simulink library "dkc"  (R2021b)
settings: Solver=VariableStepAuto  StartTime=0.0  StopTime=10.0  RelTol=1e-3
undefined symbols (not defined in the file): ENUM_ANTITHEFT_ALARM, ENUM_ANTITHEFT_ARM, ENUM_ANTITHEFT_DISARM, ENUM_ANTITHEFT_WAIT, ENUM_APSSTASYSTEM_DISABLE, ENUM_APSSTASYSTEM_ENABLE, ENUM_APSSTASYSTEM_REMOTEACTIVE, ENUM_BTCONNSTA_CONNECTED, ENUM_BTCONNSTA_DISCONNECTED, ENUM_DKCAuthSta_DECRYPTIONFAIL, ENUM_DKCAuthSta_NORMAL, ENUM_DKCAuthSta_TIMEERROR, ENUM_DKCPCMDHANDING_FORCELIFT, ENUM_DKCPCMDHANDING_LOCK, ENUM_DKCPCMDHANDING_LOCKTGATEFAIL, ENUM_DKCPCMDHANDING_OVER, ENUM_DKCPCMDHANDING_TGATEHANDLE, ENUM_DKCPCMDHANDING_UNLOCK, ENUM_DkeyShowIVI_DEFAULT, ENUM_DkeyShowIVI_INVALID, ENUM_DkeyShowIVI_NFCGREEN, ENUM_DkeyShowIVI_NFCRED, ENUM_GEARACTUALPOSN_N, ENUM_GEARACTUALPOSN_P, ENUM_KEYMISSSTA_DEFAULT, ENUM_KEYMISSSTA_KEYMISS, ENUM_KEYMODE_DAFAULT, ENUM_KEYMODE_INVALID, ENUM_KEYMODE_NFC, ENUM_KEYMODE_UIDBLE, ENUM_KEYMODE_UIDUWB, ENUM_KEYTYPE_NFC, ENUM_KEYTYPE_NOREQ, ENUM_KEYTYPE_UID, ENUM_PARKINGMODE_DISABLE, ENUM_PARKINGMODE_REMOTEFORWARD, ENUM_PARKINGMODE_REMOTEREVERSE, ENUM_PARKINGMODE_STANDBY, ENUM_PCMD_AUTOLOCKJUDGE, ENUM_PCMD_DEFAULT, ENUM_PCMD_NFCDETECT, ENUM_PCMD_PTGJUDGE, ENUM_PCMD_RSSIJUDGELOCK, ENUM_PCMD_TRUNKHAND, ENUM_PCMD_UIDBUTTON, ENUM_PCMD_UWBDETEDT, ENUM_PCMDTOBCM_DEFAULT, ENUM_PCMDTOBCM_FORCELIFT, ENUM_PCMDTOBCM_LOCK, ENUM_PCMDTOBCM_LOCKTGATEFAIL, ENUM_PCMDTOBCM_NFCCOMMAND, ENUM_PCMDTOBCM_REMOTETGATE, ENUM_PCMDTOBCM_TGATEHANDLE, ENUM_PCMDTOBCM_UNLOCK, ENUM_PCMDTOBCM_UWBLOCK, ENUM_PCMDTOBCM_UWBUNLOCK, ENUM_PDKEYPTGAREA_GRAYSPTGZONE, ENUM_PDKEYPTGAREA_PTGZONE, ENUM_PDKEYPTGAREA_SPTGZONE, ENUM_PDKEYPTGAREA_UNAVALIABLE ... (+126)
libraries: simulink x120, hcu_lib x6
(part 2 of 4)

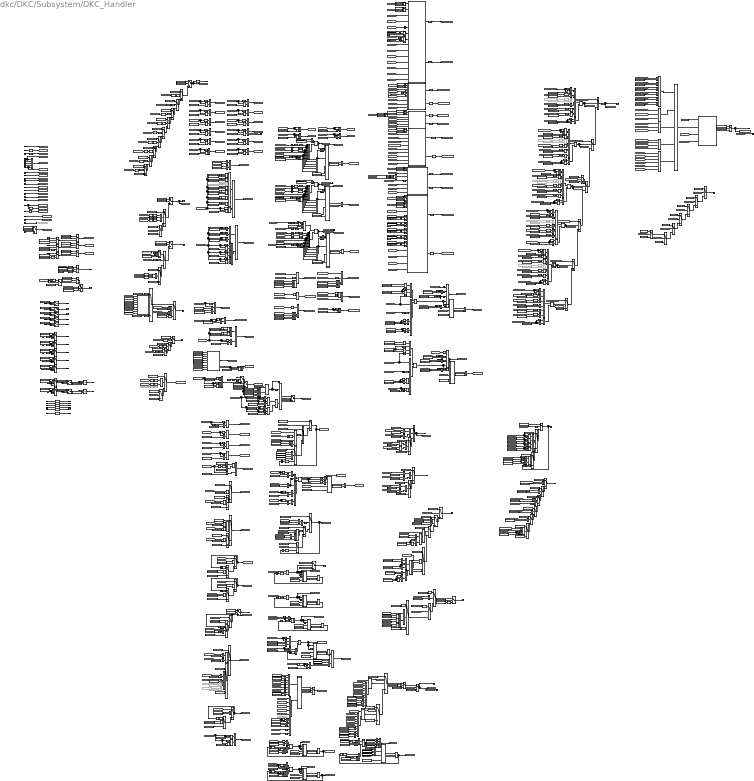
== system dkc/DKC/Subsystem/DKC_Handler ==
  note: % VINP_PDKeyAreaLockUnlock_enum(PE Zone)
      | ENUM_PDKEYRAWLULOCK_UNAVALIABLE = uint8( 0 );
      | ENUM_PDKEYRAWLULOCK_INLOCK = uint8( 1 );
      | ENUM_PDKEYRAWLULOCK_INUNLOCK = uint8( 2 );
      | ENUM_PDKEYRAWLULOCK_RESERVE = uint8( 3 );
      | ENUM_PDKEYRAWLULOCK_OTHERZONE = uint8( 255 );
  note: UWB Detect PDKey PEZone raw (沒有明確狀態一律給UNAVALIABLE)
  note: % VINP_PDKeyAreaLockUnlock_enum(PE Zone)
      | ENUM_PDKEYRAWLULOCK_UNAVALIABLE = uint8( 0 );
      | ENUM_PDKEYRAWLULOCK_INLOCK = uint8( 1 );
      | ENUM_PDKEYRAWLULOCK_INUNLOCK = uint8( 2 );
      | ENUM_PDKEYRAWLULOCK_RESERVE = uint8( 3 );
      | ENUM_PDKEYRAWLULOCK_OTHERZONE = uint8( 255 );
  note: VDKC_UWBXFPP_enum
      | DD File Define:s8
      | Valid Range:-127~127
      | Invalid value:128
  note: VINP_UWBXPower_dB
      | BSW Define:s8
      | Valid Range:-128~126
      | Invalid value:127(0x7F)
  note: VDKC_CoordinateX_enum
      | DD File Define:s16
      | Valid Range:-2550~2550
      | over range:2560(0x1FF)
      | INVALID:-2550(0x000)
  note: VDKC_UWB1Distance_enum
      | DD File Define:u16
      | Valid Range:0~2540
      | Invalid value:2550( 0xFF*10 )
  note: VINP_UWBxDistance_cm
      | BSW Define:u16
      | Valid Range:0~65534
      | Invalid value:65535(0xFFFF)
  note: KeyFobArea
      | KeyFobArea=0: unavailable
      |
      | Bit0 : PS Zone
      | Bit1 : Unlock Zone
      | Bit2 : Lock Zone
      |
      | Bit3 : SPTG Zone
      | Bit4 : PTG Zone
      | Bit5 : Welcome Zone
      | Bit6 : OutWelcome Zone
      | Bit7 : RKE Zone
      | Bit8 : GrayLockZone
      | Bit9 : GrayWelcomeZone
      | Bit10: GrayOutWelcomeZone
      | Bit11: GraySPTGZone
      |
      | 如過只舉PTG相關Flag
      | 輸出匯給出UNAVALIABLE
  note: KeyFobArea_flag change to KeyUWBDetPTGArea_enum
  note: 60s timeout
  note: Wait 60s standby judge
  note: Wait 60 s
  note: 5.5s timeout
  note: Wait 4S+1.5S USER Control Forward/Backward Req Judge
  note: Wait 4+1.5 s
  note: Wait 200ms APM-APS Req Judge
  note: Wait 200ms timeout
  note: UIDBLEButton Requireto RAPS Backward Release
  note: UIDBLEButton Requireto RAPS Forward Release
  note: UIDBLEButton Requireto RAPS Backward Press
  note: UIDBLEButton Requireto RAPS Forward Press
  note: UIDBLEButton Requireto RAPS Start Release
  note: UIDBLEButton Requireto RAPS Start Press
  note: KeyFobArea
      | KeyFobArea=0: unavailable
      | Bit0 : PS Zone
      | Bit1 : Unlock Zone
      | Bit2 : Lock Zone
      | Bit3 : SPTG Zone
      | Bit4 : PTG Zone
      | Bit5 : Welcome Zone
      | Bit6 : OutWelcome Zone
      | Bit7 : RKE Zone
      | Bit8 : GrayLockZone
      | Bit9 : GrayWelcomeZone
      | Bit10: GrayOutWelcomeZone
      | Bit11: GraySPTGZone
      |
      | 如過只舉PTG相關Flag
      | 輸出匯給出UNAVALIABLE
  note: KeyFobArea_flag change to PTGArea Debug
  note: UnavailabletoUnlock request door unlock
  note: RSSI Judge Lock trigger edge
  note: RSSI STRONG >>WEAK
  note: Key mode sta Judge
  note: Key Type Judge
  note: % VDKC_KeyModeSta_enum
      | ENUM_KEYMODE_DAFAULT = uint8( 0 );
      | ENUM_KEYMODE_UIDUWB = uint8( 1 );
      | ENUM_KEYMODE_UIDBLE = uint8( 2 );
      | ENUM_KEYMODE_PHONEUWB = uint8( 3 );
      | ENUM_KEYMODE_PHONEBLE = uint8( 4 );
      | ENUM_KEYMODE_NFC = uint8( 5 );
      | ENUM_KEYMODE_INVALID = uint8( 6 );
  note: % VDKC_FDCPCommandToBCM_enum
      | ENUM_PCMDTOBCM_DEFAULT = uint8( 0 );
      | ENUM_PCMDTOBCM_LOCK = uint8( 1 );
      | ENUM_PCMDTOBCM_UNLOCK = uint8( 2 );
      | ENUM_PCMDTOBCM_REMOTETGATE = uint8( 3 );
      | ENUM_PCMDTOBCM_CARSEARCH = uint8( 4 );
      | ENUM_PCMDTOBCM_LOCKTGATEFAIL = uint8( 5 );
      | ENUM_PCMDTOBCM_TGATEHANDLE = uint8( 6 );
      | ENUM_PCMDTOBCM_FORCELIFT = uint8( 7 );
      | ENUM_PCMDTOBCM_CARSEARCHMUTE = uint8( 8 );
      | ENUM_PCMDTOBCM_NFCCOMMAND = uint8( 9 );
      | ENUM_PCMDTOBCM_UWBLOCK = uint8( 10 );
      | ENUM_PCMDTOBCM_UWBUNLOCK = uint8( 11 );
      | ENUM_PCMDTOBCM_FRONTHOOD = uint8( 12 );
      | ENUM_PCMDTOBCM_CHARGECOVER = uint8( 13 );
      | ENUM_PCMDTOBCM_INVALID = uint8( 15 );
  note: % KDKC_BTConnectSta_enum_ovrdflg
      | % VDKC_BTConnectSta_enum
      | ENUM_BTCONNSTA_DISCONNECTED = uint8( 0 );
      | ENUM_BTCONNSTA_CONNECTED = uint8( 1 );
      | ENUM_BTCONNSTA_CONNECTING = uint8( 2 );
      | ENUM_BTCONNSTA_RESERVE = uint8( 3 );
  note: UID Battery Low Show in IVI
  note: % VDKC_UIDLowPowerSta_enum
      | ENUM_UIDLOWBATSTA_DEFAULT = uint8( 0 );
      | ENUM_UIDLOWBATSTA_LOWBATT = uint8( 1 );
  note: % KDKC_BTConnectSta_enum_ovrdflg
      | % VDKC_BTConnectSta_enum
      | ENUM_BTCONNSTA_DISCONNECTED = uint8( 0 );
      | ENUM_BTCONNSTA_CONNECTED = uint8( 1 );
      | ENUM_BTCONNSTA_CONNECTING = uint8( 2 );
      | ENUM_BTCONNSTA_RESERVE = uint8( 3 );
  note: PDKEY or NFC Card Judge Area in PS
  note: % VDKC_KeyMissSta_enum
      | ENUM_KEYMISSSTA_DEFAULT = uint8( 0 );
      | ENUM_KEYMISSSTA_KEYMISS = uint8( 1 );
  note: % VPMM_PowerSta_enum
      | ENUM_POWERSTA_OFF = uint8( 0 );
      | ENUM_POWERSTA_OFFC = uint8( 1 );
      | ENUM_POWERSTA_OFFA = uint8( 2 );
      | ENUM_POWERSTA_STANDBY = uint8( 3 );
      | ENUM_POWERSTA_ON = uint8( 4 );
      | ENUM_POWERSTA_READY = uint8( 5 );
  note: Fix the Bug of debounce in the DKC P-Command.
  note: WelcomeSta Latch
  note: KeyFobArea
      | KeyFobArea=0: unavailable
      | Bit0 : PS Zone
      | Bit1 : Unlock Zone
      | Bit2 : Lock Zone
      | Bit3 : SPTG Zone
      | Bit4 : PTG Zone
      | Bit5 : Welcome Zone
      | Bit6 : OutWelcome Zone
      | Bit7 : RKE Zone
      | Bit8 : GrayLockZone
      | Bit9 : GrayWelcomeZone
      | Bit10: GrayOutWelcomeZone
      | Bit11: GraySPTGZone
      |
      | 如過只舉PTG相關Flag
      | 輸出匯給出UNAVALIABLE
  note: % VDKC_FDCKeyAreaSPTG_enum
      | % VDKC_KeyAreaSPTGSta_enum
      | % KDKC_KeyUWBDetSPTGArea_enum_ovrdval
      | ENUM_PDKEYSPTGRAW_UNAVALIABLE = uint8( 0 );
      | ENUM_PDKEYSPTGRAW_INTOZONE = uint8( 1 );
      | ENUM_PDKEYSPTGRAW_OUTZONE = uint8( 2 );
      | ENUM_PDKEYSPTGRAW_RESERVE = uint8( 3 );
  note: KeyFobArea_flag change to KeyUWBDetSPTGArea_enum
  note: KeyFobArea
      | KeyFobArea=0: unavailable
      | Bit0 : PS Zone
      | Bit1 : Unlock Zone
      | Bit2 : Lock Zone
      | Bit3 : SPTG Zone
      | Bit4 : PTG Zone
      | Bit5 : Welcome Zone
      | Bit6 : OutWelcome Zone
      | Bit7 : RKE Zone
      | Bit8 : GrayLockZone
      | Bit9 : GrayWelcomeZone
      | Bit10: GrayOutWelcomeZone
      | Bit11: GraySPTGZone
      |
      | 如過只舉PTG相關Flag
      | 輸出匯給出UNAVALIABLE
  note: 5m
  note: KeyFobArea
      | KeyFobArea=0: unavailable
      | Bit0 : PS Zone
      | Bit1 : Unlock Zone
      | Bit2 : Lock Zone
      | Bit3 : SPTG Zone
      | Bit4 : PTG Zone
      | Bit5 : OutPTG Zone
      | Bit6 : Welcome Zone
      | Bit7 : OutWelcome Zone
      | Bit8 : RKE Zone
      | Bit9 : InitDetLockZone (GrayLockZone)
      | Bit10: InitDetWelcomeZone(GrayWelcomeZone)
      | Bit11: InitDetOutWelcomeZone(GrayOutWelcomeZone
  note: PMM change to ready if( Antif==ARM ) , PCmd==FORCELIFT
  note: If the remote app lock during the auto-lock period,the next auto-lock will fail.
  note: If the remote app lock during the auto-lock period,the next auto-lock will fail.
  note: RemoteTG command Rising Judge
  note: Priority4-TrunkHandPCmd
  note: Priority2-TrunkHandPCmd
  note: TRUNKHANSW_PRESS Judge
  note: UIDBLEButton Requireto CHARGECOVER
  note: UIDBLEButton Requireto FRONTHOOD
  note: % VDKC_FDCKeyAreaPTG_enum
      | % VINP_PDKeyAreaPTG_enum
      | % VDKC_KeyAreaPTG_enum
      | % KDKC_KeyUWBDetPTGArea_enum_ovrdval
      | ENUM_PDKEYPTGRAW_UNAVALIABLE = uint8( 0 );
      | ENUM_PDKEYPTGRAW_INTOZONE = uint8( 1 );
      | ENUM_PDKEYPTGRAW_OUTZONE = uint8( 2 );
      | ENUM_PDKEYPTGRAW_RESERVE = uint8( 3 );
  note: KeyFobArea_flag change to KeyUWBDetPTGArea_enum
  note: % KINP_UIDButtonCmd_enum_ovrdval
      | % VHAL_UIDButtonCmd_enum
      | % VINP_UIDButtonCmd_enum
      | ENUM_UIDBUTTON_UNAVALIABLE = uint8( 0 );
      | ENUM_UIDBUTTON_UNLOCK = uint8( 1 );
      | ENUM_UIDBUTTON_LOCK = uint8( 2 );
      | ENUM_UIDBUTTON_FRONTHOOD = uint8( 3 );
      | ENUM_UIDBUTTON_REMOTETAILGATE = uint8( 4 );
      | ENUM_UIDBUTTON_CHARGECOVER = uint8( 5 );
      | ENUM_UIDBUTTON_CARSEARCH = uint8( 6 );
      | ENUM_UIDBUTTON_RAPSSTARTPRESS = uint8( 7 );
      | ENUM_UIDBUTTON_RAPSFORWARDPRESS = uint8( 8 );
      | ENUM_UIDBUTTON_RAPSBACKWARDPRESS = uint8( 9 );
      | ENUM_UIDBUTTON_RAPSSTARTRELEASE = uint8( 10 );
      | ENUM_UIDBUTTON_RAPSFORWARDRELEASE = uint8( 11 );
      | ENUM_UIDBUTTON_RAPSBACKWARRELEASE = uint8( 12 );
  note: UIDBLEButton Requireto CARSEARCH
  note: UIDBLEButton Requireto REMOTETAILGATE
  note: % VDKC_KeyUWBDetArea_enum
      | % KDKC_KeyUWBDetArea_enum_ovrdval
      | ENUM_UWBDET_UNAVALIABLE = uint8( 0 );
      | ENUM_UWBDET_PSZONE = uint8( 1 );
      | ENUM_UWBDET_UNLOCKZONE = uint8( 2 );
      | ENUM_UWBDET_LOCKZONE = uint8( 3 );
      | ENUM_UWBDET_WELCOMEZONE = uint8( 4 );
      | ENUM_UWBDET_OUTWELCOMEZONE = uint8( 5 );
      | ENUM_UWBDET_RKEZONE = uint8( 6 );
      | ENUM_UWBDET_GRAYLOCKZONE = uint8( 7 );
      | ENUM_UWBDET_GRAYWELCOMEZONE = uint8( 8 );
      | ENUM_UWBDET_GRAYOUTWELCOMEZONE = uint8( 9 );
  note: % VINP_PDKeyAreaLockUnlock_enum
      | ENUM_PDKEYRAWLULOCK_UNAVALIABLE = uint8( 0 );
      | ENUM_PDKEYRAWLULOCK_INLOCK = uint8( 1 );
      | ENUM_PDKEYRAWLULOCK_INUNLOCK = uint8( 2 );
      | ENUM_PDKEYRAWLULOCK_RESERVE = uint8( 3 );
  note: % VINP_PDKeyAreaPS_enum(PS Zone)
      | ENUM_PDKEYRAWPS_UNAVALIABLE = uint8( 0 );
      | ENUM_PDKEYRAWPS_INPS = uint8( 1 );
      | ENUM_PDKEYRAWPS_OUTPS = uint8( 2 );
      | ENUM_PDKEYRAWPS_RESERVE = uint8( 3 );
  note: UIDButton change Antitheft state to DISARM
  note: UIDButton AutoLock Judge
  note: UWB Within unLock Zone(3m) Judge(需為明確的unlock zone)
  note: Priority1-UIDButton PCmd
  note: UIDBLEButton Requireto Unlock
  note: UIDBLEButton Requireto Lock
  note: Arbitration Det Area PE Zone
  note: UWB Detect PDKey PEZone raw (沒有明確狀態一律給UNAVALIABLE)
  note: NFCKeyArea change to non-PS zone
  note: Priority3-NFC Detect PCmd
  note: UWB_Detect_PDKey Require to Lock
  note: UWB_Detect_PDKey Require to unLock
  note: NFC change Antitheft state to DISARM
  note: NFCKeyArea change to PS zone
  note: KeyArea change to non-PS zone
  note: UWB Detect PDKey PSZone raw
  note: Power state change from READY or ON to Standby
  note: Power state change to OFFC
  note: Power state change to OFFA
  note: Power state "LEAVE" from READY
  note: Power state change to OFF
  note: Priority6-UWB Detect PCmd
  note: Detect PCommand set Default
  note: NFCJudge_PS_Area
  note: NFCJudgePEZoneSta
  note: % VINP_PDKeyAreaPS_enum(PS Zone)
      | ENUM_PDKEYRAWPS_UNAVALIABLE = uint8( 0 );
      | ENUM_PDKEYRAWPS_INPS = uint8( 1 );
      | ENUM_PDKEYRAWPS_OUTPS = uint8( 2 );
      | ENUM_PDKEYRAWPS_RESERVE = uint8( 3 );
  note: Arbitration Det Area PS Zone
  note: % VINP_PDKeyAreaLockUnlock_enum
      | ENUM_PDKEYRAWLULOCK_UNAVALIABLE = uint8( 0 );
      | ENUM_PDKEYRAWLULOCK_INLOCK = uint8( 1 );
      | ENUM_PDKEYRAWLULOCK_INUNLOCK = uint8( 2 );
      | ENUM_PDKEYRAWLULOCK_RESERVE = uint8( 3 );
  note: % VINP_PDKeyAreaLockUnlock_enum(PE Zone)
      | ENUM_PDKEYRAWLULOCK_UNAVALIABLE = uint8( 0 );
      | ENUM_PDKEYRAWLULOCK_INLOCK = uint8( 1 );
      | ENUM_PDKEYRAWLULOCK_INUNLOCK = uint8( 2 );
      | ENUM_PDKEYRAWLULOCK_RESERVE = uint8( 3 );
  note: Arbitration PCmdtoBCM
  note: Priority5-AutoLock Judge PCmd
  note: NFC AutoLock Judge
  note: % VDKC_KeyUWBDetArea_enum
      | % KDKC_KeyUWBDetArea_enum_ovrdval
      | ENUM_UWBDET_UNAVALIABLE = uint8( 0 );
      | ENUM_UWBDET_PSZONE = uint8( 1 );
      | ENUM_UWBDET_UNLOCKZONE = uint8( 2 );
      | ENUM_UWBDET_LOCKZONE = uint8( 3 );
      | ENUM_UWBDET_WELCOMEZONE = uint8( 4 );
      | ENUM_UWBDET_OUTWELCOMEZONE = uint8( 5 );
      | ENUM_UWBDET_RKEZONE = uint8( 6 );
      | ENUM_UWBDET_GRAYLOCKZONE = uint8( 7 );
      | ENUM_UWBDET_GRAYWELCOMEZONE = uint8( 8 );
      | ENUM_UWBDET_GRAYOUTWELCOMEZONE = uint8( 9 );
  note: % VTQD_GearActualPosn_enum
      | ENUM_GEARACTUALPOSN_P = uint8( 1 );
      | ENUM_GEARACTUALPOSN_R = uint8( 2 );
      | ENUM_GEARACTUALPOSN_N = uint8( 3 );
      | ENUM_GEARACTUALPOSN_D = uint8( 4 );
      | ENUM_GEARACTUALPOSN_INVALID = uint8( 0 );
  note: % VINP_UIDButtonCmd_enum
      | ENUM_UIDBUTTON_UNAVALIABLE = uint8( 0 );
      | ENUM_UIDBUTTON_UNLOCK = uint8( 1 );
      | ENUM_UIDBUTTON_LOCK = uint8( 2 );
      | ENUM_UIDBUTTON_FRONTHOOD = uint8( 3 );
      | ENUM_UIDBUTTON_REMOTETAILGATE = uint8( 4 );
      | ENUM_UIDBUTTON_CHARGECOVER = uint8( 5 );
      | ENUM_UIDBUTTON_CARSEARCH = uint8( 6 );
  note: KeyFobArea_flag change to KeyUWBDetArea_enum
  note: PTG InnerSW Close TimerOut Count Function
  note: TailgateSW2 FallingEdge to close and Dectect UID in PS Zone
  note: TailgateSW2 FallingEdge to close and Dectect UID out PS Zone
  note: Press InnerSW2 after TailgateSW No Close
  note: FallingEdge to close and Dectect UID in PS Zone
  note: Press InnerSW1 or DKC remtailgate Button after TailgateSW No Close
  note: KeyFobArea
      | KeyFobArea=0: unavailable
      | Bit0 : PS Zone
      | Bit1 : Unlock Zone
      | Bit2 : Lock Zone
      | Bit3 : SPTG Zone
      | Bit4 : PTG Zone
      | Bit5 : Welcome Zone
      | Bit6 : OutWelcome Zone
      | Bit7 : RKE Zone
      | Bit8 : GrayLockZone
      | Bit9 : GrayWelcomeZone
      | Bit10: GrayOutWelcomeZone
      | Bit11: GraySPTGZone
      |
      | 如過只舉PTG相關Flag
      | 輸出匯給出UNAVALIABLE
  note: % VDKC_KeyUWBDetArea_enum
      | % KDKC_KeyUWBDetArea_enum_ovrdval
      | ENUM_UWBDET_UNAVALIABLE = uint8( 0 );
      | ENUM_UWBDET_PSZONE = uint8( 1 );
      | ENUM_UWBDET_UNLOCKZONE = uint8( 2 );
      | ENUM_UWBDET_LOCKZONE = uint8( 3 );
      | ENUM_UWBDET_WELCOMEZONE = uint8( 4 );
      | ENUM_UWBDET_OUTWELCOMEZONE = uint8( 5 );
      | ENUM_UWBDET_RKEZONE = uint8( 6 );
      | ENUM_UWBDET_GRAYLOCKZONE = uint8( 7 );
      | ENUM_UWBDET_GRAYWELCOMEZONE = uint8( 8 );
      | ENUM_UWBDET_GRAYOUTWELCOMEZONE = uint8( 9 );
  note: 8m
  note: 10m
  note: 3m
  note: 3-5m
  note: % VDKC_KeyUWBDetArea_enum
      | % KDKC_KeyUWBDetArea_enum_ovrdval
      | ENUM_UWBDET_UNAVALIABLE = uint8( 0 );
      | ENUM_UWBDET_PSZONE = uint8( 1 );
      | ENUM_UWBDET_UNLOCKZONE = uint8( 2 );
      | ENUM_UWBDET_LOCKZONE = uint8( 3 );
      | ENUM_UWBDET_WELCOMEZONE = uint8( 4 );
      | ENUM_UWBDET_OUTWELCOMEZONE = uint8( 5 );
      | ENUM_UWBDET_RKEZONE = uint8( 6 );
      | ENUM_UWBDET_GRAYLOCKZONE = uint8( 7 );
      | ENUM_UWBDET_GRAYWELCOMEZONE = uint8( 8 );
      | ENUM_UWBDET_GRAYOUTWELCOMEZONE = uint8( 9 );
  note: % VDKC_KeyUWBDetArea_enum
      | % KDKC_KeyUWBDetArea_enum_ovrdval
      | ENUM_UWBDET_UNAVALIABLE = uint8( 0 );
      | ENUM_UWBDET_PSZONE = uint8( 1 );
      | ENUM_UWBDET_UNLOCKZONE = uint8( 2 );
      | ENUM_UWBDET_LOCKZONE = uint8( 3 );
      | ENUM_UWBDET_WELCOMEZONE = uint8( 4 );
      | ENUM_UWBDET_OUTWELCOMEZONE = uint8( 5 );
      | ENUM_UWBDET_RKEZONE = uint8( 6 );
      | ENUM_UWBDET_GRAYLOCKZONE = uint8( 7 );
      | ENUM_UWBDET_GRAYWELCOMEZONE = uint8( 8 );
      | ENUM_UWBDET_GRAYOUTWELCOMEZONE = uint8( 9 );
  note: NFC Unlock/lock PCMD Change to NFC-CMD
  note: % VDKC_KeyUWBDetArea_enum
      | % KDKC_KeyUWBDetArea_enum_ovrdval
      | ENUM_UWBDET_UNAVALIABLE = uint8( 0 );
      | ENUM_UWBDET_PSZONE = uint8( 1 );
      | ENUM_UWBDET_UNLOCKZONE = uint8( 2 );
      | ENUM_UWBDET_LOCKZONE = uint8( 3 );
      | ENUM_UWBDET_WELCOMEZONE = uint8( 4 );
      | ENUM_UWBDET_OUTWELCOMEZONE = uint8( 5 );
      | ENUM_UWBDET_RKEZONE = uint8( 6 );
      | ENUM_UWBDET_GRAYLOCKZONE = uint8( 7 );
      | ENUM_UWBDET_GRAYWELCOMEZONE = uint8( 8 );
      | ENUM_UWBDET_GRAYOUTWELCOMEZONE = uint8( 9 );
  note: UWB_Detect_PDKey Require to Welcome mode
  note: LIDA -Green Latch
  note: in unlockZone and unlock during not counter timeout trigger
  note: in unlockZone and unlock during not counter timeout trigger
  note: trigger==0&& reset==1 timer counter=Reset(0)
  note: trigger==0&& reset==1 timer counter=Reset(0)
  note: NFCJudge Auto Leave PS
  note: DKC Allow Sleep Judge
  note: Keep PE,PS Zone State
  note: % KDKC_BTConnectSta_enum_ovrdflg
      | ENUM_BTConnSta_DISCONNECTED = uint8( 0 );
      | ENUM_BTConnSta_CONNECTED = uint8( 1 );
      | ENUM_BTConnSta_CONNECTING = uint8( 2 );
      | ENUM_BTConnSta_RESERVE = uint8( 3 );
  note: on Ready BT Disconnect 10s(key miss Judge)
  note: NFCKeyArea change to PS zone
  note: % VDKC_KeyTypeSta_enum
      | ENUM_KEYTYPE_NOREQ = uint8( 0 );
      | ENUM_KEYTYPE_UID = uint8( 1 );
      | ENUM_KEYTYPE_NFC = uint8( 2 );
      | ENUM_KEYTYPE_PHONE = uint8( 3 );
  note: Antitheft change to ARM
  note: Antitheft change to ARM
  note: NFC change Antitheft state to DISARM
  note: IVI Show NFC Card STA Judge
  note: DrDoor Sta Judge Latch
  note: RSSI_dBm:1Byte
      | Type:s8[-128~127]
      | (0~-100dB) range
      | Initial value:-128
      | Valid Range:0~-100
      | Other Invalid:1~127,-101~-12
  note: % KDKC_BTRSSISampTime_s=init 100ms
  note: BT RSSI Judge UID Area
  note: RSSI_dBm:1Byte
      | Type:s8[-128~127]
      | (0~-100dB) range
      | Initial value:-128
      | Valid Range:0~-100
      | Other Invalid:1~127,-101~-12
      | % VDKC_RSSIJudgeArea_enum
      | ENUM_RSSIAREA_DAFAULT = uint8( 0 );
      | ENUM_RSSIAREA_WEAK = uint8( 1 );
      | ENUM_RSSIAreaSta_STRONG = uint8( 2 );
  note: Judge Unlock Zone Falling edge flg
  note: % VDKC_KeyUWBDetArea_enum
      | % KDKC_KeyUWBDetArea_enum_ovrdval
      | ENUM_UWBDET_UNAVALIABLE = uint8( 0 );
      | ENUM_UWBDET_PSZONE = uint8( 1 );
      | ENUM_UWBDET_UNLOCKZONE = uint8( 2 );
      | ENUM_UWBDET_LOCKZONE = uint8( 3 );
      | ENUM_UWBDET_WELCOMEZONE = uint8( 4 );
      | ENUM_UWBDET_OUTWELCOMEZONE = uint8( 5 );
      | ENUM_UWBDET_RKEZONE = uint8( 6 );
      | ENUM_UWBDET_GRAYLOCKZONE = uint8( 7 );
      | ENUM_UWBDET_GRAYWELCOMEZONE = uint8( 8 );
      | ENUM_UWBDET_GRAYOUTWELCOMEZONE = uint8( 9 );
  note: PCMD_Debug output
  note: % VDKC_RSSISignal_enum
      | ENUM_RSSI_MAX = uint8( 0 );
      | ENUM_RSSI_UNAVAILABLE = uint8( 255 );
  note: % VDKC_UWBDetPTGArea_enum
      | ENUM_PDKEYPTGAREA_UNAVALIABLE = uint8( 0 );
      | ENUM_PDKEYPTGAREA_SPTGZONE = uint8( 1 );
      | ENUM_PDKEYPTGAREA_PTGZONE = uint8( 2 );
      | ENUM_PDKEYPTGAREA_GraySPTGZone = uint8( 3 );
  note: RAPS Active flg
  note: ACC>1.5% =0
      | ACC<1.5% =1
  note: ACC=Active flg=1
      | ACC=OFF flg=0
  note: % VINP_APSStaSystem_enum
      | % VAPS_APSStaSystem_enum
      | ENUM_APSSTASYSTEM_DISABLE = uint8( 0 );
      | ENUM_APSSTASYSTEM_ENABLE = uint8( 1 );
      | ENUM_APSSTASYSTEM_ACTIVE = uint8( 2 );
      | ENUM_APSSTASYSTEM_FAILED = uint8( 3 );
      | ENUM_APSSTASYSTEM_REMOTEACTIVE = uint8( 4 );
  note: % VINP_APSStaSystem_enum
      | % VAPS_APSStaSystem_enum
      | ENUM_APSSTASYSTEM_DISABLE = uint8( 0 );
      | ENUM_APSSTASYSTEM_ENABLE = uint8( 1 );
      | ENUM_APSSTASYSTEM_ACTIVE = uint8( 2 );
      | ENUM_APSSTASYSTEM_FAILED = uint8( 3 );
      | ENUM_APSSTASYSTEM_REMOTEACTIVE = uint8( 4 );
  note: 200s timeout
  note: % VDKC_FDCDKCParkingMode_enum
      | ENUM_PARKINGMODE_DISABLE = uint8( 0 );
      | ENUM_PARKINGMODE_STANDBY = uint8( 1 );
      | ENUM_PARKINGMODE_REMOTEPARKING = uint8( 2 );
      | ENUM_PARKINGMODE_REMOTEFORWARD = uint8( 3 );
      | ENUM_PARKINGMODE_REMOTEREVERSE = uint8( 4 );
  note: DKC Judge Output ParkingMode
  note: % VDKC_DkeyAreaRAPSSta_enum
      | % KDKC_KeyUWBDetRAPSArea_enum_ovrdval
      | ENUM_PDKEYRAPSRAW_UNAVALIABLE = uint8( 0 );
      | ENUM_PDKEYRAPSRAW_INTOZONE = uint8( 1 );
      | ENUM_PDKEYRAPSRAW_OUTZONE = uint8( 2 );
  note: RAPS Detect zone keep judge
  note: % VINP_UWBxDistance_cm
      | ENUM_UWBXDISTANCE_ONCANINVALID = uint16( 2550 );
      | % VINP_UWB1Power_dB
      | ENUM_UWBPOWER_BSWINVALID = int16( 127 );
      | % VDKC_UWBXFPP_enum
      | ENUM_UWBPOWER_ONCANINVALID = int16( 128 );
      | % VINP_UWBpositionX_cm
      | ENUM_UWBPOSX_BSWINVALID = int16( 32767 );
      | % VDKC_CoordinateX_enum
      | ENUM_UWBPOSX_ONCANINVALID = int16( -2550 );
      | ENUM_UWBPOSX_ONCANEXRANGE = int16( 2560 );
      | % VINP_UWBpositionY_cm
      | ENUM_UWBPOSY_ONCANINVALID = int16( 0 );
      | ENUM_UWBPOSY_BSWINVALID = int16( 32767 );
      | ENUM_UWBPOSY_ONCANEXRANGE = int16( -2560 );
  note: UWBxDistance
  note: UWB1Power
  note: % VINP_UWB5RangingSta_enum
      | % VDKC_UWB5Invalid_flg
      | % KINP_UWB5RangingSta_enum_ovrdval
      | ENUM_UWBRANGINGSTA_VALID = uint8( 0 );
      | ENUM_UWBRANGINGSTA_INVALID = uint8( 1 );
      | ENUM_UWBRANGINGSTA_BROKEN = uint8( 2 );
      | ENUM_UWBRANGINGSTA_NOUSED = uint8( 3 );
  note: UWBpositionX/Y
  note: UWB OTHER
  note: Keep Detect unlock area
  note: keep unlockzone to otherzone Judge lock
  task_time_s : Inport
  VINP_NFCLidASta_flg : Inport  Port=2
  VINP_NFCDoorSta_flg : Inport  Port=3
  VINP_DrDoorSW_flg : Inport  Port=4
  VINP_PsDoorSW_flg : Inport  Port=5
  VINP_RRDoorSW_flg : Inport  Port=6
  VINP_RLDoorSW_flg : Inport  Port=7
  VINP_TailgateSW_flg : Inport  Port=8
  VINP_HoodSW_flg : Inport  Port=9
  VBCM_AntitheftSta_enum : Inport  Port=10
  VPMM_PowerSta_enum : Inport  Port=11
  VINP_KeyFobAreaU16_enum : Inport  Port=12
  VINP_UIDButtonCmd_enum : Inport  Port=13
  VINP_VehSpeed_kph : Inport  Port=14
  VTQD_GearActualPosn_enum : Inport  Port=15
  VINP_TrunkHanSW_flg : Inport  Port=16
  VINP_BPPTGInsideSW1Sta_enum : Inport  Port=17
  VINP_BPPTGInsideSW2Sta_enum : Inport  Port=18
  VINP_BrakeSWGPIO_flg : Inport  Port=19
  VTQD_LowIdleAccPedal_flg : Inport  Port=20
  VDKC_CANMsgValidZONEDRFR_flg : Inport  Port=21
  VINP_SeatSW_flg : Inport  Port=22
  VINP_BTConnectSta_enum : Inport  Port=23
  VINP_UIDBatVoltx1000_V : Inport  Port=24
  VINP_DKCBTRSSI_dB : Inport  Port=25
  VINP_FlashJugKeepUnLZone_flg : Inport  Port=26
  VINP_BPPTGExistSta_flg : Inport  Port=27
  VINP_APSStaSystem_enum : Inport  Port=28
  VINP_UWB1Distance_cm : Inport  Port=29
  VINP_UWB2Distance_cm : Inport  Port=30
  VINP_UWB3Distance_cm : Inport  Port=31
  VINP_UWB4Distance_cm : Inport  Port=32
  VINP_UWB5Distance_cm : Inport  Port=33
  VINP_UWB1Power_dB : Inport  Port=34
  VINP_UWB2Power_dB : Inport  Port=35
  VINP_UWB3Power_dB : Inport  Port=36
  VINP_UWB4Power_dB : Inport  Port=37
  VINP_UWB5Power_dB : Inport  Port=38
  VINP_UWBpositionX_cm : Inport  Port=39
  VINP_UWBpositionY_cm : Inport  Port=40
  VINP_UWB1RangingSta_enum : Inport  Port=41
  VINP_UWB2RangingSta_enum : Inport  Port=42
  VINP_UWB3RangingSta_enum : Inport  Port=43
  VINP_UWB4RangingSta_enum : Inport  Port=44
  VINP_UWB5RangingSta_enum : Inport  Port=45
  VINP_UWBRangingON_flg : Inport  Port=46
  Abs : Abs
  AllowSleep_Chart : Stateflow chart  TreatAsAtomicUnit=on
  AutoLock_PCMD_Chart : Stateflow chart  TreatAsAtomicUnit=on
  BTRSSIJudgeArea_Chart : Stateflow chart  TreatAsAtomicUnit=on
  Constant : Constant  Value=ENUM_BTCONNSTA_DISCONNECTED  OutDataTypeStr=uint8
  Constant{1,16,136,138,165,304..305,313,316,417} (10 alike) : Constant  Value=ENUM_UWBDET_UNLOCKZONE
  Constant10 : Constant  Value=ENUM_TRUNKHANSW_RELEASE
  Constant{35,100..101,140} (4 alike) : Constant  Value=KDKC_UnlockCmdDelayTime_s
  Constant102 : Constant  Value=ENUM_UIDBUTTON_LOCK
  Constant{57..59,63..68,72..78,103,108,110..113,142,146,149,196,216..220} (31 alike) : Constant  Value=ENUM_DKCPCMDHANDING_OVER
  Constant{60..61,69..70,98,104..105,144..145,147..148,151,153,178,201,261,264..265,271,274,277,279,281,283,285} (25 alike) : Constant  Value=ENUM_PCMDTOBCM_DEFAULT
  Constant{106,159,202..203,205..207,211..212} (9 alike) : Constant  Value=KDKC_ZONEVaildCmdDelayTime_s
  Constant{62,71,107,109,114} (5 alike) : Constant  Commented=on  Value=ENUM_DKCPCMDHANDING_OVER
  Constant11 : Constant  Value=ENUM_PDKEYPTGRAW_INTOZONE
  Constant{3..4,115..116} (4 alike) : Constant  Value=KDKC_AutoLockTimeout_s
  Constant117 : Constant  Value=KDKC_PSAreaTimeout_s
  Constant{44,47,81,92,99,118,128,150,154..156,191,210,241,246,268..269,272,392} (19 alike) : Constant  Value=ENUM_PDKEYRAWPS_INPS
  Constant119 : Constant  Value=KDKC_PSAreaTimeout_s
  Constant12 : Constant  Value=ENUM_PDKEYPTGRAW_UNAVALIABLE
  Constant{55,87,120,226..228,288,306,314,380..381,424} (12 alike) : Constant  Value=ENUM_UWBDET_UNAVALIABLE
  Constant{121,157,160..162} (5 alike) : Constant  Value=ENUM_PDKEYRAWPS_OUTPS
  Constant{82..84,122,129,152,244,263} (8 alike) : Constant  Value=ENUM_POWERSTA_READY
  Constant123 : Constant  Value=ENUM_ANTITHEFT_DISARM
  Constant124 : Constant  Value=ENUM_POWERSTA_OFFC
  Constant125 : Constant  Value=ENUM_POWERSTA_OFF
  Constant{6,8..9,53,56,91,126,197..198,209} (10 alike) : Constant  Value=ENUM_PCMDTOBCM_UNLOCK
  Constant{46,127,158,163..164,170,177,391,393,418} (10 alike) : Constant  Value=ENUM_PDKEYRAWPS_UNAVALIABLE
  Constant13 : Constant  Value=ENUM_UIDBUTTON_REMOTETAILGATE
  Constant130 : Constant  Value=KDKC_LatchWelcomeModeSta_s
  Constant{23,131,134,180} (4 alike) : Constant  Value=ENUM_UWBDET_WELCOMEZONE
  Constant132 : Constant  Value=ENUM_UWBDET_GRAYOUTWELCOMEZONE
  Constant133 : Constant  Commented=on  Value=ENUM_UWBDET_GRAYLOCKZONE
  Constant135 : Constant  Value=ENUM_POWERSTA_STANDBY
  Constant{2,15,97,137,175,422} (6 alike) : Constant  Value=ENUM_UWBDET_PSZONE
  Constant{22,139,166,181} (4 alike) : Constant  Value=ENUM_UWBDET_LOCKZONE
  Constant14 : Constant  Value=ENUM_UIDBUTTON_CARSEARCH
  Constant{48,54,141,199,204} (5 alike) : Constant  Value=KDKC_LockCmdDelayTime_s
  Constant143 : Constant  Value=ENUM_POWERSTA_ON
  Constant{94,167..168,171..172,419,423} (7 alike) : Constant  Value=ENUM_PDKEYRAWLULOCK_INUNLOCK
  Constant{95,169,173..174,176} (5 alike) : Constant  Value=ENUM_PDKEYRAWLULOCK_INLOCK
  Constant17 : Constant  Value=ENUM_PDKEYSPTGRAW_UNAVALIABLE
  Constant179 : Constant  Value=ENUM_UIDBUTTON_UNLOCK
  Constant18 : Constant  Value=ENUM_PDKEYSPTGRAW_INTOZONE
  Constant182 : Constant  Value=ENUM_UWBDET_GRAYWELCOMEZONE
  Constant{25,183,308,315,426} (5 alike) : Constant  Value=ENUM_UWBDET_GRAYLOCKZONE
  Constant{7,24,90,184} (4 alike) : Constant  Value=ENUM_UWBDET_OUTWELCOMEZONE
  Constant185 : Constant  Value=ENUM_PDKEYWELCOMERAW_UNAVALIABLE
  Constant186 : Constant  Value=ENUM_PDKEYWELCOMERAW_INTOZONE
  Constant187 : Constant  Value=ENUM_UWBDET_GRAYOUTWELCOMEZONE
  Constant188 : Constant  Value=KDKC_LatchWelcomeModeSta_s
  Constant189 : Constant  Value=KDKC_LatchLidADetGreenCard_s
  Constant19 : Constant  Value=ENUM_PDKEYSPTGRAW_OUTZONE
  Constant190 : Constant  Value=ENUM_DkeyShowIVI_NFCGREEN
  Constant192 : Constant  Value=KDKC_LatchLidADetGreenCard_s
  Constant193 : Constant  Value=ENUM_DkeyShowIVI_DEFAULT
  Constant194 : Constant  Value=ENUM_DkeyShowIVI_NFCRED
  Constant{79..80,195,213} (4 alike) : Constant  Value=ENUM_ANTITHEFT_ARM
  Constant20 : Constant  Value=KDKC_KeyUWBDetSPTGArea_enum_ovrdflg
  Constant200 : Constant  Value=ENUM_PCMDTOBCM_NFCCOMMAND
  Constant208 : Constant  Value=ENUM_ANTITHEFT_DISARM
  Constant21 : Constant  Value=KDKC_KeyUWBDetSPTGArea_enum_ovrdval
  Constant214 : Constant  Value=ENUM_DkeyShowIVI_INVALID
  Constant215 : Constant  Value=ENUM_DkeyShowIVI_DEFAULT
  Constant221 : Constant  Value=KDKC_FDCKeyAllowSleep_flg_ovrdflg
  Constant222 : Constant  Value=KDKC_FDCKeyAllowSleep_flg_ovrdval
  Constant{51,223,251,262,335,349,382,425} (8 alike) : Constant  Value=ENUM_BTCONNSTA_CONNECTED
  Constant{40,50,52,224} (4 alike) : Constant  Value=ENUM_PCMDTOBCM_REMOTETGATE
  Constant225 : Constant  Value=KDKC_DKCAllowSleepDelayTime_s
  Constant229 : Constant  Value=KDKC_BTConnectSta_enum_ovrdflg
  Constant230 : Constant  Value=KDKC_BTConnectSta_enum_ovrdval
  Constant{231,318..319,337,353,383..386} (9 alike) : Constant  Value=FALSE
  Constant233 : Constant  Value=ENUM_KEYMISSSTA_KEYMISS
  Constant235 : Constant  Value=ENUM_POWERSTA_ON
  Constant236 : Constant  Value=ENUM_POWERSTA_STANDBY
  Constant237 : Constant  Value=ENUM_POWERSTA_OFFC
  Constant238 : Constant  Value=ENUM_KEYMISSSTA_DEFAULT
  Constant239 : Constant  Value=KDKC_BTDisconJudgeDeb_s
  Constant240 : Constant  Value=KDKC_BTDisconJudgeDeb_s
  Constant242 : Constant  Value=ENUM_KEYMISSSTA_DEFAULT
  Constant{243,347,360,362} (4 alike) : Constant  Value=ENUM_BTCONNSTA_DISCONNECTED
  Constant245 : Constant  Value=ENUM_KEYMISSSTA_KEYMISS
  Constant247 : Constant  Value=KDKC_UIDBTStaBSWInpSW_ovrdflg
  Constant248 : Constant  Value=KDKC_UIDBatVoltx1000_V_ovrdflg
  Constant249 : Constant  Value=KDKC_UIDBatVoltx1000_V_ovrdval
  Constant250 : Constant  Value=ENUM_POWERSTA_OFF
  Constant252 : Constant  Value=ENUM_UIDLOWBATSTA_DEFAULT
  Constant253 : Constant  Value=ENUM_UIDLOWBATSTA_DEFAULT
  Constant254 : Constant  Value=ENUM_UIDLOWBATSTA_LOWBATT
  Constant255 : Constant  Value=KDKC_UIDBatLowVolDeb_cnt
  Constant256 : Constant  Value=KDKC_UIDBatOKVolDeb_cnt
  Constant257 : Constant  Value=KDKC_UIDBatSampInterval_s
  Constant258 : Constant  Value=KDKC_UIDBatSampTotal_cnt
  Constant259 : Constant  Value=KDKC_UIDBatLowVolx1000Thres_V
  Constant26 : Constant  Value=ENUM_PDKEYPTGRAW_INTOZONE
  Constant260 : Constant  Value=KDKC_UIDBatOKVolx1000Thres_V
  Constant266 : Constant  Value=ENUM_KEYTYPE_NOREQ
  Constant267 : Constant  Value=ENUM_KEYTYPE_UID
  Constant27 : Constant  Value=ENUM_PDKEYPTGRAW_OUTZONE
  Constant270 : Constant  Value=ENUM_KEYTYPE_NFC
  Constant273 : Constant  Value=ENUM_KEYMODE_UIDBLE
  Constant275 : Constant  Value=KDKC_DrDoorOpenStaKeep_s
  Constant276 : Constant  Value=ENUM_KEYMODE_DAFAULT
  Constant278 : Constant  Value=ENUM_KEYMODE_NFC
  Constant{28,36,41,43,45,49} (6 alike) : Constant  Value=KDKC_PTGSWCloseTimeout_s
  Constant280 : Constant  Value=ENUM_KEYMODE_DAFAULT
  Constant282 : Constant  Value=ENUM_KEYMODE_DAFAULT
  Constant284 : Constant  Value=ENUM_KEYMODE_UIDUWB
  Constant286 : Constant  Value=ENUM_KEYMODE_INVALID
  Constant287 : Constant  Value=KDKC_DrDoorOpenStaKeep_s
  Constant289 : Constant  Value=KDKC_DKCBTRSSI_dB_ovrdflg
  Constant29 : Constant  Value=ENUM_UIDBUTTON_FRONTHOOD
  Constant290 : Constant  Value=KDKC_DKCBTRSSI_dB_ovrdval
  Constant291 : Constant  Value=ENUM_RSSIAREA_WEAK
  Constant292 : Constant  Value=KDKC_UIDVolBSWtInpSW_ovrdflg
  Constant293 : Constant  Value=3000  OutDataTypeStr=uint16
  Constant294 : Constant  Value=KDKC_UIDRSSIBSWtInpSW_ovrdflg
  Constant295 : Constant  Value=0  OutDataTypeStr=uint16
  Constant296 : Constant  Value=KDKC_JudBTRSSIWeakDeb_cnt
  Constant297 : Constant  Value=KDKC_JudBTRSSIStrongDeb_cnt
  Constant298 : Constant  Value=KDKC_BTRSSISampTime_s
  Constant299 : Constant  Value=TRUE  OutDataTypeStr=uint16
  Constant30 : Constant  Value=ENUM_UIDBUTTON_CHARGECOVER
  Constant300 : Constant  Value=KDKC_JudBTRSSIWeakThres_dB
  Constant301 : Constant  Value=KDKC_JudBTRSSIStrongThres_dB
  Constant302 : Constant  Value=KDKC_StoreUnlockAreaSW_ovrdflg
  Constant303 : Constant  Value=KDKC_StoreUnlockAreaSW_ovrdval
  Constant307 : Constant  Value=KDKC_KeyMissStaSW_ovrdflg
  Constant309 : Constant  Value=KDKC_UnavToUnlReqSW_ovrdflg
  Constant31 : Constant  Value=KDKC_KeyUWBDetArea_enum_ovrdflg
  Constant310 : Constant  Value=KDKC_UnavToUnlReqSW_ovrdval
  Constant311 : Constant  Value=KDKC_KeyMissStaSW_ovrdval  OutDataTypeStr=uint16
  Constant312 : Constant  Value=ENUM_PCMDTOBCM_LOCK
  Constant317 : Constant  Value=ENUM_PCMDTOBCM_LOCK
  Constant32 : Constant  Value=KDKC_KeyUWBDetArea_enum_ovrdval
  Constant320 : Constant  Value=ENUM_PDKEYSPTGRAW_OUTZONE
  Constant321 : Constant  Value=ENUM_PCMD_DEFAULT
  Constant322 : Constant  Value=ENUM_PCMD_RSSIJUDGELOCK
  Constant323 : Constant  Value=ENUM_PCMD_UWBDETEDT
  Constant324 : Constant  Value=ENUM_PCMD_AUTOLOCKJUDGE
  Constant325 : Constant  Value=ENUM_PCMD_PTGJUDGE
  Constant326 : Constant  Value=ENUM_PCMD_NFCDETECT
  Constant327 : Constant  Value=ENUM_PCMD_TRUNKHAND
  Constant328 : Constant  Value=ENUM_PCMD_UIDBUTTON
  Constant329 : Constant  Value=ENUM_UIDBUTTON_RAPSSTARTPRESS
  Constant33 : Constant  Value=KDKC_KeyUWBDetPTGArea_enum_ovrdflg
  Constant330 : Constant  Value=ENUM_PDKEYPTGAREA_UNAVALIABLE
  Constant331 : Constant  Value=ENUM_RSSI_UNAVAILABLE
  Constant332 : Constant  Value=ENUM_PDKEYPTGAREA_PTGZONE
  Constant333 : Constant  Value=ENUM_PDKEYPTGAREA_GRAYSPTGZONE
  Constant334 : Constant  Value=ENUM_PDKEYPTGAREA_SPTGZONE
  Constant336 : Constant  Value=ENUM_RSSI_UNAVAILABLE
  Constant338 : Constant  Value=TRUE
  Constant339 : Constant  Value=TRUE
  Constant34 : Constant  Value=KDKC_KeyUWBDetPTGArea_enum_ovrdval
  Constant340 : Constant  Value=ENUM_RSSI_UNAVAILABLE
  Constant341 : Constant  Value=ENUM_UIDBUTTON_RAPSSTARTRELEASE
  Constant342 : Constant  Value=ENUM_UIDBUTTON_RAPSFORWARDPRESS
  Constant343 : Constant  Value=ENUM_UIDBUTTON_RAPSBACKWARDPRESS
  Constant344 : Constant  Value=ENUM_UIDBUTTON_RAPSFORWARDRELEASE
  Constant345 : Constant  Value=ENUM_UIDBUTTON_RAPSBACKWARRELEASE
  Constant{346,352,364,378} (4 alike) : Constant  Value=ENUM_APSSTASYSTEM_DISABLE
  Constant348 : Constant  Value=ENUM_APSSTASYSTEM_ENABLE
  Constant350 : Constant  Value=KDKC_WaitAPMAPSReqTime_s
  Constant351 : Constant  Value=KDKC_WaitAPMAPSReqTime_s
  Constant354 : Constant  Value=ENUM_PARKINGMODE_DISABLE
  Constant355 : Constant  Value=ENUM_APSSTASYSTEM_REMOTEACTIVE
  Constant356 : Constant  Value=KDKC_WaitAPMJudgUserReqTime_s
  Constant357 : Constant  Value=KDKC_WaitAPMJudgUserReqTime_s
  Constant358 : Constant  Value=ENUM_APSSTASYSTEM_ENABLE
  Constant359 : Constant  Value=ENUM_PARKINGMODE_REMOTEFORWARD
  Constant361 : Constant  Value=ENUM_PARKINGMODE_REMOTEREVERSE
  Constant363 : Constant  Value=ENUM_PARKINGMODE_STANDBY
  Constant365 : Constant  Value=KDKC_DKCStandbyWait60sTime_s
  Constant366 : Constant  Value=KDKC_DKCStandbyWait60sTime_s
  Constant367 : Constant  Value=ENUM_APSSTASYSTEM_ENABLE
  Constant368 : Constant  Value=ENUM_PDKEYRAPSRAW_UNAVALIABLE
  Constant{369,373..376} (5 alike) : Constant  Value=ENUM_PDKEYRAPSRAW_INTOZONE
  Constant37 : Constant  Value=ENUM_PTGINNERSWSTA_PRESS
  Constant370 : Constant  Value=ENUM_PDKEYRAPSRAW_OUTZONE
  Constant371 : Constant  Value=KDKC_KeyUWBDetRAPSArea_enum_ovrdflg
  Constant372 : Constant  Value=KDKC_KeyUWBDetRAPSArea_enum_ovrdval
  Constant377 : Constant  Value=ENUM_PARKINGMODE_STANDBY
  Constant379 : Constant  Value=TRUE
  Constant38 : Constant  Value=ENUM_PTGINNERSWSTA_RELEASE
  Constant387 : Constant  Value=KDKC_APSStaSystem_enum_ovrdflg
  Constant388 : Constant  Value=KDKC_APSStaSystem_enum_ovrdval
  Constant389 : Constant  Value=KDKC_UserReqRAPSLatch_flg_ovrdflg
  Constant39 : Constant  Value=ENUM_PTGINNERSWSTA_PRESS
  Constant390 : Constant  Value=KDKC_UserReqRAPSLatch_flg_ovrdval
  Constant{394..398} (5 alike) : Constant  Value=ENUM_UWBXDISTANCE_ONCANINVALID
  Constant{399,401,403,405,407} (5 alike) : Constant  Value=ENUM_UWBPOWER_BSWINVALID
  Constant{400,402,404,406,408} (5 alike) : Constant  Value=ENUM_UWBPOWER_ONCANINVALID
  Constant409 : Constant  Value=ENUM_UWBPOSX_BSWINVALID
  Constant410 : Constant  Value=ENUM_UWBPOSX_ONCANINVALID
  Constant411 : Constant  Value=ENUM_UWBPOSX_ONCANEXRANGE
  Constant412 : Constant  Value=ENUM_UWBPOSX_ONCANEXRANGE
  Constant413 : Constant  Value=ENUM_UWBPOSY_BSWINVALID
  Constant414 : Constant  Value=ENUM_UWBPOSY_ONCANINVALID
  Constant415 : Constant  Value=ENUM_UWBPOSY_ONCANEXRANGE
  Constant416 : Constant  Value=ENUM_UWBPOSY_ONCANEXRANGE
  Constant42 : Constant  Value=ENUM_PTGINNERSWSTA_RELEASE
  Constant420 : Constant  Value=ENUM_PDKEYRAWLULOCK_OTHERZONE
  Constant421 : Constant  Value=ENUM_PDKEYRAWLULOCK_UNAVALIABLE
  Constant427 : Constant  Commented=on  Value=ENUM_UWBDET_GRAYWELCOMEZONE
  Constant428 : Constant  Commented=on  Value=ENUM_UWBDET_GRAYOUTWELCOMEZONE
  Constant429 : Constant  Value=ENUM_PDKEYRAWLULOCK_OTHERZONE
  Constant430 : Constant  Value=ENUM_PDKEYRAWLULOCK_UNAVALIABLE
  Constant5 : Constant  Value=ENUM_ANTITHEFT_DISARM
  Constant85 : Constant  Value=ENUM_UWBDET_RKEZONE
  Constant86 : Constant  Value=ENUM_UWBDET_GRAYOUTWELCOMEZONE
  Constant88 : Constant  Value=ENUM_UWBDET_GRAYWELCOMEZONE
  Constant89 : Constant  Value=ENUM_UWBDET_RKEZONE
  Constant93 : Constant  Value=ENUM_PCMDTOBCM_LOCK
  Constant96 : Constant  Value=ENUM_POWERSTA_OFFA
  Data Type Conversion{1,8..16,18..40,42,44,46..48,50..52,54..55,57..61,63..72,78..83,85,88..89,97..98,101,121,123,128,136,142..146,148..149} (81 alike) : DataTypeConversion  OutDataTypeStr=uint8
  Data Type Conversion{2..7,45,73..77,84,86..87,90..96,99..100,102..117,119..120,124..126,129,131..132,134..135,147} (51 alike) : DataTypeConversion  OutDataTypeStr=boolean
  Data Type Conversion118 : DataTypeConversion  OutDataTypeStr=uint16
  Data Type Conversion122 : DataTypeConversion
  Data Type Conversion127 : DataTypeConversion  OutDataTypeStr=uint16
  Data Type Conversion130 : DataTypeConversion  OutDataTypeStr=uint16
  Data Type Conversion133 : DataTypeConversion  Commented=on  OutDataTypeStr=boolean
  Data Type Conversion{137..141} (5 alike) : DataTypeConversion  OutDataTypeStr=int16
  Data Type Conversion{17,41,43,49,53,56} (6 alike) : DataTypeConversion  Commented=on  OutDataTypeStr=uint8
  Data Type Conversion62 : DataTypeConversion  OutDataTypeStr=int8
  Detect Change{1..56} (56 alike) : simulink/Logic and Bit Operations/Detect Change  vinit=0  OutDataTypeStr=boolean
  Detect Decrease{,1..20} (21 alike) : simulink/Logic and Bit Operations/Detect Decrease  vinit=0.0  OutDataTypeStr=boolean
  Detect Increase{,1..20,22} (22 alike) : simulink/Logic and Bit Operations/Detect Increase  vinit=0.0  OutDataTypeStr=boolean
  Equal{1..22,24,26,28..37,39..40,42..46,48..49,51..67,69..73,75..78,81..83,85..89,91..103,105..107,109..112,114..129,131,137..138,141..147,149,151..152,156,158,164..165,167,169,171..195,198..199,201..203,205..214,216..217,220..221} (176 alike) : RelationalOperator  Operator===  OutDataTypeStr=boolean  RndMeth=Simplest
  Equal{23,25,27,38,47,79,84,90,104,108,130,132..136,139,148,150,153..155,157,159..163,166,168,170,196..197,200,204,215} (36 alike) : RelationalOperator  Operator=~=  OutDataTypeStr=boolean  RndMeth=Simplest
  Equal{41,50,68,74,80,113,218..219} (8 alike) : RelationalOperator  Commented=on  Operator===  OutDataTypeStr=boolean  RndMeth=Simplest
  Extract Bits : simulink/Logic and Bit Operations/Extract Bits  bitsToExtract=Range of bits  numBits=0  bitIdxRange=[0 0]  outScalingMode=Treat bit field as an integer
  Extract Bits1 : simulink/Logic and Bit Operations/Extract Bits  bitsToExtract=Range of bits  numBits=0  bitIdxRange=[1 1]  outScalingMode=Treat bit field as an integer
  Extract Bits10 : simulink/Logic and Bit Operations/Extract Bits  bitsToExtract=Range of bits  numBits=0  bitIdxRange=[4 4]  outScalingMode=Treat bit field as an integer
  Extract Bits11 : simulink/Logic and Bit Operations/Extract Bits  bitsToExtract=Range of bits  numBits=0  bitIdxRange=[11 11]  outScalingMode=Treat bit field as an integer
  Extract Bits12 : simulink/Logic and Bit Operations/Extract Bits  bitsToExtract=Range of bits  numBits=0  bitIdxRange=[11 11]  outScalingMode=Treat bit field as an integer
  Extract Bits13 : simulink/Logic and Bit Operations/Extract Bits  bitsToExtract=Range of bits  numBits=0  bitIdxRange=[3 3]  outScalingMode=Treat bit field as an integer
  Extract Bits14 : simulink/Logic and Bit Operations/Extract Bits  bitsToExtract=Range of bits  numBits=0  bitIdxRange=[11 11]  outScalingMode=Treat bit field as an integer
  Extract Bits15 : simulink/Logic and Bit Operations/Extract Bits  bitsToExtract=Range of bits  numBits=0  bitIdxRange=[4 4]  outScalingMode=Treat bit field as an integer
  Extract Bits16 : simulink/Logic and Bit Operations/Extract Bits  bitsToExtract=Range of bits  numBits=0  bitIdxRange=[3 3]  outScalingMode=Treat bit field as an integer
  Extract Bits17 : simulink/Logic and Bit Operations/Extract Bits  bitsToExtract=Range of bits  numBits=0  bitIdxRange=[4 4]  outScalingMode=Treat bit field as an integer
  Extract Bits18 : simulink/Logic and Bit Operations/Extract Bits  bitsToExtract=Range of bits  numBits=0  bitIdxRange=[1 1]  outScalingMode=Treat bit field as an integer
  Extract Bits19 : simulink/Logic and Bit Operations/Extract Bits  Commented=on  bitsToExtract=Range of bits  numBits=0  bitIdxRange=[2 2]  outScalingMode=Treat bit field as an integer
  Extract Bits2 : simulink/Logic and Bit Operations/Extract Bits  bitsToExtract=Range of bits  numBits=0  bitIdxRange=[2 2]  outScalingMode=Treat bit field as an integer
  Extract Bits20 : simulink/Logic and Bit Operations/Extract Bits  bitsToExtract=Range of bits  numBits=0  bitIdxRange=[0 0]  outScalingMode=Treat bit field as an integer
  Extract Bits3 : simulink/Logic and Bit Operations/Extract Bits  bitsToExtract=Range of bits  numBits=0  bitIdxRange=[5 5]  outScalingMode=Treat bit field as an integer
  Extract Bits4 : simulink/Logic and Bit Operations/Extract Bits  bitsToExtract=Range of bits  numBits=0  bitIdxRange=[6 6]  outScalingMode=Treat bit field as an integer
  Extract Bits5 : simulink/Logic and Bit Operations/Extract Bits  bitsToExtract=Range of bits  numBits=0  bitIdxRange=[3 3]  outScalingMode=Treat bit field as an integer
  Extract Bits6 : simulink/Logic and Bit Operations/Extract Bits  bitsToExtract=Range of bits  numBits=0  bitIdxRange=[7 7]  outScalingMode=Treat bit field as an integer
  Extract Bits7 : simulink/Logic and Bit Operations/Extract Bits  bitsToExtract=Range of bits  numBits=0  bitIdxRange=[8 8]  outScalingMode=Treat bit field as an integer
  Extract Bits8 : simulink/Logic and Bit Operations/Extract Bits  bitsToExtract=Range of bits  numBits=0  bitIdxRange=[9 9]  outScalingMode=Treat bit field as an integer
  Extract Bits9 : simulink/Logic and Bit Operations/Extract Bits  bitsToExtract=Range of bits  numBits=0  bitIdxRange=[10 10]  outScalingMode=Treat bit field as an integer
  From : From  Commented=on  GotoTag=VINP_BPPTGExistSta_flg
  From{73,83,101,153,185} (5 alike) : From  Commented=on  GotoTag=VDKC_UWBDetPCmdHandSta_enum
  From14 : From  Commented=on  GotoTag=VINP_BPPTGExistSta_flg
  From371 : From  Commented=on  GotoTag=VDKC_UIDButtonUnlock_flg
  From415 : From  Commented=on  GotoTag=VINP_KeyFobAreaU16_enum
  From428 : From  Commented=on  GotoTag=VINP_BPPTGExistSta_flg
  From454 : From  Commented=on  GotoTag=VDKC_KeyUWBDetArea_enum
  From455 : From  Commented=on  GotoTag=VDKC_KeyUWBDetArea_enum
  Goto71 : Goto  Commented=on  GotoTag=VINP_BPPTGExistSta_flg
  Logical Operator{1,38,73,127} (4 alike) : Logic  Inputs=4  AllPortsSameDT=off  OutDataTypeStr=boolean
  Logical Operator{2,5,10,53,55,59,67,74,94..95,97..99,109,114..115,121,138..139,146,150..151,163,165,184,188,206,220..221,223..224} (31 alike) : Logic  Operator=OR  AllPortsSameDT=off  OutDataTypeStr=boolean
  Logical Operator{11..14,16,18,20..21,23,26..27,29..30,32,36,42,44..46,49,51..52,54,56,58,60,63..65,68..71,75,78..80,82..84,86..87,89..90,92..93,100,102..104,106,108,110..111,113,116..117,122..123,132,134,136,140..141,143..145,147..149,153,155..157,159..160,166..173,183,186..187,190..192,199,201,210,212,214,222,225..226} (98 alike) : Logic  AllPortsSameDT=off  OutDataTypeStr=boolean
  Logical Operator{28,31,88,101,105,203} (6 alike) : Logic  Inputs=5  AllPortsSameDT=off  OutDataTypeStr=boolean
  Logical Operator{9,76,96,107,129,137,142} (7 alike) : Logic  Operator=OR  Inputs=4  AllPortsSameDT=off  OutDataTypeStr=boolean
  Logical Operator{37,81,85,112,126,128,131,197} (8 alike) : Logic  Operator=OR  Inputs=3  AllPortsSameDT=off  OutDataTypeStr=boolean
  Logical Operator{3..4,6..7,22,35,39..40,43,47,57,61..62,66,72,118..119,125,133,152,154,158,175..181,185,189,195..196,198,200,204..205,207..209,211,213,216..219,227} (47 alike) : Logic  Operator=NOT  AllPortsSameDT=off  OutDataTypeStr=boolean
  Logical Operator{15,24..25,50,120,135,161..162,164} (9 alike) : Logic  Inputs=3  AllPortsSameDT=off  OutDataTypeStr=boolean
  Logical Operator{17,19,33..34,41,48,77,124,215} (9 alike) : Logic  Operator=OR  Inputs=6  AllPortsSameDT=off  OutDataTypeStr=boolean
  Logical Operator130 : Logic  Operator=OR  Inputs=5  AllPortsSameDT=off  OutDataTypeStr=boolean
  Logical Operator174 : Logic  Inputs=9  AllPortsSameDT=off  OutDataTypeStr=boolean
  Logical Operator182 : Logic  Operator=OR  Inputs=10  AllPortsSameDT=off  OutDataTypeStr=boolean
  Logical Operator193 : Logic  Operator=OR  Inputs=10  AllPortsSameDT=off  OutDataTypeStr=boolean
  Logical Operator194 : Logic  Operator=OR  Inputs=10  AllPortsSameDT=off  OutDataTypeStr=boolean
  Logical Operator202 : Logic  Operator=OR  Inputs=5  AllPortsSameDT=off  OutDataTypeStr=boolean
  Logical Operator8 : Logic  Operator=OR  Inputs=5  AllPortsSameDT=off  OutDataTypeStr=boolean
  Logical Operator91 : Logic  Inputs=6  AllPortsSameDT=off  OutDataTypeStr=boolean
  NFC_PCMD_Chart : Stateflow chart  TreatAsAtomicUnit=on
  PDkeyJudgeBatLowVolt_Chart : Stateflow chart  TreatAsAtomicUnit=on
  PTG_PCMD_Chart : Stateflow chart  TreatAsAtomicUnit=on
  Relational Operator{1..13} (13 alike) : RelationalOperator  OutDataTypeStr=boolean  RndMeth=Simplest
  SR_Latch1 : Subsystem  mask(SR_Latch){}
      mask help: SR latch function.
  SR_Latch10 : Subsystem  mask(SR_Latch){}
      mask help: SR latch function.
  SR_Latch11 : Subsystem  mask(SR_Latch){}
      mask help: SR latch function.
  SR_Latch12 : Subsystem  mask(SR_Latch){}
      mask help: SR latch function.
  SR_Latch13 : Subsystem  mask(SR_Latch){}
      mask help: SR latch function.
  SR_Latch14 : Subsystem  mask(SR_Latch){}
      mask help: SR latch function.
  SR_Latch15 : Subsystem  mask(SR_Latch){}
      mask help: SR latch function.
  SR_Latch16 : Subsystem  mask(SR_Latch){}
      mask help: SR latch function.
  SR_Latch17 : Subsystem  mask(SR_Latch){}
      mask help: SR latch function.
  SR_Latch18 : Subsystem  mask(SR_Latch){}
      mask help: SR latch function.
  SR_Latch19 : Subsystem  mask(SR_Latch){}
      mask help: SR latch function.
  SR_Latch2 : Subsystem  mask(SR_Latch){}
      mask help: SR latch function.
  SR_Latch20 : Subsystem  mask(SR_Latch){}
      mask help: SR latch function.
  SR_Latch21 : Subsystem  mask(SR_Latch){}
      mask help: SR latch function.
  SR_Latch22 : Subsystem  mask(SR_Latch){}
      mask help: SR latch function.
  SR_Latch23 : Subsystem  mask(SR_Latch){}
      mask help: SR latch function.
  SR_Latch24 : Subsystem  mask(SR_Latch){}
      mask help: SR latch function.
  SR_Latch25 : Subsystem  mask(SR_Latch){}
      mask help: SR latch function.
  SR_Latch26 : Subsystem  mask(SR_Latch){}
      mask help: SR latch function.
  SR_Latch3 : hcu_lib/Basic_Blocks/SR_Latch
  SR_Latch4 : Subsystem  mask(SR_Latch){}
      mask help: SR latch function.
  SR_Latch5 : Subsystem  mask(SR_Latch){}
      mask help: SR latch function.
  SR_Latch6 : Subsystem  mask(SR_Latch){}
      mask help: SR latch function.
  SR_Latch7 : hcu_lib/Basic_Blocks/SR_Latch
  SR_Latch8 : Subsystem  mask(SR_Latch){}
      mask help: SR latch function.
  SR_Latch9 : Subsystem  mask(SR_Latch){}
      mask help: SR latch function.
  Switch{,1,10,51,54,63,75..82,99,103,114..115} (18 alike) : Switch  Criteria=u2 > Threshold
  Switch{2..9,11..50,52..53,55..57,60..62,64..74,83..92,94..98,100..102,104..113,132..135} (99 alike) : Switch  Criteria=u2 ~= 0
  Switch{116..120} (5 alike) : Switch  Threshold=2550
  Switch{121..126,129} (7 alike) : Switch  Criteria=u2 ~= 0  Threshold=127
  Switch127 : Switch  Criteria=u2 > Threshold  Threshold=2550
  Switch128 : Switch  Threshold=-2550
  Switch130 : Switch  Criteria=u2 > Threshold  Threshold=2550
  Switch131 : Switch  Threshold=-2550
  Switch93 : Switch  Threshold=-100
  Terminator{,1..5} (6 alike) : Terminator
  Timer1 : Subsystem  mask(Timer){}
      mask help: Timer funcion.
  Timer10 : Subsystem  mask(Timer){}
      mask help: Timer funcion.
  Timer11 : Subsystem  mask(Timer){}
      mask help: Timer funcion.
  Timer12 : Subsystem  mask(Timer){}
      mask help: Timer funcion.
  Timer13 : Subsystem  mask(Timer){}
      mask help: Timer funcion.
  Timer2 : Subsystem  mask(Timer){}
      mask help: Timer funcion.
  Timer3 : hcu_lib/Basic_Blocks/Timer
  Timer4 : hcu_lib/Basic_Blocks/Timer
  Timer5 : Subsystem  mask(Timer){}
      mask help: Timer funcion.
  Timer6 : Subsystem  mask(Timer){}
      mask help: Timer funcion.
  Timer7 : Subsystem  mask(Timer){}
      mask help: Timer funcion.
  Timer8 : Subsystem  mask(Timer){}
      mask help: Timer funcion.
  Timer9 : Subsystem  mask(Timer){}
      mask help: Timer funcion.
  TrunkHanSW_PCMD_Chart : Stateflow chart  TreatAsAtomicUnit=on
  UIDButton_PCMD_Chart : Stateflow chart  TreatAsAtomicUnit=on
  UWB_PCMD_Chart : Stateflow chart  TreatAsAtomicUnit=on
  Unit Delay{,1..17,19..46,49..63,67} (62 alike) : UnitDelay  SampleTime=-1  HasFrameUpgradeWarning=on
  Unit Delay18 : UnitDelay  Commented=on  SampleTime=-1  HasFrameUpgradeWarning=on
  VDKC_FDCPCommandToBCM_enum : Outport
  VDKC_FDCKeyAreaLockUnlock_enum : Outport  Port=2
  VDKC_FDCKeyAreaPS_enum : Outport  Port=3
  VDKC_FDCKeyAreaPTG_enum : Outport  Port=4
  VDKC_FDCKeyAreaSPTG_enum : Outport  Port=5
  VDKC_FDCKeyWelcomeSta_enum : Outport  Port=6
  VDKC_FDCKeyAllowSleep_flg : Outport  Port=7
  VDKC_KeyMissSta_flg : Outport  Port=8
  VDKC_UIDLowPowerSta_flg : Outport  Port=9
  VDKC_KeyModeSta_enum : Outport  Port=10
  VDKC_KeyTypeSta_enum : Outport  Port=11
  VDKC_DkeyShowIVISta_enum : Outport  Port=12
  VDKC_JudgeKeepUnlockZone_flg : Outport  Port=13
  VDKC_OutputPCMDModule_enum : Outport  Port=14
  VDKC_UWBDetArea_enum : Outport  Port=15
  VDKC_BLERSSI_enum : Outport  Port=16
  VDKC_UWBDetPTGArea_enum : Outport  Port=17
  VDKC_UIDBatVolt_enum : Outport  Port=18
  VDKC_DkeyAreaRAPSSta_enum : Outport  Port=19
  VDKC_ParkingModeCmd_enum : Outport  Port=20
  VDKC_UWB1Distance_enum : Outport  Port=21
  VDKC_UWB2Distance_enum : Outport  Port=22
  VDKC_UWB3Distance_enum : Outport  Port=23
  VDKC_UWB4Distance_enum : Outport  Port=24
  VDKC_UWB0Distance_enum : Outport  Port=25
  VDKC_UWB1FPP_enum : Outport  Port=26
  VDKC_UWB2FPP_enum : Outport  Port=27
  VDKC_UWB3FPP_enum : Outport  Port=28
  VDKC_UWB4FPP_enum : Outport  Port=29
  VDKC_UWB0FPP_enum : Outport  Port=30
  VDKC_CoordinateX_enum : Outport  Port=31
  VDKC_CoordinateY_enum : Outport  Port=32
  VDKC_UWB1Invalid_flg : Outport  Port=33
  VDKC_UWB2Invalid_flg : Outport  Port=34
  VDKC_UWB3Invalid_flg : Outport  Port=35
  VDKC_UWB4Invalid_flg : Outport  Port=36
  VDKC_UWB0Invalid_flg : Outport  Port=37
  VDKC_UWBOnOff_flg : Outport  Port=38
  wires:
  Unit Delay46/1 -> UIDButton_PCMD_Chart/5(VDKC_UserReqRAPSLatch_flg)
  [VDKC_UserReqRAPSLatch_flg] -> Unit Delay46/1
  Switch57/1 -> UWB_PCMD_Chart/7(VDKC_UWBDetKeepUnltoOther_flg)
  [VDKC_UWBDetKeepUnltoOther_flg] -> Switch57/1
  [VDKC_UserReqRAPSLatch_flg] -> Logical Operator227/1
  Logical Operator227/1 -> Switch57/2
  Constant231/1 -> Switch57/3
  Logical Operator225/1 -> [VDKC_UWBDetKeepUnltoOther_flg]  "VDKC_UWBDetKeepUnltoOther_flg"
  Equal221/1 -> Logical Operator225/1
  Data Type Conversion149/1 -> Equal221/1
  Unit Delay63/1 -> Data Type Conversion149/1
  Constant423/1 -> Equal221/2
  Logical Operator226/1 -> Logical Operator225/2
  Equal220/1 -> Logical Operator226/2
  Detect Change56/1 -> Logical Operator226/1
  Constant429/1 -> Equal220/2
  [VDKC_UWBDetUnlockKeepSta_enum] -> Unit Delay63/1, Detect Change56/1, Equal220/1
  Equal217/1 -> Logical Operator224/2
  Equal212/1 -> Logical Operator224/1
  Logical Operator224/1 -> Switch132/2
  Constant428/1 -> Equal219/2
  From455/1 -> Equal219/1
  From454/1 -> Equal218/1
  Constant427/1 -> Equal218/2
  Constant426/1 -> Equal217/2
  [VDKC_KeyUWBDetArea_enum] -> Equal217/1
  [VDKC_UWBDetUnLockSta_enum] -> Switch134/1
  Data Type Conversion148/1 -> Switch135/1
  Unit Delay62/1 -> Data Type Conversion148/1
  Constant430/1 -> Switch135/3
  Equal216/1 -> Switch135/2
  Constant425/1 -> Equal216/2
  [VDKC_BTConnectSta_enum] -> Equal216/1
  Switch135/1 -> Switch134/3
  Equal215/1 -> Switch134/2
  [VDKC_KeyUWBDetArea_enum] -> Equal215/1
  Constant424/1 -> Equal215/2
  Switch134/1 -> [VDKC_UWBDetUnlockKeepSta_enum], Unit Delay62/1  "VDKC_UWBDetUnlockKeepSta_enum"
  Constant420/1 -> Switch132/3
  Constant421/1 -> Switch132/1
  [VDKC_KeyUWBDetArea_enum] -> Equal212/1
  Switch132/1 -> Switch133/3
  Switch133/1 -> [VDKC_UWBDetUnLockSta_enum]  "VDKC_UWBDetUnLockSta_enum"
  Constant422/1 -> Equal213/2
  [VDKC_KeyUWBDetArea_enum] -> Equal213/1
  Constant419/1 -> Switch133/1
  Logical Operator223/1 -> Switch133/2
  Equal213/1 -> Logical Operator223/1
  [VDKC_KeyUWBDetArea_enum] -> Equal214/1
  Constant417/1 -> Equal214/2
  Equal214/1 -> Logical Operator223/2
  Constant418/1 -> Equal212/2
  Data Type Conversion147/1 -> VDKC_UWBOnOff_flg/1  "VDKC_UWBOnOff_flg"
  VINP_UWBRangingON_flg/1 -> Data Type Conversion147/1
  Data Type Conversion146/1 -> VDKC_UWB0Invalid_flg/1  "VDKC_UWB0Invalid_flg"
  VINP_UWB5RangingSta_enum/1 -> Data Type Conversion146/1
  Data Type Conversion145/1 -> VDKC_UWB4Invalid_flg/1  "VDKC_UWB4Invalid_flg"
  VINP_UWB4RangingSta_enum/1 -> Data Type Conversion145/1
  Data Type Conversion144/1 -> VDKC_UWB3Invalid_flg/1  "VDKC_UWB3Invalid_flg"
  VINP_UWB3RangingSta_enum/1 -> Data Type Conversion144/1
  Data Type Conversion143/1 -> VDKC_UWB2Invalid_flg/1  "VDKC_UWB2Invalid_flg"
  VINP_UWB2RangingSta_enum/1 -> Data Type Conversion143/1
  Data Type Conversion142/1 -> VDKC_UWB1Invalid_flg/1  "VDKC_UWB1Invalid_flg"
  VINP_UWB1RangingSta_enum/1 -> Data Type Conversion142/1
  Data Type Conversion141/1 -> Equal209/2, Switch125/3
  Data Type Conversion140/1 -> Switch124/3, Equal208/2
  Data Type Conversion139/1 -> Equal207/2, Switch123/3
  Data Type Conversion138/1 -> Switch122/3, Equal206/2
  VINP_UWB1Power_dB/1 -> Data Type Conversion137/1
  Data Type Conversion137/1 -> Equal205/2, Switch121/3
  VINP_UWBpositionY_cm/1 -> Switch129/3, Equal211/2
  Equal211/1 -> Switch129/2
  Constant413/1 -> Equal211/1
  Constant414/1 -> Switch129/1
  Switch129/1 -> Switch130/3, Switch130/2
  Constant415/1 -> Switch130/1
  Switch130/1 -> Switch131/1, Switch131/2
  Constant416/1 -> Switch131/3
  Switch131/1 -> VDKC_CoordinateY_enum/1  "VDKC_CoordinateY_enum"
  Switch128/1 -> VDKC_CoordinateX_enum/1  "VDKC_CoordinateX_enum"
  Constant412/1 -> Switch128/3
  Switch127/1 -> Switch128/2, Switch128/1
  Constant411/1 -> Switch127/1
  Switch126/1 -> Switch127/2, Switch127/3
  Constant410/1 -> Switch126/1
  Constant409/1 -> Equal210/1
  Equal210/1 -> Switch126/2
  VINP_UWBpositionX_cm/1 -> Equal210/2, Switch126/3
  Switch125/1 -> VDKC_UWB0FPP_enum/1  "VDKC_UWB0FPP_enum"
  Switch124/1 -> VDKC_UWB4FPP_enum/1  "VDKC_UWB4FPP_enum"
  Switch123/1 -> VDKC_UWB3FPP_enum/1  "VDKC_UWB3FPP_enum"
  Switch122/1 -> VDKC_UWB2FPP_enum/1  "VDKC_UWB2FPP_enum"
  VINP_UWB5Power_dB/1 -> Data Type Conversion141/1
  Constant408/1 -> Switch125/1
  Equal209/1 -> Switch125/2
  Constant407/1 -> Equal209/1
  Constant405/1 -> Equal208/1
  VINP_UWB4Power_dB/1 -> Data Type Conversion140/1
  Equal208/1 -> Switch124/2
  Constant406/1 -> Switch124/1
  Constant404/1 -> Switch123/1
  Equal207/1 -> Switch123/2
  VINP_UWB3Power_dB/1 -> Data Type Conversion139/1
  Constant403/1 -> Equal207/1
  Constant401/1 -> Equal206/1
  VINP_UWB2Power_dB/1 -> Data Type Conversion138/1
  Equal206/1 -> Switch122/2
  Constant402/1 -> Switch122/1
  Switch121/1 -> VDKC_UWB1FPP_enum/1  "VDKC_UWB1FPP_enum"
  Constant400/1 -> Switch121/1
  Equal205/1 -> Switch121/2
  Constant399/1 -> Equal205/1
  Switch120/1 -> VDKC_UWB0Distance_enum/1  "VDKC_UWB0Distance_enum"
  Switch119/1 -> VDKC_UWB4Distance_enum/1  "VDKC_UWB4Distance_enum"
  Switch118/1 -> VDKC_UWB3Distance_enum/1  "VDKC_UWB3Distance_enum"
  Switch117/1 -> VDKC_UWB2Distance_enum/1  "VDKC_UWB2Distance_enum"
  Constant398/1 -> Switch120/1
  VINP_UWB5Distance_cm/1 -> Switch120/2, Switch120/3
  VINP_UWB4Distance_cm/1 -> Switch119/2, Switch119/3
  Constant397/1 -> Switch119/1
  Constant396/1 -> Switch118/1
  VINP_UWB3Distance_cm/1 -> Switch118/2, Switch118/3
  VINP_UWB2Distance_cm/1 -> Switch117/2, Switch117/3
  Constant395/1 -> Switch117/1
  Switch116/1 -> VDKC_UWB1Distance_enum/1  "VDKC_UWB1Distance_enum"
  Constant394/1 -> Switch116/1
  VINP_UWB1Distance_cm/1 -> Switch116/2, Switch116/3
  Constant393/1 -> Equal204/2
  [VDKC_UWBDetPSZoneKeepSta_enum] -> Equal204/1
  Equal204/1 -> Logical Operator222/2
  Equal25/1 -> Logical Operator222/1
  Logical Operator222/1 -> Logical Operator25/3
  Equal24/1 -> Logical Operator221/2
  Constant392/1 -> Equal203/2
  [VDKC_UWBDetPSZoneKeepSta_enum] -> Equal203/1
  [VDKC_UWBDetPSZoneKeepSta_enum] -> Equal24/1
  Logical Operator221/1 -> Logical Operator24/3
  Constant46/1 -> Equal24/2
  Equal203/1 -> Logical Operator221/1
  Logical Operator220/1 -> Logical Operator45/2
  Equal202/1 -> Logical Operator220/2
  Constant391/1 -> Equal202/2
  [VDKC_UWBDetPSZoneKeepSta_enum] -> Equal202/1
  SR_Latch21/1(latched) -> Switch115/3
  Switch115/1 -> [VDKC_UserReqRAPSLatch_flg]
  Constant389/1 -> Switch115/2
  Constant390/1 -> Switch115/1
  Constant388/1 -> Switch114/1
  VINP_APSStaSystem_enum/1 -> Switch114/3
  Constant387/1 -> Switch114/2
  Switch114/1 -> [VDKC_APSStaSystem_enum]  "VDKC_APSStaSystem_enum"
  Unit Delay59/1 -> Logical Operator182/10
  Unit Delay57/1 -> Logical Operator182/9
  Unit Delay55/1 -> Logical Operator182/8
  Equal185/1 -> Logical Operator182/7
  Logical Operator183/1 -> Logical Operator182/6
  Switch113/1 -> UWB_PCMD_Chart/8(VDKC_UnavToUnlReqUnlock_flg)
  Constant386/1 -> Switch113/3
  Logical Operator219/1 -> Switch113/2
  [VDKC_UserReqRAPSLatch_flg] -> Logical Operator219/1
  [VDKC_UnavToUnlReqUnlock_flg] -> Switch113/1
  Switch112/1 -> UWB_PCMD_Chart/6(VDKC_UIDDetRSSIChgToLock_flg)
  [VDKC_UIDDetRSSIChgToLock_flg] -> Switch112/1
  [VDKC_UserReqRAPSLatch_flg] -> Logical Operator218/1
  Logical Operator218/1 -> Switch112/2
  Constant385/1 -> Switch112/3
  Switch111/1 -> UWB_PCMD_Chart/5(VDKC_UWBDetReqtoUnlock_flg)
  Constant384/1 -> Switch111/3
  Logical Operator217/1 -> Switch111/2
  [VDKC_UserReqRAPSLatch_flg] -> Logical Operator217/1
  [VDKC_UWBDetAreaChaToUnlock_flg] -> Switch111/1
  Switch110/1 -> UWB_PCMD_Chart/4(VDKC_UWBDetReqtoLock_flg)
  [VDKC_UWBDetAreaChangeToLock_flg] -> Switch110/1
  [VDKC_UserReqRAPSLatch_flg] -> Logical Operator216/1
  Logical Operator216/1 -> Switch110/2
  Constant383/1 -> Switch110/3
  [VDKC_RPAStandbyTcTrig_flg] -> Logical Operator215/6
  [VDKC_WaitUserReqTrgT_flg] -> Logical Operator215/5
  [VDKC_WaitAPMReqEnTrgT_flg] -> Logical Operator215/4
  [VDKC_UIDForWPressLacth_flg] -> Logical Operator215/3
  [VDKC_UIDBackWPressLacth_flg] -> Logical Operator215/2
  [VDKC_UserReqRAPSLatch_flg] -> Logical Operator215/1
  Switch102/1 -> Switch101/3
  Logical Operator215/1 -> Logical Operator130/5  "VDKC_DKCRAPSTimerActive_flg"
  [VDKC_UserReqRAPSLatch_flg] -> Unit Delay61/1
  Unit Delay61/1 -> Logical Operator214/2
  Logical Operator214/1 -> Switch109/2
  Equal201/1 -> Logical Operator214/1
  [VDKC_DkeyRAPSAreaRaw_enum] -> Switch108/1
  Switch104/1 -> [VDKC_DkeyRAPSAreaRaw_enum]  "VDKC_DkeyRAPSAreaRaw_enum"
  Data Type Conversion136/1 -> Switch109/1
  Unit Delay60/1 -> Data Type Conversion136/1
  Constant380/1 -> Switch109/3
  Constant382/1 -> Equal201/2
  [VDKC_BTConnectSta_enum] -> Equal201/1
  Switch109/1 -> Switch108/3
  Equal200/1 -> Switch108/2
  [VDKC_KeyUWBDetArea_enum] -> Equal200/1
  Constant381/1 -> Equal200/2
  Switch108/1 -> Unit Delay60/1, Switch103/3  "VDKC_UWBDetRAPSZoneKeep_enum"
  Constant337/1 -> Switch107/3
  [VDKC_UIDButtonFrontHood_flg] -> Switch107/1
  Logical Operator213/1 -> Switch107/2
  [VDKC_UserReqRAPSLatch_flg] -> Logical Operator213/1
  Switch107/1 -> UIDButton_PCMD_Chart/6(VDKC_UIDButtonFrontHood_flg)
  Logical Operator212/1 -> Switch84/2
  Logical Operator211/1 -> Logical Operator212/2
  Constant379/1 -> Logical Operator212/1
  [VDKC_UserReqRAPSLatch_flg] -> Logical Operator211/1
  Logical Operator209/1 -> Logical Operator210/2
  Logical Operator210/1 -> Switch85/2
  Constant339/1 -> Logical Operator210/1
  [VDKC_UserReqRAPSLatch_flg] -> Logical Operator209/1
  [VDKC_UIDButtonBackWRelease_flg] -> Logical Operator208/1
  [VDKC_UIDButtonForWRelease_flg] -> Logical Operator207/1
  Logical Operator208/1 -> Logical Operator203/5
  Logical Operator207/1 -> Logical Operator203/4
  [VDKC_UIDButtonBackWRelease_flg] -> Logical Operator202/5
  [VDKC_UIDButtonForWRelease_flg] -> Logical Operator202/4
  Logical Operator181/1 -> Logical Operator174/8
  Logical Operator180/1 -> Logical Operator174/7
  Logical Operator179/1 -> Logical Operator174/6
  Logical Operator178/1 -> Logical Operator174/5
  Logical Operator177/1 -> Logical Operator174/4
  Logical Operator176/1 -> Logical Operator174/3
  Equal199/1 -> Logical Operator174/2
  Equal195/1 -> Logical Operator174/9
  [VDKC_APSStaSystem_enum] -> Equal199/1
  Constant378/1 -> Equal199/2
  [VDKC_ParkingModeCmd_enum] -> Terminator5/1
  [VDKC_UIDButtonStartRelease_flg] -> Terminator4/1
  Constant377/1 -> Switch106/3
  Switch101/1 -> Switch106/1
  Equal198/1 -> Switch106/2
  Constant376/1 -> Equal198/2
  [VDKC_DkeyAreaRAPSSta_enum] -> Equal198/1
  Switch106/1 -> Switch94/1
  Constant375/1 -> Equal197/2
  [VDKC_DkeyAreaRAPSSta_enum] -> Equal197/1
  Equal197/1 -> Logical Operator194/10
  Equal196/1 -> Logical Operator193/10
  [VDKC_DkeyAreaRAPSSta_enum] -> Equal196/1
  Constant374/1 -> Equal196/2
  Constant373/1 -> Equal195/2
  [VDKC_DkeyAreaRAPSSta_enum] -> Equal195/1
  Data Type Conversion135/1 -> Logical Operator206/2
  [VINP_KeyFobAreaU16_enum] -> Extract Bits18/1
  Extract Bits18/1 -> Data Type Conversion135/1
  Data Type Conversion134/1 -> Logical Operator206/1
  Logical Operator206/1 -> Switch104/2
  Switch103/1 -> [VDKC_DkeyAreaRAPSSta_enum], VDKC_DkeyAreaRAPSSta_enum/1  "VDKC_DkeyAreaRAPSSta_enum"
  Constant370/1 -> Switch105/1
  Constant368/1 -> Switch105/3
  [VINP_KeyFobAreaU16_enum] -> Switch105/2
  Switch105/1 -> Switch104/3
  Constant369/1 -> Switch104/1
  Extract Bits20/1 -> Data Type Conversion134/1
  [VINP_KeyFobAreaU16_enum] -> Extract Bits20/1
  Constant372/1 -> Switch103/1
  Constant371/1 -> Switch103/2
  Extract Bits19/1 -> Data Type Conversion133/1
  From415/1 -> Extract Bits19/1
  [VDKC_UIDButtonBackWPress_flg] -> Logical Operator205/1
  Logical Operator205/1 -> Logical Operator203/2
  Logical Operator204/1 -> Logical Operator203/1
  [VDKC_UIDButtonForWPress_flg] -> Logical Operator204/1
  Logical Operator203/1 -> Timer13/1(trigger), [VDKC_RPAStandbyTcTrig_flg]  "VDKC_RPAStandbyTcTrig_flg"
  Logical Operator202/1 -> Timer13/2(reset)
  [VDKC_UIDButtonForWPress_flg] -> Logical Operator202/2
  [VDKC_UIDButtonBackWPress_flg] -> Logical Operator202/3
  Logical Operator198/1 -> Logical Operator202/1
  [VDKC_RPAWait60sReqTout_flg] -> Unit Delay59/1
  Equal194/1 -> Logical Operator197/3
  [VDKC_APSStaSystem_enum] -> Equal194/1
  Constant364/1 -> Equal194/2
  [VDKC_UserReqRAPSLatch_flg] -> Logical Operator200/1
  Logical Operator200/1 -> Logical Operator197/2
  Data Type Conversion132/1 -> Logical Operator197/1
  Logical Operator197/1 -> SR_Latch26/2(reset)
  [task_time_s] -> Timer13/3(Ts)
  Constant365/1 -> Timer13/4(max_time)
  SR_Latch26/1(latched) -> Logical Operator198/1, Logical Operator203/3
  Constant366/1 -> Relational Operator13/2
  Timer13/1(time) -> Relational Operator13/1
  Unit Delay58/1 -> Data Type Conversion132/1
  Relational Operator13/1 -> [VDKC_RPAWait60sReqTout_flg], Unit Delay58/1  "VDKC_RPAWait60sReqTout_flg"
  Logical Operator199/1 -> SR_Latch26/1(set)
  [VDKC_UserReqRAPSLatch_flg] -> Logical Operator199/1
  Equal193/1 -> Logical Operator201/2
  Detect Increase22/1 -> Logical Operator201/1
  Constant367/1 -> Equal193/2
  [VDKC_APSStaSystem_enum] -> Equal193/1, Detect Increase22/1
  Logical Operator201/1 -> Logical Operator199/2
  Constant363/1 -> Switch102/3
  Logical Operator196/1 -> Logical Operator194/9
  [VDKC_UserReqRAPSLatch_flg] -> Logical Operator196/1
  [VDKC_AnyDoorSta_flg] -> Logical Operator194/8
  [VDKC_AnyDoorSta_flg] -> Logical Operator193/8
  [VDKC_UserReqRAPSLatch_flg] -> Logical Operator195/1
  Logical Operator195/1 -> Logical Operator193/9
  Logical Operator194/1 -> SR_Latch25/2(reset)  "VDKC_UIDBackWReset_flg"
  [VDKC_UIDButtonBackWRelease_flg] -> Logical Operator194/1
  [VDKC_UIDButtonUnlock_flg] -> Logical Operator194/2
  [VDKC_UIDButtonLock_flg] -> Logical Operator194/3
  [VDKC_UIDButtonForWPress_flg] -> Logical Operator194/4
  [VDKC_UIDButtonStartPress_flg] -> Logical Operator194/5
  [VDKC_BTConnectSta_enum] -> Equal192/1
  Constant362/1 -> Equal192/2
  Equal192/1 -> Logical Operator194/7
  [VDKC_UIDButtonCarSearch_flg] -> Logical Operator194/6
  [VDKC_UIDButtonBackWPress_flg] -> SR_Latch25/1(set)
  Constant361/1 -> Switch102/1
  SR_Latch25/1(latched) -> Switch102/2, [VDKC_UIDBackWPressLacth_flg]  "VDKC_UIDBackWPressLacth_flg"
  [VDKC_UIDButtonCarSearch_flg] -> Logical Operator193/6
  Equal191/1 -> Logical Operator193/7
  Constant360/1 -> Equal191/2
  [VDKC_BTConnectSta_enum] -> Equal191/1
  [VDKC_UIDButtonStartPress_flg] -> Logical Operator193/5
  [VDKC_UIDButtonBackWPress_flg] -> Logical Operator193/4
  [VDKC_UIDButtonLock_flg] -> Logical Operator193/3
  [VDKC_UIDButtonUnlock_flg] -> Logical Operator193/2
  [VDKC_UIDButtonForWRelease_flg] -> Logical Operator193/1
  Logical Operator193/1 -> SR_Latch24/2(reset)  "VDKC_UIDForWReset_flg"
  SR_Latch24/1(latched) -> [VDKC_UIDForWPressLacth_flg], Switch101/2  "VDKC_UIDForWPressLacth_flg"
  [VDKC_UIDButtonForWPress_flg] -> SR_Latch24/1(set)
  Constant359/1 -> Switch101/1
  [VDKC_WaitAPMJuUserReqTout_flg] -> Unit Delay57/1
  Logical Operator192/1 -> Logical Operator190/2
  [VDKC_APSStaSystem_enum] -> Detect Increase20/1, Equal189/1
  Constant358/1 -> Equal189/2
  Detect Increase20/1 -> Logical Operator192/1
  Equal189/1 -> Logical Operator192/2
  [VDKC_UserReqRAPSLatch_flg] -> Logical Operator190/1
  Logical Operator190/1 -> SR_Latch22/1(set)
  Relational Operator11/1 -> [VDKC_WaitAPMJuUserReqTout_flg], Unit Delay56/1  "VDKC_WaitAPMJuUserReqTout_flg"
  Unit Delay56/1 -> Data Type Conversion131/1
  Timer11/1(time) -> Relational Operator11/1
  Constant357/1 -> Relational Operator11/2
  Logical Operator189/1 -> Timer11/2(reset)
  SR_Latch22/1(latched) -> Logical Operator189/1, Timer11/1(trigger), [VDKC_WaitUserReqTrgT_flg]  "VDKC_WaitUserReqTrgT_flg"
  Constant356/1 -> Timer11/4(max_time)
  [task_time_s] -> Timer11/3(Ts)
  Logical Operator188/1 -> SR_Latch22/2(reset)
  Data Type Conversion131/1 -> Logical Operator188/1
  [VDKC_APSStaSystem_enum] -> Detect Increase19/1, Equal190/1
  Constant355/1 -> Equal190/2
  Detect Increase19/1 -> Logical Operator191/1
  Equal190/1 -> Logical Operator191/2
  Logical Operator191/1 -> Logical Operator188/2
  Constant354/1 -> Switch94/3
  Switch94/1 -> VDKC_ParkingModeCmd_enum/1, [VDKC_ParkingModeCmd_enum]  "VDKC_ParkingModeCmd_enum"
  Constant353/1 -> Data Type Conversion130/1
  Data Type Conversion130/1 -> Switch100/3
  Data Type Conversion127/1 -> Switch100/1
  Switch100/1 -> VDKC_UIDBatVolt_enum/1  "VDKC_UIDBatVolt_enum"
  Equal188/1 -> Switch100/2
  Constant349/1 -> Equal188/2
  [VDKC_BTConnectSta_enum] -> Equal188/1
  [VDKC_UserReqRAPSLatch_flg] -> Switch94/2
  [VDKC_WaitAPMReqTimeout_flg] -> Unit Delay55/1
  Logical Operator187/1 -> Logical Operator184/2
  Equal187/1 -> Logical Operator187/2
  Detect Increase17/1 -> Logical Operator187/1
  Constant348/1 -> Equal187/2
  [VDKC_APSStaSystem_enum] -> Equal187/1, Detect Increase17/1
  Data Type Conversion129/1 -> Logical Operator184/1
  Logical Operator184/1 -> SR_Latch23/2(reset)
  Equal186/1 -> Logical Operator186/2
  Constant352/1 -> Equal186/2
  [VDKC_APSStaSystem_enum] -> Equal186/1
  [task_time_s] -> Timer12/3(Ts)
  Constant350/1 -> Timer12/4(max_time)
  SR_Latch23/1(latched) -> Timer12/1(trigger), [VDKC_WaitAPMReqEnTrgT_flg], Logical Operator185/1  "VDKC_WaitAPMReqEnTrgT_flg"
  Logical Operator185/1 -> Timer12/2(reset)
  Constant351/1 -> Relational Operator12/2
  Timer12/1(time) -> Relational Operator12/1
  Unit Delay54/1 -> Data Type Conversion129/1
  Relational Operator12/1 -> Unit Delay54/1, [VDKC_WaitAPMReqTimeout_flg]  "VDKC_WaitAPMReqTimeout_flg"
  [VDKC_UserReqRAPSLatch_flg] -> Detect Increase18/1
  Detect Increase18/1 -> Logical Operator186/1
  Logical Operator186/1 -> SR_Latch23/1(set)
  [VDKC_BTConnectSta_enum] -> Equal185/1
  Constant347/1 -> Equal185/2
  Constant346/1 -> Equal183/2
  Equal183/1 -> Logical Operator183/2
  Detect Decrease19/1 -> Logical Operator183/1
  [VDKC_APSStaSystem_enum] -> Detect Decrease19/1, Equal183/1
  [VDKC_UIDButtonLock_flg] -> Logical Operator182/5
  [VINP_HoodSW_flg] -> Logical Operator182/2
  [VINP_TailgateSW_flg] -> Logical Operator182/1
  [VINP_BrakeSWSta_flg] -> Logical Operator182/4
  [VDKC_ACCSWSta_flg] -> Logical Operator182/3
  Logical Operator182/1 -> SR_Latch21/2(reset)  "VDKC_RAPStopTrigger_flg"
  Logical Operator174/1 -> SR_Latch21/1(set)  "VDKC_UserReqRAPTrigger_flg"
  [VDKC_UIDButtonStartPress_flg] -> Logical Operator174/1
  [VINP_SeatSW_flg] -> Logical Operator181/1
  [VDKC_ACCSWSta_flg] -> Logical Operator180/1
  [VINP_BrakeSWSta_flg] -> Logical Operator179/1
  [VINP_HoodSW_flg] -> Logical Operator178/1
  [VINP_TailgateSW_flg] -> Logical Operator177/1
  [VDKC_AnyDoorSta_flg] -> Logical Operator176/1
  Logical Operator175/1 -> [VDKC_ACCSWSta_flg]  "VDKC_ACCSWSta_flg"
  VTQD_LowIdleAccPedal_flg/1 -> Logical Operator175/1
  VINP_HoodSW_flg/1 -> [VINP_HoodSW_flg]
  Logical Operator173/1 -> [VDKC_UIDButtonBackWRelease_flg]  "VDKC_UIDButtonBackWRelease_flg"
  Equal181/1 -> Logical Operator173/2
  Detect Change55/1 -> Logical Operator173/1
  Constant345/1 -> Equal181/2
  [VDKC_UIDBLEBatton_Cmd] -> Detect Change55/1, Equal181/1
  [VDKC_UIDBLEBatton_Cmd] -> Equal180/1, Detect Change54/1
  Constant344/1 -> Equal180/2
  Detect Change54/1 -> Logical Operator172/1
  Equal180/1 -> Logical Operator172/2
  Logical Operator172/1 -> [VDKC_UIDButtonForWRelease_flg]  "VDKC_UIDButtonForWRelease_flg"
  [VDKC_UIDBLEBatton_Cmd] -> Equal179/1, Detect Change53/1
  Constant343/1 -> Equal179/2
  Detect Change53/1 -> Logical Operator171/1
  Equal179/1 -> Logical Operator171/2
  Logical Operator171/1 -> [VDKC_UIDButtonBackWPress_flg]  "VDKC_UIDButtonBackWPress_flg"
  Logical Operator170/1 -> [VDKC_UIDButtonForWPress_flg]  "VDKC_UIDButtonForWPress_flg"
  Equal178/1 -> Logical Operator170/2
  Detect Change52/1 -> Logical Operator170/1
  Constant342/1 -> Equal178/2
  [VDKC_UIDBLEBatton_Cmd] -> Detect Change52/1, Equal178/1
  Logical Operator169/1 -> [VDKC_UIDButtonStartRelease_flg]  "VDKC_UIDButtonStartRelease_flg"
  Equal177/1 -> Logical Operator169/2
  Detect Change51/1 -> Logical Operator169/1
  Constant341/1 -> Equal177/2
  [VDKC_UIDBLEBatton_Cmd] -> Detect Change51/1, Equal177/1
  [VDKC_UIDBLEBatton_Cmd] -> Equal176/1, Detect Change50/1
  Constant329/1 -> Equal176/2
  Detect Change50/1 -> Logical Operator168/1
  Equal176/1 -> Logical Operator168/2
  Logical Operator168/1 -> [VDKC_UIDButtonStartPress_flg]  "VDKC_UIDButtonStartPress_flg"
  Switch93/1 -> Switch99/3
  Constant331/1 -> Switch93/3
  Data Type Conversion123/1 -> Switch93/1
  Abs/1 -> Data Type Conversion123/1
  [VDKC_DKCBTRSSI_dB] -> Abs/1, Switch93/2
  [VDKC_DKCBTRSSI_dB] -> Switch99/2
  Constant340/1 -> Switch99/1
  [VDKC_UIDBatVoltx1000_V] -> Data Type Conversion127/1
  Constant338/1 -> Switch83/2
  Constant336/1 -> Switch95/3
  Switch99/1 -> Switch95/1
  Switch95/1 -> VDKC_BLERSSI_enum/1  "VDKC_BLERSSI_enum"
  Equal175/1 -> Switch95/2
  [VDKC_BTConnectSta_enum] -> Equal175/1
  Constant335/1 -> Equal175/2
  Constant334/1 -> Switch96/1
  Constant332/1 -> Switch97/1
  Constant333/1 -> Switch98/1
  Switch96/1 -> VDKC_UWBDetPTGArea_enum/1  "VDKC_UWBDetPTGArea_enum"
  Switch98/1 -> Switch97/3
  Switch97/1 -> Switch96/3
  [VINP_KeyFobAreaU16_enum] -> Extract Bits16/1
  Extract Bits16/1 -> Data Type Conversion124/1
  Constant330/1 -> Switch98/3
  Data Type Conversion124/1 -> Switch96/2
  [VINP_KeyFobAreaU16_enum] -> Extract Bits17/1
  Extract Bits17/1 -> Data Type Conversion125/1
  Data Type Conversion125/1 -> Switch97/2
  Extract Bits14/1 -> Data Type Conversion126/1
  [VINP_KeyFobAreaU16_enum] -> Extract Bits14/1
  Data Type Conversion126/1 -> Switch98/2
  Data Type Conversion122/1 -> VDKC_UWBDetArea_enum/1  "VDKC_UWBDetArea_enum"
  Switch86/1 -> VDKC_OutputPCMDModule_enum/1  "VDKC_OutputPCMDModule_enum"
  Constant328/1 -> Switch86/1
  Constant327/1 -> Switch87/1
  Constant326/1 -> Switch88/1
  Constant325/1 -> Switch89/1
  Constant324/1 -> Switch90/1
  Constant323/1 -> Switch92/3
  Constant322/1 -> Switch92/1
  Constant321/1 -> Switch91/3
  [VDKC_UIDDetRSSIChgToLock_flg] -> Switch92/2
  Switch92/1 -> Switch91/1
  Switch91/1 -> Switch90/3
  Switch90/1 -> Switch89/3
  Switch89/1 -> Switch88/3
  Switch88/1 -> Switch87/3
  Switch87/1 -> Switch86/3
  [VDKC_UWBDetCmdLatch_flg] -> Switch91/2
  [VDKC_AutoLockCmdLatch_flg] -> Switch90/2
  [VDKC_PTGPCmdLatch_flg] -> Switch89/2
  [VDKC_NFCDetPCmdLatch_flg] -> Switch88/2
  [VDKC_TrunkHanPCmdLatch_flg] -> Switch87/2
  [VDKC_UIDButPCmdLatch_flg] -> Switch86/2
  VINP_DKCBTRSSI_dB/1 -> Switch78/1
  VINP_UIDBatVoltx1000_V/1 -> Switch76/1
  VINP_BTConnectSta_enum/1 -> Switch77/1
  PDkeyJudgeBatLowVolt_Chart/1(VDKC_UIDBatLowVolt_flg) -> Switch65/2  "VDKC_UIDBatLowVolt_flg"
  Logical Operator138/1 -> SR_Latch17/2(reset)
  Logical Operator140/1 -> Logical Operator138/1
  [VDKC_BTConnectSta_enum] -> Equal151/1, Detect Change42/1
  Constant262/1 -> Equal151/2
  Detect Change42/1 -> Logical Operator140/1
  Equal151/1 -> Logical Operator140/2
  Logical Operator133/1 -> Timer9/2(reset)
  [VDKC_FDCKeyAllowSleep_flg] -> Terminator2/1
  Switch51/1 -> [VDKC_FDCKeyAllowSleep_flg], VDKC_FDCKeyAllowSleep_flg/1  "VDKC_FDCKeyAllowSleep_flg"
  AllowSleep_Chart/1(VDKC_FDCKeyAllowSleep_flg) -> Switch51/3
  Constant221/1 -> Switch51/2
  Constant222/1 -> Switch51/1
  Logical Operator130/1 -> AllowSleep_Chart/2(VDKC_FDCDKCTimerActive_flg)  "VDKC_FDCDKCTimerActive_flg"
  Constant225/1 -> AllowSleep_Chart/1(KDKC_DKCAllowSleepDelayTime_s)
  [VPMM_PowerSta_enum] -> AllowSleep_Chart/4(VPMM_PowerSta_enum)
  [task_time_s] -> AllowSleep_Chart/3(task_time_s)
  Logical Operator129/1 -> Logical Operator130/4  "VDKC_DKCOtherTimerActive_flg"
  Logical Operator128/1 -> Logical Operator130/3  "VDKC_DKCAutoJudgTimerActive_flg"
  Logical Operator126/1 -> Logical Operator130/2  "VDKC_DKCTGTimerActive_flg"
  Logical Operator124/1 -> Logical Operator130/1  "VDKC_DKCCmdHandTimerActive_flg"
  [VDKC_LidADetGreenCardLatch4s_flg] -> Logical Operator129/2
  [VDKC_UWBDetChgWelcomeLatch_flg] -> Logical Operator129/1
  [VDKC_AutoLeavePSTimerLatch_flg] -> Logical Operator128/3
  [VDKC_UIDAutoLockTimerLatch_flg] -> Logical Operator128/2
  [VDKC_NFCAutoLockTimerLatch_flg] -> Logical Operator128/1
  [VDKC_RemTGCmdTimerLatch_flg] -> Logical Operator126/3
  [VDKC_InnerSW1TimerLatch_flg] -> Logical Operator126/2
  [VDKC_InnerSW2TimerLatch_flg] -> Logical Operator126/1
  Equal133/1 -> Logical Operator124/3
  Equal134/1 -> Logical Operator124/4
  Equal135/1 -> Logical Operator124/5
  Equal136/1 -> Logical Operator124/6
  Constant220/1 -> Equal136/2
  [VDKC_AutoLockPCmdHandSta_enum] -> Equal136/1
  Constant219/1 -> Equal135/2
  [VDKC_UWBDetPCmdHandSta_enum] -> Equal135/1
  Constant218/1 -> Equal134/2
  [VDKC_PTGPCmdHandSta_enum] -> Equal134/1
  Constant217/1 -> Equal133/2
  [VDKC_NFCDetPCmdHandSta_enum] -> Equal133/1
  Constant216/1 -> Equal132/2
  [VDKC_TrunkHanPCmdHandSta_enum] -> Equal132/1
  Equal132/1 -> Logical Operator124/2
  [VDKC_UIDButtonPCmdHandSta_enum] -> Equal130/1
  Constant196/1 -> Equal130/2
  Equal130/1 -> Logical Operator124/1
  Logical Operator60/1 -> [VDKC_PMMChgToReady_flg]  "VDKC_PMMChgToReady_flg"
  Unit Delay42/1 -> Data Type Conversion113/1
  [VDKC_UIDButtJudgeAutoLock_flg] -> Unit Delay42/1
  Unit Delay41/1 -> Data Type Conversion112/1
  [VDKC_NFCDetJudgeAutoLock_flg] -> Unit Delay41/1
  Logical Operator56/1 -> Logical Operator76/3
  Logical Operator110/1 -> Logical Operator76/4
  Switch47/1 -> AutoLock_PCMD_Chart/1(KDKC_LockCmdDelayTime_s)
  [VDKC_CANMsgValidZONEDRFR_flg] -> Switch47/2
  Constant48/1 -> Switch47/3
  Constant207/1 -> Switch47/1
  Switch49/1 -> UWB_PCMD_Chart/1(KDKC_LockCmdDelayTime_s)
  Switch50/1 -> UWB_PCMD_Chart/2(KDKC_UnlockCmdDelayTime_s)
  [VDKC_CANMsgValidZONEDRFR_flg] -> Switch50/2
  Constant140/1 -> Switch50/3
  Constant212/1 -> Switch50/1
  Constant211/1 -> Switch49/1
  Constant141/1 -> Switch49/3
  [VDKC_CANMsgValidZONEDRFR_flg] -> Switch49/2
  Switch46/1 -> PTG_PCMD_Chart/1(KDKC_LockCmdDelayTime_s)
  Constant159/1 -> Switch46/1
  Constant54/1 -> Switch46/3
  [VDKC_CANMsgValidZONEDRFR_flg] -> Switch46/2
  Switch45/1 -> NFC_PCMD_Chart/2(KDKC_UnlockCmdDelayTime_s)
  Constant106/1 -> Switch45/1
  Constant35/1 -> Switch45/3
  [VDKC_CANMsgValidZONEDRFR_flg] -> Switch45/2
  Switch44/1 -> TrunkHanSW_PCMD_Chart/1(KDKC_UnlockCmdDelayTime_s)
  [VDKC_CANMsgValidZONEDRFR_flg] -> Switch43/2
  Constant204/1 -> Switch43/3
  Constant205/1 -> Switch43/1
  Switch43/1 -> NFC_PCMD_Chart/1(KDKC_LockCmdDelayTime_s)
  Constant206/1 -> Switch44/1
  Constant101/1 -> Switch44/3
  [VDKC_CANMsgValidZONEDRFR_flg] -> Switch44/2
  [VDKC_CANMsgValidZONEDRFR_flg] -> Switch42/2
  Constant100/1 -> Switch42/3
  Constant203/1 -> Switch42/1
  Switch42/1 -> UIDButton_PCMD_Chart/2(KDKC_UnlockCmdDelayTime_s)
  Switch41/1 -> UIDButton_PCMD_Chart/1(KDKC_LockCmdDelayTime_s)
  Constant202/1 -> Switch41/1
  Constant199/1 -> Switch41/3
  [VDKC_CANMsgValidZONEDRFR_flg] -> Switch41/2
  VDKC_CANMsgValidZONEDRFR_flg/1 -> [VDKC_CANMsgValidZONEDRFR_flg]
  Equal55/1 -> Logical Operator101/5
  Equal54/1 -> Logical Operator101/4
  Equal49/1 -> Logical Operator31/5
  Equal48/1 -> Logical Operator31/4
  Equal51/1 -> Logical Operator31/3
  Equal44/1 -> Logical Operator88/5
  Equal43/1 -> Logical Operator88/4
  Equal81/1 -> Logical Operator88/3
  Equal40/1 -> Logical Operator28/5
  Equal39/1 -> Logical Operator28/4
  Equal42/1 -> Logical Operator28/3
  Equal35/1 -> Logical Operator105/5
  Equal34/1 -> Logical Operator105/4
  Equal75/1 -> Logical Operator105/3
  Switch26/1 -> Switch27/3
  Constant178/1 -> Switch26/3
  Switch27/1 -> Switch12/3
  Logical Operator35/1 -> Logical Operator127/3
  Constant198/1 -> Equal63/2
  Equal63/1 -> Logical Operator35/1
  [VDKC_UIDButtonPCmdToBCMRAW_enum] -> Unit Delay40/1
  Unit Delay40/1 -> Data Type Conversion85/1
  Data Type Conversion85/1 -> Equal63/1
  Logical Operator7/1 -> Logical Operator73/3
  Equal33/1 -> Logical Operator7/1
  [VDKC_UIDButtonPCmdToBCMRAW_enum] -> Unit Delay32/1
  Unit Delay32/1 -> Data Type Conversion72/1
  Constant197/1 -> Equal33/2
  Data Type Conversion72/1 -> Equal33/1
  Logical Operator57/1 -> Logical Operator73/1
  SR_Latch3/1 -> Logical Operator43/1, Logical Operator73/4
  Data Type Conversion71/1 -> Equal4/1
  Constant6/1 -> Equal4/2
  Equal4/1 -> Logical Operator6/1
  [VDKC_FDCPCommandToBCM_enum] -> Unit Delay10/1
  Unit Delay10/1 -> Data Type Conversion71/1
  Unit Delay9/1 -> Data Type Conversion69/1
  [VDKC_FDCPCommandToBCM_enum] -> Unit Delay9/1
  Equal10/1 -> Logical Operator72/1
  Constant126/1 -> Equal10/2
  Data Type Conversion69/1 -> Equal10/1
  Constant201/1 -> Switch19/3
  Constant200/1 -> Switch19/1
  [VDKC_NFCDetPCmdToBCMRAW_enum] -> Switch19/2
  Switch19/1 -> Switch25/1
  Logical Operator111/1 -> Logical Operator9/4
  Logical Operator127/1 -> Timer1/1(trigger), [VDKC_UIDAutoLockTimerLatch_flg]  "VDKC_UIDAutoLockTimerLatch_flg"
  Logical Operator125/1 -> Logical Operator127/1
  [VDKC_UWBDetWithinUnlockZone_flg] -> Logical Operator125/1
  Logical Operator72/1 -> Logical Operator73/2
  Data Type Conversion87/1 -> Logical Operator114/2
  [VINP_KeyFobAreaU16_enum] -> Extract Bits12/1
  Extract Bits12/1 -> Data Type Conversion87/1
  Data Type Conversion86/1 -> Logical Operator114/1
  Logical Operator114/1 -> Switch18/2
  Extract Bits15/1 -> Data Type Conversion86/1
  [VINP_KeyFobAreaU16_enum] -> Extract Bits15/1
  Data Type Conversion84/1 -> Switch2/2
  Switch1/1 -> VDKC_FDCKeyAreaSPTG_enum/1  "VDKC_FDCKeyAreaSPTG_enum"
  Constant19/1 -> Switch18/1
  Constant17/1 -> Switch18/3
  Switch2/1 -> Switch1/3
  Switch18/1 -> Switch2/3
  Constant21/1 -> Switch1/1
  Constant20/1 -> Switch1/2
  Extract Bits13/1 -> Data Type Conversion84/1
  [VINP_KeyFobAreaU16_enum] -> Extract Bits13/1
  Data Type Conversion45/1 -> Logical Operator112/3
  [VINP_KeyFobAreaU16_enum] -> Extract Bits11/1
  Extract Bits11/1 -> Data Type Conversion45/1
  VINP_BPPTGInsideSW1Sta_enum/1 -> [VINP_BPPTGInsideSW1Sta_enum]
  VINP_BPPTGInsideSW2Sta_enum/1 -> [VINP_BPPTGInsideSW2Sta_enum]
  [VTQD_GearActualPosn_enum] -> TrunkHanSW_PCMD_Chart/7(VDKC_GearActualPosn_enum)
  Equal59/1 -> Logical Operator77/1
  Equal122/1 -> Logical Operator77/2
  [VPMM_PowerSta_enum] -> Detect Change34/1, Equal117/1
  Constant84/1 -> Equal117/2
  Equal117/1 -> Logical Operator111/2
  Detect Change34/1 -> Logical Operator111/1
  Detect Change18/1 -> Logical Operator110/1
  [VPMM_PowerSta_enum] -> Equal60/1, Detect Change18/1
  Equal60/1 -> Logical Operator110/2
  Constant83/1 -> Equal60/2
  Detect Increase9/1 -> AutoLock_PCMD_Chart/4(VDKC_PMMChgToReady_flg)
  [VDKC_PMMChgToReady_flg] -> Detect Increase9/1
  Constant82/1 -> Equal58/2
  Equal58/1 -> Logical Operator60/2
  [VPMM_PowerSta_enum] -> Detect Change17/1, Equal58/1
  Detect Change17/1 -> Logical Operator60/1
  Data Type Conversion70/1 -> Equal30/1
  Data Type Conversion68/1 -> Equal5/1
  Data Type Conversion66/1 -> Detect Change7/1, Equal20/1
  Unit Delay12/1 -> Data Type Conversion66/1
  Data Type Conversion64/1 -> Detect Change8/1, Equal19/1
  Unit Delay3/1 -> Data Type Conversion64/1
  Data Type Conversion63/1 -> Detect Change9/1, Equal26/1
  Unit Delay7/1 -> Data Type Conversion63/1
  Constant80/1 -> Equal56/2
  [VBCM_AntitheftSta_enum] -> Detect Change16/1, Equal56/1
  Detect Change16/1 -> Logical Operator58/1
  Equal56/1 -> Logical Operator58/2
  Equal31/1 -> Logical Operator56/2
  Detect Change12/1 -> Logical Operator56/1
  [VBCM_AntitheftSta_enum] -> Equal31/1, Detect Change12/1
  Constant79/1 -> Equal31/2
  Logical Operator55/1 -> Timer3/2
  Logical Operator43/1 -> Logical Operator55/1
  Constant56/1 -> Equal30/2
  Equal30/1 -> Logical Operator55/2
  [VDKC_UIDButtonPCmdToBCMRAW_enum] -> Unit Delay1/1
  Unit Delay1/1 -> Data Type Conversion70/1
  [VDKC_UWBDetWithinUnlockZone_flg] -> Logical Operator57/1
  Unit Delay11/1 -> Data Type Conversion68/1
  [VDKC_UIDButtJudgeAutoLock_flg] -> Detect Increase2/1
  [VDKC_NFCDetJudgeAutoLock_flg] -> Detect Increase7/1
  [VDKC_PTGPCmdHandSta_enum] -> Data Type Conversion61/1
  Constant78/1 -> Equal55/2
  Data Type Conversion61/1 -> Equal55/1
  Data Type Conversion60/1 -> Equal54/1
  Constant77/1 -> Equal54/2
  [VDKC_TrunkHanPCmdHandSta_enum] -> Data Type Conversion60/1
  [VDKC_TrunkHanPCmdHandSta_enum] -> Data Type Conversion58/1
  Constant75/1 -> Equal52/2
  Data Type Conversion58/1 -> Equal52/1
  Data Type Conversion59/1 -> Equal53/1
  Constant76/1 -> Equal53/2
  [VDKC_PTGPCmdHandSta_enum] -> Data Type Conversion59/1
  Equal52/1 -> Logical Operator91/5
  Equal53/1 -> Logical Operator91/6
  Switch12/1 -> Switch25/3
  [VDKC_TrunkHanPCmdHandSta_enum] -> Data Type Conversion23/1
  Constant74/1 -> Equal49/2
  Data Type Conversion23/1 -> Equal49/1
  Data Type Conversion21/1 -> Equal48/1
  Constant73/1 -> Equal48/2
  [VDKC_UIDButtonPCmdHandSta_enum] -> Data Type Conversion21/1
  [VDKC_AutoLockPCmdHandSta_enum] -> Data Type Conversion57/1
  From83/1 -> Data Type Conversion56/1
  [VDKC_NFCDetPCmdHandSta_enum] -> Data Type Conversion24/1
  Constant68/1 -> Equal45/2
  Data Type Conversion24/1 -> Equal45/1
  Detect Decrease2/1 -> Logical Operator30/1
  Equal46/1 -> Logical Operator30/2
  Constant69/1 -> Equal46/2
  [VDKC_PTGPCmdToBCMRAW_enum] -> Detect Decrease2/1, Equal46/1
  Logical Operator30/1 -> SR_Latch10/2(reset)
  Equal45/1 -> Logical Operator31/2
  Logical Operator31/1 -> SR_Latch10/1(set)
  Logical Operator32/1 -> Logical Operator31/1
  Equal47/1 -> Logical Operator32/2
  Detect Change14/1 -> Logical Operator32/1
  Constant70/1 -> Equal47/2
  [VDKC_PTGPCmdToBCMRAW_enum] -> Equal47/1, Detect Change14/1
  SR_Latch10/1(latched) -> [VDKC_PTGPCmdLatch_flg], Switch12/2
  [VDKC_PTGPCmdToBCMRAW_enum] -> Switch12/1
  Data Type Conversion56/1 -> Equal50/1
  Constant71/1 -> Equal50/2
  Constant72/1 -> Equal51/2
  Data Type Conversion57/1 -> Equal51/1
  Switch25/1 -> Switch11/3
  [VDKC_TrunkHanPCmdHandSta_enum] -> Data Type Conversion19/1
  Constant66/1 -> Equal43/2
  Data Type Conversion19/1 -> Equal43/1
  Data Type Conversion20/1 -> Equal44/1
  Constant67/1 -> Equal44/2
  [VDKC_PTGPCmdHandSta_enum] -> Data Type Conversion20/1
  Data Type Conversion18/1 -> Equal42/1
  Constant63/1 -> Equal42/2
  Constant62/1 -> Equal41/2
  Data Type Conversion17/1 -> Equal41/1
  [VDKC_TrunkHanPCmdToBCMRAW_enum] -> Switch11/1
  SR_Latch9/1(latched) -> Switch11/2, [VDKC_TrunkHanPCmdLatch_flg]
  [VDKC_TrunkHanPCmdToBCMRAW_enum] -> Detect Change13/1, Equal38/1
  Constant61/1 -> Equal38/2
  Detect Change13/1 -> Logical Operator29/1
  Equal38/1 -> Logical Operator29/2
  Logical Operator29/1 -> Logical Operator28/1
  Logical Operator28/1 -> SR_Latch9/1(set)
  Equal36/1 -> Logical Operator28/2
  Logical Operator27/1 -> SR_Latch9/2(reset)
  [VDKC_TrunkHanPCmdToBCMRAW_enum] -> Equal37/1, Detect Decrease1/1
  Constant60/1 -> Equal37/2
  Equal37/1 -> Logical Operator27/2
  Detect Decrease1/1 -> Logical Operator27/1
  Data Type Conversion16/1 -> Equal36/1
  Constant59/1 -> Equal36/2
  Switch11/1 -> Switch30/3
  [VDKC_NFCDetPCmdHandSta_enum] -> Data Type Conversion16/1
  From73/1 -> Data Type Conversion17/1
  [VDKC_AutoLockPCmdHandSta_enum] -> Data Type Conversion18/1
  [VDKC_UIDButtonPCmdHandSta_enum] -> Data Type Conversion14/1
  Constant64/1 -> Equal39/2
  Data Type Conversion14/1 -> Equal39/1
  Data Type Conversion15/1 -> Equal40/1
  Constant65/1 -> Equal40/2
  [VDKC_PTGPCmdHandSta_enum] -> Data Type Conversion15/1
  [VDKC_PTGPCmdHandSta_enum] -> Data Type Conversion13/1
  Constant58/1 -> Equal35/2
  Data Type Conversion13/1 -> Equal35/1
  Data Type Conversion12/1 -> Equal34/1
  Constant57/1 -> Equal34/2
  [VDKC_TrunkHanPCmdHandSta_enum] -> Data Type Conversion12/1
  Equal15/1 -> Logical Operator15/3
  [VDKC_FDCKeyAreaPTG_enum] -> Equal15/1
  Constant11/1 -> Equal15/2
  Data Type Conversion9/1 -> [VDKC_TrunkHanPCmdHandSta_enum]  "VDKC_TrunkHanPCmdHandSta_enum"
  TrunkHanSW_PCMD_Chart/2(VDKC_TrunkHanUnlockPCmdHandingSta_enum) -> Data Type Conversion9/1
  TrunkHanSW_PCMD_Chart/1(VDKC_TrunkHanPCmdToBCMRAW_enum) -> Data Type Conversion8/1
  Data Type Conversion8/1 -> [VDKC_TrunkHanPCmdToBCMRAW_enum]  "VDKC_TrunkHanPCmdToBCMRAW_enum"
  [VINP_VehSpeed_kph] -> TrunkHanSW_PCMD_Chart/6(VDKC_VehSpeed_kph)
  [VBCM_AntitheftSta_enum] -> TrunkHanSW_PCMD_Chart/2(VBCM_AntitheftSta_enum)
  [task_time_s] -> TrunkHanSW_PCMD_Chart/4(task_time_s)
  [VDKC_DKCPCmdFallingEdge_flg] -> TrunkHanSW_PCMD_Chart/5(VDKC_PCmdFallingEdge_flg)
  Logical Operator15/1 -> [VDKC_TrunkHandleSW_flg]  "VDKC_TrunkHandleSW_flg"
  Equal14/1 -> Logical Operator15/2
  Detect Decrease17/1 -> Logical Operator15/1
  Constant10/1 -> Equal14/2
  [VINP_TrunkHanSW_flg] -> Detect Decrease17/1, Equal14/1
  VINP_TrunkHanSW_flg/1 -> [VINP_TrunkHanSW_flg]
  Constant33/1 -> Switch10/2
  Constant34/1 -> Switch10/1
  Constant32/1 -> Switch/1
  Constant31/1 -> Switch/2
  Switch/1 -> [VDKC_KeyUWBDetArea_enum], Data Type Conversion122/1  "VDKC_KeyUWBDetArea_enum"
  [VDKC_UIDButtonChargeCover_flg] -> UIDButton_PCMD_Chart/8(VDKC_UIDButtonChargeCover_flg)
  [VDKC_UIDBLEBatton_Cmd] -> Equal13/1, Detect Change5/1
  Constant30/1 -> Equal13/2
  Detect Change5/1 -> Logical Operator14/1
  Equal13/1 -> Logical Operator14/2
  Logical Operator14/1 -> [VDKC_UIDButtonChargeCover_flg]  "VDKC_UIDButtonChargeCover_flg"
  Logical Operator13/1 -> [VDKC_UIDButtonFrontHood_flg]  "VDKC_UIDButtonFrontHood_flg"
  Equal12/1 -> Logical Operator13/2
  Detect Change4/1 -> Logical Operator13/1
  Constant29/1 -> Equal12/2
  [VDKC_UIDBLEBatton_Cmd] -> Detect Change4/1, Equal12/1
  [VINP_KeyFobAreaU16_enum] -> Extract Bits5/1
  Extract Bits5/1 -> Data Type Conversion7/1
  Constant26/1 -> Switch8/1
  Switch9/1 -> Switch8/3
  [VINP_KeyFobAreaU16_enum] -> Switch9/2
  Switch8/1 -> Switch10/3
  Switch3/1 -> Switch/3
  Switch13/1 -> Switch7/3
  Switch7/1 -> Switch6/3
  Constant24/1 -> Switch7/1
  Data Type Conversion6/1 -> Switch7/2
  Extract Bits4/1 -> Data Type Conversion6/1
  [VINP_KeyFobAreaU16_enum] -> Extract Bits4/1
  [VINP_KeyFobAreaU16_enum] -> Extract Bits3/1
  [VINP_KeyFobAreaU16_enum] -> Extract Bits2/1
  [VINP_KeyFobAreaU16_enum] -> Extract Bits1/1
  Extract Bits1/1 -> Data Type Conversion3/1
  Switch6/1 -> Switch5/3
  Extract Bits3/1 -> Data Type Conversion5/1
  Data Type Conversion5/1 -> Switch6/2
  Constant23/1 -> Switch6/1
  Switch5/1 -> Switch4/3
  Constant22/1 -> Switch5/1
  Data Type Conversion4/1 -> Switch5/2
  Extract Bits2/1 -> Data Type Conversion4/1
  Switch4/1 -> Switch3/3
  Data Type Conversion3/1 -> Switch4/2
  Constant16/1 -> Switch4/1
  Constant15/1 -> Switch3/1
  Data Type Conversion2/1 -> Switch3/2
  Extract Bits/1 -> Data Type Conversion2/1
  [VINP_KeyFobAreaU16_enum] -> Extract Bits/1
  VTQD_GearActualPosn_enum/1 -> [VTQD_GearActualPosn_enum]
  [VTQD_GearActualPosn_enum] -> UIDButton_PCMD_Chart/13(VDKC_GearActualPosn_enum)
  [VINP_VehSpeed_kph] -> UIDButton_PCMD_Chart/12(VDKC_VehSpeed_kph)
  [VDKC_UIDButtonCarSearch_flg] -> UIDButton_PCMD_Chart/9(VDKC_UIDButtonCarSearch_flg)
  Switch84/1 -> UIDButton_PCMD_Chart/7(VDKC_UIDButtonRemTailGate_flg)
  VINP_VehSpeed_kph/1 -> [VINP_VehSpeed_kph]
  Logical Operator12/1 -> [VDKC_UIDButtonCarSearch_flg]  "VDKC_UIDButtonCarSearch_flg"
  Equal9/1 -> Logical Operator12/2
  Detect Change3/1 -> Logical Operator12/1
  Constant14/1 -> Equal9/2
  [VDKC_UIDBLEBatton_Cmd] -> Detect Change3/1, Equal9/1
  [VDKC_UIDBLEBatton_Cmd] -> Equal8/1, Detect Change2/1
  Constant13/1 -> Equal8/2
  Detect Change2/1 -> Logical Operator11/1
  Equal8/1 -> Logical Operator11/2
  Logical Operator11/1 -> [VDKC_UIDButtonRemTailGate_flg]  "VDKC_UIDButtonRemTailGate_flg"
  VINP_KeyFobAreaU16_enum/1 -> [VINP_KeyFobAreaU16_enum]
  VINP_UIDButtonCmd_enum/1 -> [VDKC_UIDBLEBatton_Cmd]
  [VDKC_NFCDetPCmdHandSta_enum] -> Data Type Conversion48/1
  [VDKC_UIDButtonPCmdHandSta_enum] -> Data Type Conversion35/1
  From101/1 -> Data Type Conversion49/1
  [VDKC_AutoLockPCmdHandSta_enum] -> Data Type Conversion47/1
  [VDKC_NFCDetPCmdHandSta_enum] -> Data Type Conversion46/1
  [VDKC_UIDButtonPCmdHandSta_enum] -> Data Type Conversion29/1
  [VDKC_AutoLockPCmdHandSta_enum] -> Data Type Conversion44/1
  From185/1 -> Data Type Conversion43/1
  [VDKC_UIDButtonPCmdHandSta_enum] -> Data Type Conversion51/1
  [VDKC_AutoLockPCmdHandSta_enum] -> Data Type Conversion42/1
  From153/1 -> Data Type Conversion41/1
  [VDKC_NFCDetPCmdHandSta_enum] -> Data Type Conversion37/1
  Constant157/1 -> Switch29/3
  Constant158/1 -> Switch29/1
  Data Type Conversion1/1 -> Logical Operator10/2
  Detect Increase2/1 -> Data Type Conversion1/1
  Data Type Conversion33/1 -> Logical Operator10/1
  Logical Operator10/1 -> AutoLock_PCMD_Chart/3(VDKC_AutoLockReqtoLock_flg)  "VDKC_AutoLockReqtoLock_flg"
  [VDKC_UIDButtonPCmdToBCMRAW_enum] -> Unit Delay11/1
  Detect Change1/1 -> Logical Operator1/2
  Timer1/1(time) -> Relational Operator1/1
  Logical Operator9/1 -> SR_Latch6/2(reset)
  Relational Operator1/1 -> [VDKC_UIDButtJudgeAutoLock_flg]  "VDKC_UIDButtJudgeAutoLock_flg"
  Logical Operator5/1 -> Timer1/2(reset)
  Logical Operator1/1 -> SR_Latch6/1(set)
  Equal6/1 -> Logical Operator1/3
  [task_time_s] -> Timer1/3(Ts)
  Equal5/1 -> Logical Operator5/2
  [VDKC_AnyDoorSta_flg] -> Logical Operator3/1, Logical Operator9/1
  [VBCM_AntitheftSta_enum] -> Equal6/1, Detect Change1/1
  SR_Latch6/1(latched) -> Logical Operator127/4, Logical Operator4/1
  Constant5/1 -> Equal6/2
  Logical Operator4/1 -> Logical Operator5/1
  Constant9/1 -> Equal5/2
  Logical Operator3/1 -> Logical Operator1/4
  Equal3/1 -> Logical Operator1/1
  [VDKC_UIDButtonPCmdToBCMRAW_enum] -> Equal3/1
  Constant8/1 -> Equal3/2
  Constant4/1 -> Relational Operator1/2
  Constant3/1 -> Timer1/4(max_time)
  Logical Operator2/1 -> [VDKC_UWBDetWithinUnlockZone_flg]  "VDKC_UWBDetWithinUnlockZone_flg"
  Constant2/1 -> Equal1/2
  [VDKC_KeyUWBDetArea_enum] -> Equal1/1
  Equal1/1 -> Logical Operator2/1
  [VDKC_KeyUWBDetArea_enum] -> Equal2/1
  Constant1/1 -> Equal2/2
  Equal2/1 -> Logical Operator2/2
  Constant115/1 -> Timer3/4
  Constant116/1 -> Relational Operator2/2
  SR_Latch2/1(latched) -> Switch25/2, [VDKC_NFCDetPCmdLatch_flg]
  UIDButton_PCMD_Chart/1(VDKC_UIDButtonPCmdToBCMRAW_enum) -> Data Type Conversion36/1
  UIDButton_PCMD_Chart/2(VDKC_UIDButtonPCmdHandingSta_enum) -> Data Type Conversion34/1
  Switch30/1 -> Data Type Conversion54/1
  Constant103/1 -> Equal105/2
  Data Type Conversion37/1 -> Equal105/1
  Detect Decrease9/1 -> Logical Operator102/1
  Equal106/1 -> Logical Operator102/2
  Constant104/1 -> Equal106/2
  [VDKC_UIDButtonPCmdToBCMRAW_enum] -> Detect Decrease9/1, Equal106/1
  Logical Operator102/1 -> SR_Latch1/2(reset)
  Equal105/1 -> Logical Operator105/2
  Logical Operator105/1 -> SR_Latch1/1(set)
  Logical Operator106/1 -> Logical Operator105/1
  Equal108/1 -> Logical Operator106/2
  Detect Change25/1 -> Logical Operator106/1
  Constant105/1 -> Equal108/2
  [VDKC_UIDButtonPCmdToBCMRAW_enum] -> Equal108/1, Detect Change25/1
  SR_Latch1/1(latched) -> Switch30/2, [VDKC_UIDButPCmdLatch_flg]
  [VDKC_UIDButtonPCmdToBCMRAW_enum] -> Switch30/1
  [VPMM_PowerSta_enum] -> UIDButton_PCMD_Chart/11(VPMM_PowerSta_enum)
  [task_time_s] -> UIDButton_PCMD_Chart/10(task_time_s)
  [VDKC_UIDButtonLock_flg] -> UIDButton_PCMD_Chart/4(VDKC_UIDButtonLock_flg)
  [VDKC_UIDButtonUnlock_flg] -> UIDButton_PCMD_Chart/3(VDKC_UIDButtonUnlock_flg)
  Data Type Conversion36/1 -> [VDKC_UIDButtonPCmdToBCMRAW_enum]  "VDKC_UIDButtonPCmdToBCMRAW_enum"
  Data Type Conversion34/1 -> [VDKC_UIDButtonPCmdHandSta_enum]  "VDKC_UIDButtonPCmdHandSta_enum"
  [VDKC_DKCPCmdFallingEdge_flg] -> UIDButton_PCMD_Chart/14(VDKC_PCmdFallingEdge_flg)
  Logical Operator100/1 -> [VDKC_UIDButtonUnlock_flg]  "VDKC_UIDButtonUnlock_flg"
  Equal103/1 -> Logical Operator100/2
  Detect Change24/1 -> Logical Operator100/1
  Constant179/1 -> Equal103/2
  [VDKC_UIDBLEBatton_Cmd] -> Detect Change24/1, Equal103/1
  [VDKC_UIDBLEBatton_Cmd] -> Equal107/1, Detect Change23/1
  Constant102/1 -> Equal107/2
  Detect Change23/1 -> Logical Operator104/1
  Equal107/1 -> Logical Operator104/2
  Logical Operator104/1 -> [VDKC_UIDButtonLock_flg]  "VDKC_UIDButtonLock_flg"
  Constant53/1 -> Equal102/2
  [VDKC_NFCDetPCmdToBCMRAW_enum] -> Equal102/1
  Equal102/1 -> Logical Operator38/1
  SR_Latch5/1(latched) -> Switch27/2, [VDKC_AutoLockCmdLatch_flg]
  Constant153/1 -> Equal104/2
  Detect Change21/1 -> Logical Operator103/1
  Equal104/1 -> Logical Operator103/2
  Logical Operator103/1 -> Logical Operator101/1
  Logical Operator101/1 -> SR_Latch5/1(set)
  Equal85/1 -> Logical Operator101/2
  Logical Operator93/1 -> SR_Latch5/2(reset)
  [VDKC_AutoLockPCmdToBCMRAW_enum] -> Equal87/1, Detect Decrease7/1
  Equal87/1 -> Logical Operator93/2
  Detect Decrease7/1 -> Logical Operator93/1
  Data Type Conversion35/1 -> Equal85/1
  Constant149/1 -> Equal85/2
  Constant151/1 -> Equal87/2
  [VDKC_AutoLockPCmdToBCMRAW_enum] -> Equal104/1, Detect Change21/1
  Detect Increase7/1 -> Data Type Conversion33/1
  AutoLock_PCMD_Chart/1(VDKC_AutoLockPCmdToBCMRAW_enum) -> Data Type Conversion32/1
  AutoLock_PCMD_Chart/2(VDKC_AutoLockPCmdHandingSta_enum) -> Data Type Conversion30/1
  [VPMM_PowerSta_enum] -> AutoLock_PCMD_Chart/6(VPMM_PowerSta_enum)
  [VDKC_DKCPCmdFallingEdge_flg] -> AutoLock_PCMD_Chart/7(VDKC_PCmdFallingEdge_flg)
  [task_time_s] -> AutoLock_PCMD_Chart/5(task_time_s)
  [VBCM_AntitheftSta_enum] -> AutoLock_PCMD_Chart/2(VBCM_AntitheftSta_enum)
  Data Type Conversion30/1 -> [VDKC_AutoLockPCmdHandSta_enum]  "VDKC_AutoLockPCmdHandSta_enum"
  Data Type Conversion32/1 -> [VDKC_AutoLockPCmdToBCMRAW_enum]  "VDKC_AutoLockPCmdToBCMRAW_enum"
  [VDKC_AutoLockPCmdToBCMRAW_enum] -> Switch27/1
  Data Type Conversion54/1 -> [VDKC_FDCPCommandToBCM_enum], VDKC_FDCPCommandToBCM_enum/1  "VDKC_FDCPCommandToBCM_enum"
  Constant177/1 -> Switch28/3
  Constant176/1 -> Switch28/1
  Constant174/1 -> Equal101/2
  Constant173/1 -> Equal100/2
  [VDKC_UWBDetPEZoneKeepSta_enum] -> Equal101/1
  [VDKC_NFCJudgePEZoneSta_enum] -> Equal100/1
  Constant172/1 -> Switch21/1
  [VDKC_NFCJudgePEZoneSta_enum] -> Equal97/1
  [VDKC_UWBDetPEZoneKeepSta_enum] -> Equal98/1
  Constant167/1 -> Equal97/2
  Constant171/1 -> Equal98/2
  Switch21/1 -> VDKC_FDCKeyAreaLockUnlock_enum/1  "VDKC_FDCKeyAreaLockUnlock_enum"
  Logical Operator98/1 -> Switch21/2
  Equal97/1 -> Logical Operator98/1
  Equal98/1 -> Logical Operator98/2
  Switch28/1 -> Switch21/3
  Equal101/1 -> Logical Operator99/2
  Equal100/1 -> Logical Operator99/1
  Logical Operator99/1 -> Switch28/2
  Constant166/1 -> Equal115/2
  Constant170/1 -> Switch20/3
  Constant169/1 -> Switch20/1
  Equal96/1 -> Logical Operator97/2
  Constant165/1 -> Equal96/2
  [VDKC_KeyUWBDetArea_enum] -> Equal96/1
  Equal95/1 -> Logical Operator97/1
  Logical Operator97/1 -> Switch35/2
  Constant168/1 -> Switch35/1
  [VDKC_KeyUWBDetArea_enum] -> Equal95/1
  Constant175/1 -> Equal95/2
  Switch35/1 -> [VDKC_UWBDetPEZoneSta_enum]  "VDKC_UWBDetPEZoneSta_enum"
  Switch20/1 -> Switch35/3
  [VDKC_KeyUWBDetArea_enum] -> Equal115/1
  Equal115/1 -> Switch20/2
  Switch33/1 -> VDKC_FDCKeyAreaPS_enum/1, [VDKC_FDCKeyAreaPS_enum]  "VDKC_FDCKeyAreaPS_enum"
  Constant163/1 -> Switch34/3
  Constant162/1 -> Switch34/1
  Logical Operator95/1 -> Switch34/2
  Constant160/1 -> Equal93/2
  [VDKC_NFCJudgePSZoneSta_enum] -> Equal93/1
  Equal93/1 -> Logical Operator95/1
  Constant161/1 -> Equal94/2
  [VDKC_UWBDetPSZoneKeepSta_enum] -> Equal94/1
  Equal94/1 -> Logical Operator95/2
  Switch34/1 -> Switch33/3
  Constant154/1 -> Switch33/1
  Equal92/1 -> Logical Operator94/2
  [VDKC_UWBDetPSZoneKeepSta_enum] -> Equal92/1
  Constant150/1 -> Equal92/2
  Equal91/1 -> Logical Operator94/1
  [VDKC_NFCJudgePSZoneSta_enum] -> Equal91/1
  Constant118/1 -> Equal91/2
  Logical Operator94/1 -> Switch33/2
  Constant156/1 -> Switch15/1
  Logical Operator70/1 -> Logical Operator37/3
  Constant155/1 -> Equal90/2
  Equal90/1 -> Logical Operator70/2
  [VDKC_NFCJudgePSZoneSta_enum] -> Detect Change22/1, Equal90/1
  Detect Change22/1 -> Logical Operator70/1
  Equal86/1 -> Switch29/2
  Constant120/1 -> Equal86/2
  [VDKC_KeyUWBDetArea_enum] -> Equal86/1
  Switch29/1 -> Switch15/3
  Switch15/1 -> [VDKC_UWBDetPSZoneSta_enum]  "VDKC_UWBDetPSZoneSta_enum"
  [VDKC_DKCPCmdFallingEdge_flg] -> UWB_PCMD_Chart/12(VDKC_PCmdFallingEdge_flg)
  [VDKC_DKCPCmdFallingEdge_flg] -> NFC_PCMD_Chart/7(VDKC_PCmdFallingEdge_flg)
  Unit Delay17/1 -> Data Type Conversion31/1
  [VDKC_FDCPCommandToBCM_enum] -> Unit Delay17/1
  Data Type Conversion31/1 -> Equal89/1, Detect Decrease8/1
  Logical Operator86/1 -> [VDKC_DKCPCmdFallingEdge_flg]  "VDKC_DKCPCmdFallingEdge_flg"
  Constant98/1 -> Equal89/2
  Detect Decrease8/1 -> Logical Operator86/1
  Equal89/1 -> Logical Operator86/2
  [VDKC_UWBDetPCmdToBCMRAW_enum] -> Detect Change20/1, Equal84/1
  Constant147/1 -> Equal83/2
  [VDKC_UWBDetPCmdToBCMRAW_enum] -> Switch26/1
  Constant146/1 -> Equal82/2
  Data Type Conversion29/1 -> Equal82/1
  Detect Decrease6/1 -> Logical Operator90/1
  Equal83/1 -> Logical Operator90/2
  [VDKC_UWBDetPCmdToBCMRAW_enum] -> Detect Decrease6/1, Equal83/1
  Logical Operator90/1 -> SR_Latch4/2(reset)
  Equal82/1 -> Logical Operator91/2
  Logical Operator91/1 -> SR_Latch4/1(set)
  Logical Operator92/1 -> Logical Operator91/1
  Equal84/1 -> Logical Operator92/2
  Detect Change20/1 -> Logical Operator92/1
  Constant148/1 -> Equal84/2
  SR_Latch4/1(latched) -> Switch26/2, [VDKC_UWBDetCmdLatch_flg]
  [VDKC_NFCDetPCmdToBCMRAW_enum] -> Detect Change19/1, Equal79/1
  Constant145/1 -> Equal79/2
  Detect Change19/1 -> Logical Operator89/1
  Equal79/1 -> Logical Operator89/2
  Logical Operator89/1 -> Logical Operator88/1
  Logical Operator88/1 -> SR_Latch2/1(set)
  Equal76/1 -> Logical Operator88/2
  Logical Operator87/1 -> SR_Latch2/2(reset)
  [VDKC_NFCDetPCmdToBCMRAW_enum] -> Equal78/1, Detect Decrease5/1
  Constant144/1 -> Equal78/2
  Equal78/1 -> Logical Operator87/2
  Detect Decrease5/1 -> Logical Operator87/1
  Data Type Conversion51/1 -> Equal76/1
  Constant142/1 -> Equal76/2
  NFC_PCMD_Chart/2(VDKC_NFCPCmdHandingSta_enum) -> Data Type Conversion27/1
  NFC_PCMD_Chart/1(VDKC_NFCPCmdToBCMRAW_enum) -> Data Type Conversion28/1
  Data Type Conversion28/1 -> [VDKC_NFCDetPCmdToBCMRAW_enum]  "VDKC_NFCDetPCmdToBCMRAW_enum"
  Data Type Conversion27/1 -> [VDKC_NFCDetPCmdHandSta_enum]  "VDKC_NFCDetPCmdHandSta_enum"
  Data Type Conversion26/1 -> [VDKC_UWBDetPCmdHandSta_enum]  "VDKC_UWBDetPCmdHandSta_enum"
  UWB_PCMD_Chart/2(VDKC_UWBPCmdHandingSta_enum) -> Data Type Conversion26/1
  Data Type Conversion40/1 -> [VDKC_UWBDetPCmdToBCMRAW_enum]  "VDKC_UWBDetPCmdToBCMRAW_enum"
  UWB_PCMD_Chart/1(VDKC_UWBPCmdToBCMRAW_enum) -> Data Type Conversion40/1
  [task_time_s] -> UWB_PCMD_Chart/9(task_time_s)
  [VPMM_PowerSta_enum] -> UWB_PCMD_Chart/10(VPMM_PowerSta_enum)
  [VBCM_AntitheftSta_enum] -> UWB_PCMD_Chart/3(VBCM_AntitheftSta_enum)
  Logical Operator85/1 -> Logical Operator82/2
  Logical Operator84/1 -> Logical Operator85/2
  Logical Operator83/1 -> Logical Operator85/1
  Equal69/1 -> Logical Operator84/2
  Detect Change11/1 -> Logical Operator84/1
  Constant134/1 -> Equal69/2
  Constant137/1 -> Equal71/2
  Constant138/1 -> Equal72/2
  Equal71/1 -> Logical Operator81/1
  Equal72/1 -> Logical Operator81/2
  Logical Operator81/1 -> Logical Operator82/1
  Unit Delay21/1 -> Data Type Conversion55/1
  Data Type Conversion55/1 -> Equal71/1
  Data Type Conversion38/1 -> Equal72/1
  Unit Delay19/1 -> Data Type Conversion38/1
  Constant139/1 -> Equal73/2
  Detect Change33/1 -> Logical Operator83/1
  Equal73/1 -> Logical Operator83/2
  Logical Operator82/1 -> [VDKC_UWBDetAreaChangeToLock_flg]  "VDKC_UWBDetAreaChangeToLock_flg"
  Logical Operator79/1 -> [VDKC_UWBDetAreaChaToUnlock_flg]  "VDKC_UWBDetAreaChaToUnlock_flg"
  Logical Operator80/1 -> Logical Operator79/2
  Equal70/1 -> Logical Operator80/2
  Detect Change32/1 -> Logical Operator80/1
  Constant136/1 -> Equal70/2
  Unit Delay18/1 -> Data Type Conversion53/1
  Data Type Conversion53/1 -> Equal68/1
  Data Type Conversion52/1 -> Equal59/1
  Unit Delay39/1 -> Data Type Conversion52/1
  Logical Operator77/1 -> Logical Operator79/1
  Constant133/1 -> Equal68/2
  Constant132/1 -> Equal59/2
  Equal67/1 -> Logical Operator37/1, Logical Operator61/1
  Logical Operator39/1 -> Logical Operator38/4
  [VDKC_NFCLidARisingEdge_flg] -> Logical Operator109/2
  Constant123/1 -> Equal61/2
  Data Type Conversion50/1 -> Switch24/3
  Logical Operator75/1 -> SR_Latch7/1
  Switch32/1 -> Switch31/3
  [VBCM_AntitheftSta_enum] -> Detect Change27/1, Equal61/1
  Constant91/1 -> Equal28/2
  [VDKC_AnyDoorSta_flg] -> Logical Operator39/1, Logical Operator76/1
  Detect Change28/1 -> Logical Operator63/1
  Logical Operator62/1 -> Logical Operator109/1
  Unit Delay37/1 -> Data Type Conversion50/1
  Logical Operator61/1 -> Logical Operator75/2
  Constant128/1 -> Equal65/2
  SR_Latch7/1 -> Logical Operator65/2, Logical Operator62/1
  [task_time_s] -> Timer3/3
  Equal65/1 -> Logical Operator63/2
  Equal61/1 -> Logical Operator38/3
  Logical Operator38/1 -> SR_Latch3/1
  Constant99/1 -> Switch36/1
  [VPMM_PowerSta_enum] -> Equal67/1
  [VDKC_NFCLidARisingEdge_flg] -> Switch36/2
  Constant95/1 -> Switch32/1
  Constant121/1 -> Switch23/1
  Timer4/1 -> Relational Operator3/1
  Data Type Conversion25/1 -> Switch22/3
  [VDKC_NFCDetPCmdToBCMRAW_enum] -> Equal28/1
  Constant127/1 -> Switch24/1
  Relational Operator2/1 -> [VDKC_NFCDetJudgeAutoLock_flg]  "VDKC_NFCDetJudgeAutoLock_flg"
  [VDKC_PMMEnterOFF_flg] -> Switch24/2
  Logical Operator76/1 -> SR_Latch3/2
  [VDKC_NFCDetPCmdToBCMRAW_enum] -> Equal32/1
  Constant119/1 -> Relational Operator3/2
  Constant129/1 -> Equal67/2
  Constant93/1 -> Equal32/2
  Switch31/1 -> Unit Delay37/1, [VDKC_NFCJudgePEZoneSta_enum]  "VDKC_NFCJudgePEZoneSta_enum"
  Constant94/1 -> Switch31/1
  Detect Increase6/1 -> Switch32/2
  Relational Operator3/1 -> [VDKC_NFCJudgeAutoLeavePS_flg]  "VDKC_NFCJudgeAutoLeavePS_flg"
  Switch36/1 -> Unit Delay36/1, [VDKC_NFCJudgePSZoneSta_enum]  "VDKC_NFCJudgePSZoneSta_enum"
  Logical Operator67/1 -> Detect Increase1/1
  Switch23/1 -> Switch36/3
  Equal28/1 -> Logical Operator67/1
  [task_time_s] -> Timer4/3
  [VDKC_NFCLidARisingEdge_flg] -> Logical Operator67/2
  Logical Operator107/1 -> Detect Increase16/1
  Constant117/1 -> Timer4/4
  [VDKC_NFCJudgeAutoLeavePS_flg] -> Unit Delay34/1
  [VDKC_PMMLeaveREADY_flg] -> Logical Operator107/1
  Unit Delay36/1 -> Data Type Conversion25/1
  Constant164/1 -> Switch22/1
  Timer3/1 -> Relational Operator2/1
  Switch24/1 -> Switch32/3
  Switch22/1 -> Switch23/3
  Detect Change27/1 -> Logical Operator38/2
  Detect Increase1/1 -> Switch31/2
  Logical Operator109/1 -> Timer4/2
  Logical Operator37/1 -> SR_Latch7/2
  Logical Operator63/1 -> Logical Operator75/1
  Detect Change29/1 -> Logical Operator64/1
  [VDKC_FDCKeyAreaPS_enum] -> Equal27/1, Detect Change29/1
  Equal27/1 -> Logical Operator64/2
  Constant92/1 -> Equal27/2
  Logical Operator64/1 -> Logical Operator37/2
  [VDKC_NFCJudgePSZoneSta_enum] -> Detect Change28/1, Equal65/1
  [VDKC_NFCLidARisingEdge_flg] -> Logical Operator66/1
  Logical Operator65/1 -> Timer4/1, [VDKC_AutoLeavePSTimerLatch_flg]  "VDKC_AutoLeavePSTimerLatch_flg"
  Logical Operator66/1 -> Logical Operator65/1
  Logical Operator96/1 -> Switch22/2
  [VDKC_PMMEnterOFFC_flg] -> Logical Operator96/3
  [VDKC_PMMCrash_flg] -> Logical Operator96/4
  [VDKC_PMMEnterOFF_flg] -> Logical Operator96/1
  [VDKC_PMMEnterOFFA_flg] -> Logical Operator96/2
  Logical Operator73/1 -> Timer3/1, [VDKC_NFCAutoLockTimerLatch_flg]  "VDKC_NFCAutoLockTimerLatch_flg"
  Equal116/1 -> Switch15/2
  Constant97/1 -> Equal116/2
  [VDKC_KeyUWBDetArea_enum] -> Equal116/1
  Logical Operator74/1 -> Logical Operator71/1
  Equal99/1 -> Logical Operator74/1
  Equal110/1 -> Logical Operator74/2
  Data Type Conversion22/1 -> Equal99/2, Equal110/1
  Constant143/1 -> Equal110/2
  Constant152/1 -> Equal99/1
  Unit Delay16/1 -> Data Type Conversion22/1
  Constant135/1 -> Equal88/2
  Logical Operator71/1 -> [VDKC_PMMCrash_flg]  "VDKC_PMMCrash_flg"
  Equal88/1 -> Logical Operator71/2
  [VPMM_PowerSta_enum] -> Unit Delay16/1, Equal88/1
  [VPMM_PowerSta_enum] -> Equal77/1, Detect Change31/1
  Equal77/1 -> Logical Operator69/2
  Logical Operator69/1 -> [VDKC_PMMEnterOFFC_flg]  "VDKC_PMMEnterOFFC_flg"
  Detect Change31/1 -> Logical Operator69/1
  Constant124/1 -> Equal77/2
  Constant96/1 -> Equal66/2
  Equal66/1 -> Logical Operator68/2
  Logical Operator68/1 -> [VDKC_PMMEnterOFFA_flg]  "VDKC_PMMEnterOFFA_flg"
  [VPMM_PowerSta_enum] -> Equal66/1, Detect Change30/1
  Detect Change30/1 -> Logical Operator68/1
  Detect Change26/1 -> Logical Operator78/1
  Detect Change10/1 -> Logical Operator108/1
  Constant122/1 -> Equal62/2
  [VPMM_PowerSta_enum] -> Detect Change10/1, Equal64/1
  Data Type Conversion39/1 -> Equal62/1
  Logical Operator78/1 -> [VDKC_PMMLeaveREADY_flg]  "VDKC_PMMLeaveREADY_flg"
  Logical Operator108/1 -> [VDKC_PMMEnterOFF_flg]  "VDKC_PMMEnterOFF_flg"
  [VDKC_NFCDoorRisingEdge_flg] -> NFC_PCMD_Chart/4(VDKC_DetectNFCRisingEdge_flg)
  Equal64/1 -> Logical Operator108/2
  [VBCM_AntitheftSta_enum] -> NFC_PCMD_Chart/3(VBCM_AntitheftSta_enum)
  Constant125/1 -> Equal64/2
  [VPMM_PowerSta_enum] -> NFC_PCMD_Chart/6(VPMM_PowerSta_enum)
  Unit Delay35/1 -> Data Type Conversion39/1
  Equal62/1 -> Logical Operator78/2
  [task_time_s] -> NFC_PCMD_Chart/5(task_time_s)
  [VPMM_PowerSta_enum] -> Detect Change26/1, Unit Delay35/1
  Data Type Conversion41/1 -> Equal74/1
  Constant107/1 -> Equal74/2
  Constant108/1 -> Equal75/2
  Data Type Conversion42/1 -> Equal75/1
  Constant109/1 -> Equal80/2
  Data Type Conversion43/1 -> Equal80/1
  Data Type Conversion44/1 -> Equal81/1
  Constant110/1 -> Equal81/2
  Data Type Conversion46/1 -> Equal109/1
  Constant111/1 -> Equal109/2
  Constant112/1 -> Equal111/2
  Data Type Conversion47/1 -> Equal111/1
  Equal109/1 -> Logical Operator91/3
  Equal111/1 -> Logical Operator91/4
  Constant113/1 -> Equal112/2
  Data Type Conversion48/1 -> Equal112/1
  Equal112/1 -> Logical Operator101/3
  Data Type Conversion49/1 -> Equal113/1
  Constant114/1 -> Equal113/2
  task_time_s/1 -> [task_time_s]
  VPMM_PowerSta_enum/1 -> [VPMM_PowerSta_enum]
  VBCM_AntitheftSta_enum/1 -> [VBCM_AntitheftSta_enum]
  VINP_DrDoorSW_flg/1 -> [VINP_DrDoorSW_flg], Logical Operator8/1
  VINP_RRDoorSW_flg/1 -> Logical Operator8/3
  VINP_NFCLidASta_flg/1 -> Detect Increase4/1
  VINP_NFCDoorSta_flg/1 -> Detect Increase/1
  VINP_RLDoorSW_flg/1 -> Logical Operator8/4
  VINP_PsDoorSW_flg/1 -> Logical Operator8/2
  VINP_TailgateSW_flg/1 -> Logical Operator8/5, [VINP_TailgateSW_flg]
  Detect Increase/1 -> [VDKC_NFCDoorRisingEdge_flg]  "VDKC_NFCDoorRisingEdge_flg"
  Logical Operator8/1 -> [VDKC_AnyDoorSta_flg]  "VDKC_AnyDoorSta_flg"
  Detect Increase4/1 -> [VDKC_NFCLidARisingEdge_flg]  "VDKC_NFCLidARisingEdge_flg"
  Constant12/1 -> Switch9/3
  Constant27/1 -> Switch9/1
  Switch10/1 -> [VDKC_FDCKeyAreaPTG_enum], VDKC_FDCKeyAreaPTG_enum/1  "VDKC_FDCKeyAreaPTG_enum"
  Constant44/1 -> Equal22/2
  [VDKC_UWBDetPSZoneKeepSta_enum] -> Equal22/1
  Logical Operator45/1 -> [VDKC_TGFalEdgeInPS_flg]  "VDKC_TGFalEdgeInPS_flg"
  [VINP_TailgateSW_flg] -> Detect Decrease12/1
  Detect Increase8/1 -> Logical Operator26/1
  Constant45/1 -> Relational Operator5/2
  SR_Latch8/1(latched) -> Logical Operator36/1, [VDKC_PressSW1Latch_flg]  "VDKC_PressSW1Latch_flg"
  Logical Operator36/1 -> Timer5/1(trigger), [VDKC_InnerSW1TimerLatch_flg]  "VDKC_InnerSW1TimerLatch_flg"
  Logical Operator40/1 -> Logical Operator36/2
  Logical Operator17/1 -> Timer5/2(reset), Logical Operator40/1
  Timer5/1(time) -> Relational Operator5/1
  Relational Operator5/1 -> [VDKC_InnerSW1CloseTimeOut_flg]  "VDKC_InnerSW1CloseTimeOut_flg"
  [task_time_s] -> Timer5/3(Ts)
  Constant36/1 -> Timer5/4(max_time)
  [VINP_BPPTGInsideSW1Sta_enum] -> Equal21/1, Detect Decrease14/1
  Constant42/1 -> Equal21/2
  Equal21/1 -> Logical Operator42/2
  Logical Operator42/1 -> [VDKC_PressSW1FallingEdge_flg]  "VDKC_PressSW1FallingEdge_flg"
  Detect Decrease14/1 -> Logical Operator42/1
  Constant43/1 -> Timer2/4(max_time)
  Relational Operator4/1 -> [VDKC_InnerSW2CloseTimeOut_flg]  "VDKC_InnerSW2CloseTimeOut_flg"
  Timer2/1(time) -> Relational Operator4/1
  [VINP_BPPTGInsideSW2Sta_enum] -> Equal16/1, Detect Increase5/1
  Constant37/1 -> Equal16/2
  Equal16/1 -> Logical Operator16/2
  Logical Operator16/1 -> [VDKC_PressSW2RisingEdge_flg]  "VDKC_PressSW2RisingEdge_flg"
  Detect Decrease/1 -> Logical Operator20/1
  Equal17/1 -> Logical Operator20/2
  Constant38/1 -> Equal17/2
  [VINP_BPPTGInsideSW2Sta_enum] -> Detect Decrease/1, Equal17/1
  Logical Operator20/1 -> [VDKC_PressSW2FallingEdge_flg]  "VDKC_PressSW2FallingEdge_flg"
  Detect Increase5/1 -> Logical Operator16/1
  Logical Operator33/1 -> Logical Operator22/1, Timer2/2(reset)
  Detect Increase3/1 -> Logical Operator18/1
  Logical Operator18/1 -> [VDKC_PressSW1RisingEdge_flg]  "VDKC_PressSW1RisingEdge_flg"
  Equal18/1 -> Logical Operator18/2
  Constant39/1 -> Equal18/2
  [VINP_BPPTGInsideSW1Sta_enum] -> Detect Increase3/1, Equal18/1
  Logical Operator22/1 -> Logical Operator21/2
  [VINP_TailgateSW_flg] -> Detect Decrease4/1
  Logical Operator24/1 -> [VDKC_PrsSW2TGFalEdgeInPS_flg]  "VDKC_PrsSW2TGFalEdgeInPS_flg"
  Constant47/1 -> Equal25/2
  [VDKC_UWBDetPSZoneKeepSta_enum] -> Equal25/1
  Logical Operator25/1 -> [VDKC_PrsSW2TGFalEdgeOutPS_flg]  "VDKC_PrsSW2TGFalEdgeOutPS_flg"
  [VINP_TailgateSW_flg] -> Detect Decrease3/1
  Logical Operator26/1 -> [VDKC_PrsSW2TGNoEdgeTimeOut_flg]  "VDKC_PrsSW2TGNoEdgeTimeOut_flg"
  Logical Operator21/1 -> Timer2/1(trigger), [VDKC_InnerSW2TimerLatch_flg]  "VDKC_InnerSW2TimerLatch_flg"
  [VDKC_PressSW2Latch_flg] -> Logical Operator25/1
  SR_Latch11/1(latched) -> Logical Operator21/1, [VDKC_PressSW2Latch_flg]  "VDKC_PressSW2Latch_flg"
  Constant41/1 -> Relational Operator4/2
  Detect Decrease4/1 -> Logical Operator24/2
  Detect Decrease3/1 -> Logical Operator25/2
  [VDKC_InnerSW2CloseTimeOut_flg] -> Detect Increase8/1
  [VINP_TailgateSW_flg] -> Logical Operator26/2
  [VDKC_TGFalEdgeInPS_flg] -> PTG_PCMD_Chart/5(VDKC_TGFalEdgeInPS_flg)
  [VDKC_DKCPCmdFallingEdge_flg] -> PTG_PCMD_Chart/10(VDKC_PCmdFallingEdge_flg)
  [VDKC_PrsSW2TGFalEdgeInPS_flg] -> PTG_PCMD_Chart/4(VDKC_PrsSW2TGFalEdgeInPS_flg)
  [task_time_s] -> PTG_PCMD_Chart/8(task_time_s)
  [VBCM_AntitheftSta_enum] -> PTG_PCMD_Chart/2(VBCM_AntitheftSta_enum)
  [VDKC_PrsSW2TGNoEdgeTimeOut_flg] -> PTG_PCMD_Chart/6(VDKC_PrsSW2TGNoEdgeTimeOut_flg)
  PTG_PCMD_Chart/2(VDKC_PTGPCmdHandingSta_enum) -> Data Type Conversion11/1
  PTG_PCMD_Chart/1(VDKC_PTGPCmdToBCMRAW_enum) -> Data Type Conversion10/1
  [VPMM_PowerSta_enum] -> PTG_PCMD_Chart/9(VPMM_PowerSta_enum)
  Data Type Conversion11/1 -> [VDKC_PTGPCmdHandSta_enum]  "VDKC_PTGPCmdHandSta_enum"
  Data Type Conversion10/1 -> [VDKC_PTGPCmdToBCMRAW_enum]  "VDKC_PTGPCmdToBCMRAW_enum"
  [VDKC_PressSW2Latch_flg] -> Logical Operator24/1
  [VDKC_PrsSW2TGFalEdgeOutPS_flg] -> PTG_PCMD_Chart/3(VDKC_PrsSW2TGFalEdgeOutPS_flg)
  [task_time_s] -> Timer2/3(Ts)
  [VDKC_FDCPCommandToBCM_enum] -> Unit Delay12/1
  Detect Change7/1 -> Logical Operator49/1
  Equal20/1 -> Logical Operator49/2
  Constant50/1 -> Equal20/2
  Constant28/1 -> Timer6/4(max_time)
  [task_time_s] -> Timer6/3(Ts)
  Relational Operator6/1 -> [VDKC_RemTGCmdCloseTimeOut_flg]  "VDKC_RemTGCmdCloseTimeOut_flg"
  Timer6/1(time) -> Relational Operator6/1
  Logical Operator34/1 -> Logical Operator47/1, Timer6/2(reset)
  Logical Operator47/1 -> Logical Operator46/2
  Logical Operator48/1 -> SR_Latch12/2(reset)
  Logical Operator46/1 -> Timer6/1(trigger), [VDKC_RemTGCmdTimerLatch_flg]  "VDKC_RemTGCmdTimerLatch_flg"
  SR_Latch12/1(latched) -> [VDKC_RemTGCmdFaillEdgeLatch_flg], Logical Operator46/1  "VDKC_RemTGCmdFaillEdgeLatch_flg"
  [VDKC_PrsSW2TGNoEdgeTimeOut_flg] -> Unit Delay13/1
  Constant49/1 -> Relational Operator6/2
  [VINP_TailgateSW_flg] -> Unit Delay14/1
  Logical Operator50/1 -> SR_Latch12/1(set)
  [VINP_TailgateSW_flg] -> Logical Operator52/2
  [VDKC_InnerSW1CloseTimeOut_flg] -> Detect Increase10/1
  Logical Operator52/1 -> [VDKC_PrsSW1orDKCNoEdgTimOut_flg]  "VDKC_PrsSW1orDKCNoEdgTimOut_flg"
  [VDKC_RemTGCmdCloseTimeOut_flg] -> Detect Increase11/1
  Detect Increase10/1 -> Logical Operator53/1
  Detect Increase11/1 -> Logical Operator53/2
  Logical Operator53/1 -> Logical Operator52/1
  Detect Decrease13/1 -> Logical Operator34/1, Logical Operator48/1
  Unit Delay13/1 -> Data Type Conversion103/1
  [VDKC_PrsSW1orDKCNoEdgTimOut_flg] -> Unit Delay23/1
  Unit Delay23/1 -> Data Type Conversion102/1
  [VDKC_PressSW2RisingEdge_flg] -> Logical Operator34/4, Logical Operator48/4
  [VDKC_PressSW1RisingEdge_flg] -> Logical Operator34/5, Logical Operator48/5
  Logical Operator49/1 -> Logical Operator34/6, Logical Operator48/6
  Logical Operator23/1 -> Logical Operator19/6, Logical Operator17/6
  [VDKC_PressSW1RisingEdge_flg] -> Logical Operator19/5, Logical Operator17/5
  [VDKC_PressSW2RisingEdge_flg] -> Logical Operator19/4, Logical Operator17/4
  Unit Delay6/1 -> Data Type Conversion105/1
  [VDKC_PrsSW1orDKCNoEdgTimOut_flg] -> Unit Delay6/1
  Unit Delay4/1 -> Data Type Conversion106/1
  Detect Decrease10/1 -> Logical Operator19/1, Logical Operator17/1
  [VINP_TailgateSW_flg] -> Unit Delay5/1
  [VDKC_PrsSW2TGNoEdgeTimeOut_flg] -> Unit Delay4/1
  Logical Operator19/1 -> SR_Latch8/2(reset)
  Constant40/1 -> Equal19/2
  Equal19/1 -> Logical Operator23/2
  Detect Change8/1 -> Logical Operator23/1
  [VDKC_FDCPCommandToBCM_enum] -> Unit Delay3/1
  [VDKC_FDCPCommandToBCM_enum] -> Unit Delay7/1
  Detect Change9/1 -> Logical Operator44/1
  Equal26/1 -> Logical Operator44/2
  Constant52/1 -> Equal26/2
  Logical Operator41/1 -> SR_Latch11/2(reset)
  [VDKC_PrsSW2TGNoEdgeTimeOut_flg] -> Unit Delay20/1
  [VINP_TailgateSW_flg] -> Unit Delay24/1
  Unit Delay24/1 -> Data Type Conversion109/1
  Detect Decrease11/1 -> Logical Operator33/1, Logical Operator41/1
  Unit Delay20/1 -> Data Type Conversion107/1
  [VDKC_PrsSW1orDKCNoEdgTimOut_flg] -> Unit Delay25/1
  Unit Delay25/1 -> Data Type Conversion108/1
  [VDKC_PressSW2RisingEdge_flg] -> Logical Operator33/4, Logical Operator41/4
  [VDKC_PressSW1RisingEdge_flg] -> Logical Operator33/5, Logical Operator41/5
  Logical Operator44/1 -> Logical Operator33/6, Logical Operator41/6
  [VDKC_PrsSW1orDKCNoEdgTimOut_flg] -> PTG_PCMD_Chart/7(VDKC_PrsSW1orDKCNoEdgTimOut_flg)
  [VINP_TailgateSW_flg] -> Unit Delay43/1
  Detect Decrease12/1 -> Logical Operator45/1
  Equal22/1 -> Logical Operator220/1
  Logical Operator51/1 -> SR_Latch11/1(set)
  [VDKC_PressSW2FallingEdge_flg] -> Logical Operator51/1
  [VINP_TailgateSW_flg] -> Logical Operator51/2
  [VINP_TailgateSW_flg] -> Logical Operator54/2
  [VDKC_PressSW1FallingEdge_flg] -> Logical Operator54/1
  Logical Operator54/1 -> SR_Latch8/1(set)
  [VDKC_PressSW1Latch_flg] -> Terminator/1
  [VDKC_RemTGCmdFaillEdgeLatch_flg] -> Terminator1/1
  [VINP_KeyFobAreaU16_enum] -> Extract Bits6/1
  Extract Bits6/1 -> Data Type Conversion73/1
  Data Type Conversion73/1 -> Switch13/2
  Constant85/1 -> Switch13/1
  Switch14/1 -> Switch13/3
  Switch16/1 -> Switch14/3
  Constant25/1 -> Switch14/1
  Data Type Conversion74/1 -> Switch14/2
  Extract Bits7/1 -> Data Type Conversion74/1
  [VINP_KeyFobAreaU16_enum] -> Extract Bits7/1
  [VINP_KeyFobAreaU16_enum] -> Extract Bits8/1
  Extract Bits8/1 -> Data Type Conversion75/1
  Data Type Conversion75/1 -> Switch16/2
  Constant88/1 -> Switch16/1
  Switch17/1 -> Switch16/3
  Constant87/1 -> Switch17/3
  Constant86/1 -> Switch17/1
  Data Type Conversion76/1 -> Switch17/2
  Extract Bits9/1 -> Data Type Conversion76/1
  [VINP_KeyFobAreaU16_enum] -> Extract Bits9/1
  Logical Operator112/1 -> Switch8/2
  Data Type Conversion7/1 -> Logical Operator112/1
  Extract Bits10/1 -> Data Type Conversion77/1
  [VINP_KeyFobAreaU16_enum] -> Extract Bits10/1
  Data Type Conversion77/1 -> Logical Operator112/2
  Constant89/1 -> Equal118/2
  Constant90/1 -> Equal119/2
  Constant180/1 -> Equal120/2
  Unit Delay28/1 -> Data Type Conversion79/1
  Data Type Conversion79/1 -> Equal119/1
  Data Type Conversion80/1 -> Equal120/1
  Unit Delay26/1 -> Data Type Conversion80/1
  Unit Delay27/1 -> Data Type Conversion78/1
  Data Type Conversion78/1 -> Equal118/1
  Unit Delay29/1 -> Data Type Conversion81/1
  Data Type Conversion81/1 -> Equal121/1
  Constant181/1 -> Equal121/2
  [VDKC_KeyUWBDetArea_enum] -> Unit Delay39/1, Unit Delay30/1, Unit Delay27/1, Unit Delay28/1, Unit Delay26/1, Unit Delay29/1, Equal70/1, Detect Change32/1
  Constant182/1 -> Equal122/2
  Unit Delay30/1 -> Data Type Conversion82/1
  Data Type Conversion82/1 -> Equal122/1
  Unit Delay31/1 -> Data Type Conversion83/1
  Data Type Conversion83/1 -> Equal123/1
  Equal123/1 -> Logical Operator81/3
  Constant183/1 -> Equal123/2
  [VDKC_KeyUWBDetArea_enum] -> Equal124/1, Detect Change35/1, Detect Change11/1, Equal69/1, Equal73/1, Detect Change33/1, Unit Delay31/1, Unit Delay19/1, Unit Delay21/1
  Constant184/1 -> Equal124/2
  Detect Change35/1 -> Logical Operator113/1
  Equal124/1 -> Logical Operator113/2
  Logical Operator113/1 -> Logical Operator85/3
  Logical Operator58/1 -> Logical Operator9/3
  Logical Operator6/1 -> Logical Operator127/2
  Data Type Conversion89/1 -> Equal114/1
  Unit Delay33/1 -> Data Type Conversion89/1
  Constant187/1 -> Equal114/2
  [VDKC_KeyUWBDetArea_enum] -> Detect Change38/1, Equal127/1, Unit Delay33/1, Unit Delay38/1
  Constant7/1 -> Equal125/2
  Logical Operator115/1 -> Logical Operator116/1
  Unit Delay38/1 -> Data Type Conversion67/1
  Data Type Conversion67/1 -> Equal125/1
  Constant131/1 -> Equal127/2
  Detect Change38/1 -> Logical Operator117/1
  Equal127/1 -> Logical Operator117/2
  Logical Operator117/1 -> Logical Operator116/2
  Logical Operator116/1 -> [VDKC_UWBDetAreaChgWelcome_flg]  "VDKC_UWBDetAreaChgWelcome_flg"
  Equal114/1 -> Logical Operator115/2
  Equal125/1 -> Logical Operator115/1
  [VDKC_UWBDetAreaChgWelcome_flg] -> SR_Latch13/1(set)
  [task_time_s] -> Timer7/3(Ts)
  Constant130/1 -> Timer7/4(max_time)
  SR_Latch13/1(latched) -> Switch37/2, Timer7/1(trigger), [VDKC_UWBDetChgWelcomeLatch_flg], Logical Operator118/1  "VDKC_UWBDetChgWelcomeLatch_flg"
  Logical Operator118/1 -> Timer7/2(reset)
  Switch37/1 -> VDKC_FDCKeyWelcomeSta_enum/1  "VDKC_FDCKeyWelcomeSta_enum"
  Constant185/1 -> Switch37/3
  Constant186/1 -> Switch37/1
  Constant188/1 -> Relational Operator7/2
  Timer7/1(time) -> Relational Operator7/1
  Relational Operator7/1 -> Unit Delay2/1
  Relational Operator8/1 -> Unit Delay8/1
  Unit Delay8/1 -> Data Type Conversion99/1
  Timer8/1(time) -> Relational Operator8/1
  Constant192/1 -> Relational Operator8/2
  Logical Operator119/1 -> Timer8/2(reset)
  SR_Latch14/1(latched) -> [VDKC_LidADetGreenCardLatch4s_flg], Logical Operator119/1, Timer8/1(trigger)  "VDKC_LidADetGreenCardLatch4s_flg"
  Constant189/1 -> Timer8/4(max_time)
  [task_time_s] -> Timer8/3(Ts)
  [VDKC_NFCLidARisingEdge_flg] -> SR_Latch14/1(set)
  Data Type Conversion88/1 -> Detect Change40/1, Equal137/1
  Equal137/1 -> Logical Operator50/2
  Constant224/1 -> Equal137/2
  Unit Delay44/1 -> Data Type Conversion88/1
  [VDKC_FDCPCommandToBCM_enum] -> Unit Delay15/1
  Unit Delay43/1 -> Data Type Conversion104/1
  Detect Change40/1 -> Logical Operator50/1
  Unit Delay15/1 -> Unit Delay44/1
  Switch55/1 -> Unit Delay45/1, [VDKC_UWBDetPEZoneKeepSta_enum]  "VDKC_UWBDetPEZoneKeepSta_enum"
  Constant228/1 -> Equal139/2
  [VDKC_KeyUWBDetArea_enum] -> Equal139/1
  Equal139/1 -> Switch55/2
  [VDKC_UWBDetPEZoneSta_enum] -> Switch55/1
  Switch56/1 -> Switch55/3
  [VDKC_BTConnectSta_enum] -> Equal29/1
  Constant51/1 -> Equal29/2
  Equal29/1 -> Switch56/2
  Constant227/1 -> Switch56/3
  Unit Delay45/1 -> Data Type Conversion98/1
  Unit Delay22/1 -> Data Type Conversion97/1
  Switch52/1 -> Unit Delay22/1, [VDKC_UWBDetPSZoneKeepSta_enum]  "VDKC_UWBDetPSZoneKeepSta_enum"
  Constant226/1 -> Switch53/3
  Equal138/1 -> Switch53/2
  Constant223/1 -> Equal138/2
  [VDKC_BTConnectSta_enum] -> Equal138/1
  Switch53/1 -> Switch52/3
  [VDKC_UWBDetPSZoneSta_enum] -> Switch52/1
  Equal23/1 -> Switch52/2
  [VDKC_KeyUWBDetArea_enum] -> Equal23/1
  Constant55/1 -> Equal23/2
  Switch54/1 -> [VDKC_BTConnectSta_enum]  "VDKC_BTConnectSta_enum"
  Constant230/1 -> Switch54/1
  Constant229/1 -> Switch54/2
  Constant235/1 -> Equal142/2
  [VPMM_PowerSta_enum] -> Equal142/1
  [VPMM_PowerSta_enum] -> Equal143/1
  Constant236/1 -> Equal143/2
  Equal142/1 -> Logical Operator131/1
  Equal143/1 -> Logical Operator131/2
  Constant237/1 -> Equal144/2
  [VPMM_PowerSta_enum] -> Equal144/1
  Equal144/1 -> Logical Operator131/3
  Logical Operator132/1 -> Switch61/2
  Logical Operator131/1 -> Logical Operator132/2
  [VINP_BrakeSWSta_flg] -> Logical Operator132/1
  Constant238/1 -> Data Type Conversion95/1
  [VDKC_FDCKeyAreaPS_enum] -> Equal146/1
  Constant241/1 -> Equal146/2
  Equal146/1 -> Switch60/2
  Switch62/1 -> Switch60/3
  [task_time_s] -> Timer9/3(Ts)
  Constant239/1 -> Timer9/4(max_time)
  SR_Latch17/1(latched) -> [VDKC_BTDisconDebLatch_flg], Timer9/1(trigger), Logical Operator133/1  "VDKC_BTDisconDebLatch_flg"
  Constant240/1 -> Relational Operator9/2
  Timer9/1(time) -> Relational Operator9/1
  Relational Operator9/1 -> SR_Latch18/1(set), Unit Delay49/1
  Equal145/1 -> Logical Operator135/2
  Constant243/1 -> Equal145/2
  [VDKC_BTConnectSta_enum] -> Detect Decrease16/1, Equal145/1
  Detect Decrease16/1 -> Logical Operator135/1
  Logical Operator135/1 -> SR_Latch17/1(set)
  [VPMM_PowerSta_enum] -> Equal147/1
  Constant244/1 -> Equal147/2
  Equal147/1 -> Logical Operator135/3
  Logical Operator137/1 -> SR_Latch18/2(reset)
  [VDKC_PMMEnterOFFA_flg] -> Logical Operator137/2
  [VDKC_PMMEnterOFF_flg] -> Logical Operator137/1
  [VDKC_PMMEnterOFFC_flg] -> Logical Operator137/3
  [VDKC_OnReadyKeyMissLatch_flg] -> Switch62/2
  SR_Latch18/1(latched) -> [VDKC_OnReadyKeyMissLatch_flg]  "VDKC_OnReadyKeyMissLatch_flg"
  Switch61/1 -> Switch62/3
  Constant245/1 -> Data Type Conversion94/1
  [VDKC_FDCKeyAreaPS_enum] -> Unit Delay50/1
  Equal141/1 -> Logical Operator134/2
  Constant246/1 -> Equal141/2
  Detect Change15/1 -> Logical Operator134/1
  Logical Operator134/1 -> Logical Operator137/4
  [VDKC_BTDisconDebLatch_flg] -> Logical Operator129/3
  Constant248/1 -> Switch63/2
  Constant249/1 -> Switch63/1
  Switch63/1 -> [VDKC_UIDBatVoltx1000_V]  "VDKC_UIDBatVoltx1000_V"
  Switch64/1 -> VDKC_UIDLowPowerSta_flg/1  "VDKC_UIDLowPowerSta_flg"
  Logical Operator136/1 -> Switch64/2
  Constant250/1 -> Equal148/2
  [VPMM_PowerSta_enum] -> Equal148/1
  Equal148/1 -> Logical Operator136/2
  Constant251/1 -> Equal149/2
  [VDKC_BTConnectSta_enum] -> Equal149/1
  Equal149/1 -> Logical Operator136/1
  Switch65/1 -> Switch64/1
  [VDKC_UIDBatVoltx1000_V] -> PDkeyJudgeBatLowVolt_Chart/1(VDKC_UIDBatVoltx1000_V)
  Constant255/1 -> PDkeyJudgeBatLowVolt_Chart/4(KDKC_UIDBatLowVolDeb_cnt)
  Constant256/1 -> PDkeyJudgeBatLowVolt_Chart/5(KDKC_UIDBatOKVolDeb_cnt)
  Constant257/1 -> PDkeyJudgeBatLowVolt_Chart/6(KDKC_UIDBatSampInterval_s)
  [task_time_s] -> PDkeyJudgeBatLowVolt_Chart/9(task_time_s)
  Constant258/1 -> PDkeyJudgeBatLowVolt_Chart/7(KDKC_UIDBatSampTotal_cnt)
  Constant259/1 -> PDkeyJudgeBatLowVolt_Chart/2(KDKC_UIDBatLowVolx1000Thres_V)
  Constant260/1 -> PDkeyJudgeBatLowVolt_Chart/3(KDKC_UIDBatOKVolx1000Thres_V)
  [VDKC_BTConnectSta_enum] -> PDkeyJudgeBatLowVolt_Chart/8(VDKC_BTConnectSta_enum)
  Constant254/1 -> Data Type Conversion90/1
  Constant252/1 -> Data Type Conversion96/1
  Data Type Conversion92/1 -> Switch60/1
  Constant242/1 -> Data Type Conversion92/1
  Data Type Conversion93/1 -> Switch62/1
  Constant233/1 -> Data Type Conversion93/1
  Data Type Conversion94/1 -> Switch61/1
  Data Type Conversion95/1 -> Switch61/3
  Constant261/1 -> Equal150/2
  Equal150/1 -> Logical Operator141/2
  Detect Change41/1 -> Logical Operator141/1
  [VDKC_TrunkHanPCmdToBCMRAW_enum] -> Detect Change43/1, Equal153/1
  Detect Change43/1 -> Logical Operator143/1
  Equal153/1 -> Logical Operator143/2
  Constant264/1 -> Equal153/2
  Constant265/1 -> Equal154/2
  Equal154/1 -> Logical Operator144/2
  Detect Change44/1 -> Logical Operator144/1
  Logical Operator144/1 -> Logical Operator142/3
  Logical Operator143/1 -> Logical Operator142/2
  Logical Operator142/1 -> Switch66/2
  Switch67/1 -> Switch66/3
  [VDKC_UWBDetPCmdToBCMRAW_enum] -> Equal154/1, Detect Change44/1
  [VDKC_UIDButtonPCmdToBCMRAW_enum] -> Equal150/1, Detect Change41/1
  Switch66/1 -> Switch68/3
  Switch68/1 -> Unit Delay51/1, VDKC_KeyTypeSta_enum/1  "VDKC_KeyTypeSta_enum"
  [VDKC_FDCKeyAllowSleep_flg] -> Detect Increase13/1
  Detect Increase13/1 -> Switch68/2
  Constant266/1 -> Switch68/1
  Constant267/1 -> Switch66/1
  Constant269/1 -> Equal156/2
  [VDKC_UWBDetPSZoneKeepSta_enum] -> Equal156/1, Detect Change45/1
  Logical Operator141/1 -> Logical Operator142/1
  Logical Operator145/1 -> Logical Operator142/4
  Equal156/1 -> Logical Operator145/2
  Detect Change45/1 -> Logical Operator145/1
  Constant270/1 -> Switch67/1
  Detect Change47/1 -> Logical Operator148/1
  Equal158/1 -> Logical Operator148/2
  Logical Operator148/1 -> Logical Operator146/2
  [VDKC_NFCJudgePSZoneSta_enum] -> Detect Change47/1, Equal158/1
  Constant272/1 -> Equal158/2
  [VDKC_NFCDetPCmdToBCMRAW_enum] -> Detect Change46/1, Equal157/1
  Logical Operator147/1 -> Logical Operator146/1
  Detect Change46/1 -> Logical Operator147/1
  Equal157/1 -> Logical Operator147/2
  Constant271/1 -> Equal157/2
  Logical Operator146/1 -> Switch67/2
  Unit Delay51/1 -> Data Type Conversion65/1
  Data Type Conversion65/1 -> Switch67/3
  Data Type Conversion97/1 -> Switch53/1
  Data Type Conversion98/1 -> Switch56/1
  Data Type Conversion99/1 -> SR_Latch14/2(reset)
  Unit Delay49/1 -> Data Type Conversion100/1
  Data Type Conversion100/1 -> Logical Operator138/2
  Unit Delay50/1 -> Data Type Conversion101/1
  Data Type Conversion101/1 -> Equal141/1, Detect Change15/1
  Data Type Conversion102/1 -> Logical Operator34/3, Logical Operator48/3
  Data Type Conversion103/1 -> Logical Operator34/2, Logical Operator48/2
  Data Type Conversion104/1 -> Logical Operator50/3
  Data Type Conversion105/1 -> Logical Operator19/3, Logical Operator17/3
  Data Type Conversion106/1 -> Logical Operator19/2, Logical Operator17/2
  Data Type Conversion107/1 -> Logical Operator33/2, Logical Operator41/2
  Data Type Conversion108/1 -> Logical Operator33/3, Logical Operator41/3
  Data Type Conversion109/1 -> Detect Decrease11/1
  Unit Delay5/1 -> Data Type Conversion110/1
  Data Type Conversion110/1 -> Detect Decrease10/1
  Data Type Conversion111/1 -> Detect Decrease13/1
  Unit Delay14/1 -> Data Type Conversion111/1
  Data Type Conversion112/1 -> Logical Operator76/2
  Data Type Conversion113/1 -> Logical Operator9/2
  Unit Delay34/1 -> Data Type Conversion114/1
  Data Type Conversion114/1 -> Logical Operator107/2
  Unit Delay2/1 -> Data Type Conversion115/1
  Data Type Conversion115/1 -> SR_Latch13/2(reset)
  [VDKC_UIDButtonPCmdToBCMRAW_enum] -> Equal155/1
  Constant274/1 -> Equal155/2
  Equal155/1 -> Switch69/2
  Constant273/1 -> Switch69/1
  Switch70/1 -> Switch69/3
  Constant277/1 -> Equal159/2
  [VDKC_TrunkHanPCmdToBCMRAW_enum] -> Equal159/1
  Equal159/1 -> Switch70/2
  Constant276/1 -> Switch70/1
  Switch71/1 -> Switch70/3
  Constant278/1 -> Switch71/1
  [VDKC_NFCDetPCmdToBCMRAW_enum] -> Equal160/1
  Constant279/1 -> Equal160/2
  Constant281/1 -> Equal161/2
  [VDKC_PTGPCmdToBCMRAW_enum] -> Equal161/1
  Equal161/1 -> Switch72/2
  Constant280/1 -> Switch72/1
  Switch72/1 -> Switch71/3
  Constant282/1 -> Switch73/1
  Equal162/1 -> Switch73/2
  [VDKC_AutoLockPCmdToBCMRAW_enum] -> Equal162/1
  Constant283/1 -> Equal162/2
  Switch73/1 -> Switch72/3
  Constant285/1 -> Equal163/2
  [VDKC_UWBDetPCmdToBCMRAW_enum] -> Equal163/1
  Constant284/1 -> Switch74/1
  Switch74/1 -> Switch73/3
  Constant286/1 -> Switch74/3
  Switch69/1 -> VDKC_KeyModeSta_enum/1  "VDKC_KeyModeSta_enum"
  Equal160/1 -> Logical Operator151/1
  Detect Increase14/1 -> Logical Operator151/2
  Logical Operator151/1 -> Switch71/2
  [VDKC_NFCLidARisingEdge_flg] -> Detect Increase14/1
  Detect Change48/1 -> Logical Operator149/1
  Equal165/1 -> Logical Operator149/2
  [VDKC_UWBDetPSZoneSta_enum] -> Detect Change48/1, Equal165/1
  Constant268/1 -> Equal165/2
  Logical Operator150/1 -> Switch74/2
  Equal163/1 -> Logical Operator150/1
  Logical Operator149/1 -> Logical Operator150/2
  [VDKC_DrDoorOpenStaLatch4s_flg] -> Logical Operator155/1
  SR_Latch16/1(latched) -> Logical Operator155/2
  Logical Operator155/1 -> Switch48/2
  Equal152/1 -> Logical Operator139/2
  Equal7/1 -> Logical Operator139/1
  Logical Operator139/1 -> Switch39/2
  Constant263/1 -> Equal152/2
  [VPMM_PowerSta_enum] -> Equal152/1
  Switch48/1 -> Switch40/3
  Constant194/1 -> Switch40/1
  [VINP_BrakeSWFallingEdge_flg] -> SR_Latch15/1(set)
  SR_Latch15/1(latched) -> Switch40/2
  Switch40/1 -> Switch39/3
  Constant193/1 -> Switch39/1
  Constant191/1 -> Equal7/2
  [VDKC_FDCKeyAreaPS_enum] -> Equal7/1
  Switch38/1 -> VDKC_DkeyShowIVISta_enum/1  "VDKC_DkeyShowIVISta_enum"
  Constant190/1 -> Switch38/1
  [VDKC_LidADetGreenCardLatch4s_flg] -> Switch38/2
  Constant209/1 -> Equal126/2
  [VDKC_NFCDetPCmdToBCMRAW_enum] -> Equal126/1
  Equal126/1 -> Logical Operator120/1
  Constant208/1 -> Equal128/2
  [VBCM_AntitheftSta_enum] -> Equal128/1, Detect Change36/1
  Equal128/1 -> Logical Operator120/3
  Detect Change36/1 -> Logical Operator120/2
  Logical Operator120/1 -> SR_Latch16/1(set)
  [VDKC_FDCKeyAreaPS_enum] -> Equal129/1
  Constant210/1 -> Equal129/2
  Logical Operator121/1 -> SR_Latch16/2(reset)
  [VBCM_AntitheftSta_enum] -> Detect Change37/1, Equal131/1
  Constant213/1 -> Equal131/2
  Logical Operator122/1 -> Logical Operator121/2
  Equal131/1 -> Logical Operator122/2
  Detect Change37/1 -> Logical Operator122/1
  Equal129/1 -> Logical Operator121/1
  Constant214/1 -> Switch48/1
  Switch39/1 -> Switch38/3
  Constant215/1 -> Switch48/3
  Equal11/1 -> Logical Operator59/1
  Detect Change39/1 -> Logical Operator123/1
  Equal57/1 -> Logical Operator123/2
  Logical Operator123/1 -> Logical Operator59/2
  Constant195/1 -> Equal57/2
  [VBCM_AntitheftSta_enum] -> Equal57/1, Detect Change39/1
  Constant81/1 -> Equal11/2
  [VDKC_FDCKeyAreaPS_enum] -> Equal11/1
  Logical Operator59/1 -> SR_Latch15/2(reset)
  [VINP_SeatSW_flg] -> Logical Operator154/1
  Logical Operator154/1 -> Logical Operator153/2
  Logical Operator153/1 -> SR_Latch19/1(set)
  Detect Increase15/1 -> Logical Operator153/1
  [VINP_DrDoorSW_flg] -> Detect Increase15/1
  Relational Operator10/1 -> Unit Delay52/1
  Unit Delay52/1 -> Data Type Conversion116/1
  Timer10/1(time) -> Relational Operator10/1
  Constant287/1 -> Relational Operator10/2
  Logical Operator152/1 -> Timer10/2(reset)
  SR_Latch19/1(latched) -> [VDKC_DrDoorOpenStaLatch4s_flg], Logical Operator152/1, Timer10/1(trigger)  "VDKC_DrDoorOpenStaLatch4s_flg"
  Constant275/1 -> Timer10/4(max_time)
  [task_time_s] -> Timer10/3(Ts)
  Data Type Conversion116/1 -> SR_Latch19/2(reset)
  [VDKC_DrDoorOpenStaLatch4s_flg] -> Logical Operator129/4
  Constant289/1 -> Switch75/2
  Constant290/1 -> Switch75/1
  Switch75/1 -> [VDKC_DKCBTRSSI_dB]  "VDKC_DKCBTRSSI_dB"
  VINP_BrakeSWGPIO_flg/1 -> Detect Decrease15/1, [VINP_BrakeSWSta_flg]
  VINP_SeatSW_flg/1 -> [VINP_SeatSW_flg]
  [VDKC_DKCBTRSSI_dB] -> BTRSSIJudgeArea_Chart/1(VDKC_DKCBTRSSI_dB)
  Constant296/1 -> BTRSSIJudgeArea_Chart/4(KDKC_JudBTRSSIWeakDeb_cnt)
  Constant297/1 -> BTRSSIJudgeArea_Chart/5(KDKC_JudBTRSSIStrongDeb_cnt)
  Constant298/1 -> BTRSSIJudgeArea_Chart/6(KDKC_BTRSSISampTime_s)
  [task_time_s] -> BTRSSIJudgeArea_Chart/9(task_time_s)
  Constant300/1 -> BTRSSIJudgeArea_Chart/2(KDKC_JudBTRSSIWeakThres_dB)
  Constant301/1 -> BTRSSIJudgeArea_Chart/3(KDKC_JudBTRSSIStrongThres_dB)
  [VDKC_BTConnectSta_enum] -> BTRSSIJudgeArea_Chart/7(VDKC_BTConnectSta_enum)
  Detect Decrease15/1 -> [VINP_BrakeSWFallingEdge_flg]  "VINP_BrakeSWFallingEdge_flg"
  [VDKC_KeyUWBDetArea_enum] -> BTRSSIJudgeArea_Chart/8(VDKC_KeyUWBDetArea_enum)
  BTRSSIJudgeArea_Chart/1(VDKC_RSSIJudgeArea_enum) -> [VDKC_RSSIJudgeArea_enum]  "VDKC_RSSIJudgeArea_enum"
  Logical Operator156/1 -> [VDKC_UIDDetRSSIChgToLock_flg]  "VDKC_UIDDetRSSIChgToLock_flg"
  Equal164/1 -> Logical Operator156/2
  Detect Decrease18/1 -> Logical Operator156/1
  [VDKC_RSSIJudgeArea_enum] -> Equal164/1, Detect Decrease18/1
  Constant291/1 -> Equal164/2
  [VINP_SeatSW_flg] -> UWB_PCMD_Chart/11(VINP_SeatSW_flg)
  Constant292/1 -> Switch76/2
  Constant293/1 -> Data Type Conversion118/1
  Data Type Conversion118/1 -> Switch76/3
  Switch76/1 -> Switch63/3
  Constant/1 -> Switch77/3
  Constant247/1 -> Switch77/2
  Switch77/1 -> Switch54/3
  Data Type Conversion62/1 -> Switch78/3
  Constant294/1 -> Switch78/2
  Constant295/1 -> Data Type Conversion62/1
  Switch78/1 -> Switch75/3
  Constant302/1 -> Switch80/2
  Constant303/1 -> Switch80/3
  Constant299/1 -> Detect Increase12/1
  Data Type Conversion119/1 -> Switch81/2
  Detect Increase12/1 -> Data Type Conversion119/1
  Switch81/1 -> Switch80/1
  [VDKC_KeyUWBDetArea_enum] -> Equal169/1, Detect Decrease20/1, Unit Delay/1
  Logical Operator160/1 -> Logical Operator157/2
  Detect Decrease20/1 -> Logical Operator160/1
  Unit Delay/1 -> Equal167/1
  Constant305/1 -> Equal167/2
  Equal167/1 -> Logical Operator157/1
  Data Type Conversion120/1 -> Switch81/3
  Logical Operator157/1 -> Data Type Conversion120/1  "VDKC_UnlockZoneFallEdge_flg"
  Switch80/1 -> [VDKC_StoreUnlockAreaEdge_flg]  "VDKC_StoreUnlockAreaEdge_flg"
  [VDKC_StoreUnlockAreaEdge_flg] -> SR_Latch20/1(set)
  SR_Latch20/1(latched) -> VDKC_JudgeKeepUnlockZone_flg/1, Logical Operator158/1  "VDKC_JudgeKeepUnlockZone_flg"
  Logical Operator158/1 -> Logical Operator159/1
  Constant316/1 -> Equal184/2
  Data Type Conversion128/1 -> Equal182/1
  Unit Delay67/1 -> Data Type Conversion128/1
  Constant314/1 -> Equal182/2
  Detect Change49/1 -> Logical Operator164/2
  Equal184/1 -> Logical Operator164/3
  Equal182/1 -> Logical Operator164/1
  Constant288/1 -> Equal169/2
  Equal169/1 -> Logical Operator160/2
  Constant304/1 -> Equal166/2
  Equal166/1 -> Logical Operator161/2
  Equal168/1 -> Logical Operator161/1
  [VDKC_KeyUWBDetArea_enum] -> Equal170/1, Equal166/1, Equal168/1
  Constant306/1 -> Equal168/2
  Logical Operator161/1 -> SR_Latch20/2(reset)
  Constant307/1 -> Switch79/2
  Switch79/1 -> VDKC_KeyMissSta_flg/1  "VDKC_KeyMissSta_flg"
  Switch82/1 -> [VDKC_UnavToUnlReqUnlock_flg]  "VDKC_UnavToUnlReqUnlock_flg"
  Logical Operator159/1 -> Switch82/1  "VDKC_UnavToUnlReq_flg"
  Constant309/1 -> Switch82/2
  Constant310/1 -> Switch82/3
  Constant311/1 -> Data Type Conversion117/1
  Data Type Conversion117/1 -> Switch79/3
  Switch60/1 -> Switch79/1  "VDKC_JudgKeyMissSta_flg"
  VINP_FlashJugKeepUnLZone_flg/1 -> Switch81/1
  Equal118/1 -> Logical Operator77/3
  Equal119/1 -> Logical Operator77/4
  Equal120/1 -> Logical Operator77/5
  Equal121/1 -> Logical Operator77/6
  Constant308/1 -> Equal170/2
  Equal170/1 -> Logical Operator161/3
  Equal171/1 -> Logical Operator162/1
  Equal172/1 -> Logical Operator162/3
  Detect Change6/1 -> Logical Operator162/2
  [VDKC_KeyUWBDetArea_enum] -> Unit Delay53/1, Detect Change6/1, Equal172/1, Equal184/1, Detect Change49/1, Unit Delay67/1
  Constant315/1 -> Equal171/2
  Unit Delay53/1 -> Data Type Conversion121/1
  Data Type Conversion121/1 -> Equal171/1
  Constant313/1 -> Equal172/2
  Logical Operator164/1 -> Logical Operator163/1  "VDKC_UnavChgToUnlockZone_flg"
  Logical Operator163/1 -> Logical Operator159/2  "VDKC_UnORGrChgToUnlZone_flg"
  Logical Operator162/1 -> Logical Operator163/2  "VDKC_GrayChgToUnlockZone_flg"
  [VDKC_NFCDoorRisingEdge_flg] -> Logical Operator107/3
  Logical Operator165/1 -> Detect Increase6/1
  Equal32/1 -> Logical Operator165/1
  Constant312/1 -> Equal173/2
  [VDKC_AutoLockPCmdToBCMRAW_enum] -> Equal173/1
  Equal173/1 -> Logical Operator166/1
  [VDKC_NFCDetJudgeAutoLock_flg] -> Logical Operator166/2
  Logical Operator166/1 -> Logical Operator165/2
  [VDKC_NFCDetJudgeAutoLock_flg] -> Logical Operator167/2
  Equal174/1 -> Logical Operator167/1
  [VDKC_AutoLockPCmdToBCMRAW_enum] -> Equal174/1
  Constant317/1 -> Equal174/2
  Logical Operator167/1 -> Logical Operator107/4
  Detect Increase16/1 -> Switch23/2
  Constant253/1 -> Data Type Conversion91/1
  Data Type Conversion90/1 -> Switch65/1
  Data Type Conversion91/1 -> Switch65/3
  Data Type Conversion96/1 -> Switch64/3
  VINP_BPPTGExistSta_flg/1 -> Terminator3/1
  Switch83/1 -> TrunkHanSW_PCMD_Chart/3(VDKC_TrunkHanSW_flg)
  [VDKC_TrunkHandleSW_flg] -> Switch83/1
  Constant318/1 -> Switch83/3
  Constant319/1 -> Switch84/3
  [VDKC_UIDButtonRemTailGate_flg] -> Switch84/1
  Constant18/1 -> Switch85/1
  Switch85/1 -> Switch2/1
  Constant320/1 -> Switch85/3
